simulink model "Robust_joint_Space"  (R2020b)
settings: Solver=VariableStepAuto  StartTime=0.0  StopTime=10  RelTol=1e-3
(part 5 of 7)

== matlab function Robust_joint_Space/robust inverse dynamic controller/v_hat_prod ==
  data: m input; theta input; Vhat output; thetad input
function Vhat = Find_V(m,theta,thetad)

m1 = m(1);
m2 = m(2);
m3 = m(3);
m4 = m(4);
m5 = m(5);
m6 = m(6);

t1=theta(1);
t2=theta(2);
t3=theta(3);
t4=theta(4);
t5=theta(5);
t6=theta(6);

td1=thetad(1);
td2=thetad(2);
td3=thetad(3);
td4=thetad(4);
td5=thetad(5);
td6=thetad(6);

L1=0.1025;
L2=0.408;
L3=0.376;
L4=0.1025; 
L5=0.1025;

Vhat = [td2*(td2*(0.1046752610416666598360663220646*cos(t1)*sin(t1) - 0.10662220333333332668301896006824*cos(t1)*cos(t2)^2*sin(t1) + 0.0058654583333333336347958919532175*cos(t1)*cos(t3)^2*sin(t1) - 0.0029327291666666668173979459766088*cos(t1)^2*cos(t3)*sin(t3) + 0.0029327291666666668173979459766088*cos(t3)*sin(t1)^2*sin(t3) + 19740.25*m2*cos(t1)*sin(t1) - 0.25*L2^2*m2*cos(t1)*sin(t1) - 70.25*L2*m2*cos(t1)^2*sin(t2) + 70.25*L2*m2*sin(t1)^2*sin(t2) + 0.25*L2^2*m2*cos(t1)*cos(t2)^2*sin(t1)) - 1.0*td5*(0.00036659114583333335217474324707609*sin(3.0*t2 - 1.0*t1 + t3 + t4) + 0.00073318229166666670434948649415219*sin(t2 - 2.0*t1 + 3.0*t3 + t4) + 0.00018329557291666667608737162353805*sin(3.0*t2 - 2.0*t1 + t3 + t4) + 0.00018329557291666667608737162353805*sin(2.0*t1 + 3.0*t2 + t3 + t4) + 0.00073318229166666670434948649415219*sin(t2 + t3 + t4) + 0.00036659114583333335217474324707609*sin(t1 - 1.0*t2 + t3 + t4) - 0.00057664973958333336527190549070099*sin(t2 - 2.0*t1 + t3 + t4) - 0.00057664973958333336527190549070099*sin(2.0*t1 + t2 + t3 + t4) + 0.00036659114583333335217474324707609*sin(t1 + 3.0*t2 + t3 + t4) - 0.00018329557291666667608737162353805*sin(2.0*t1 + t2 - 1.0*t3 - 1.0*t4) + 0.00036659114583333335217474324707609*sin(t3 - 1.0*t2 + t4) - 0.00036659114583333335217474324707609*sin(t1 + t2 - 1.0*t3 - 1.0*t4) + 0.00073318229166666670434948649415219*sin(2.0*t1 + t2 - 1.0*t3 + t4) + 0.00018329557291666667608737162353805*sin(2.0*t1 - 1.0*t2 + t3 + t4) - 0.0010997734375000000565242297412283*sin(3.0*t2 + t3 + t4) + 94.0*L3*m5*sin(t2 + t3 + t5) - 25.625*L3*m5*sin(t2 + t3 + t4 - 1.0*t5) - 102.0*L3*m5*sin(t2 - 1.0*t5) + 0.125*L3^2*m5*sin(t2 + t3 + t4) - 0.0625*L3^2*m5*sin(t2 + t3 + t4 - 2.0*t5) - 0.0625*L3^2*m5*sin(t2 + t3 + t4 + 2.0*t5) + 25.625*L3*m5*sin(t2 + t3 + t4 + t5) + 102.0*L3*m5*sin(t2 + t5) - 94.0*L3*m5*sin(t2 + t3 - 1.0*t5) - 0.25*L3*L4*m5*sin(t2 + t3 + t4 + t5) + 0.25*L3*L4*m5*sin(t2 + t3 + t4 - 1.0*t5)) - 1.0*td6*(0.00084023437500000005238864897449957*cos(t1)*cos(t5)*sin(t1) + 0.00042011718750000002619432448724979*cos(t1)^2*cos(t2)*cos(t3)*cos(t4)*sin(t5) - 0.00042011718750000002619432448724979*cos(t2)*cos(t3)*cos(t4)*sin(t1)^2*sin(t5) - 0.00042011718750000002619432448724979*cos(t1)^2*cos(t2)*sin(t3)*sin(t4)*sin(t5) - 0.00042011718750000002619432448724979*cos(t1)^2*cos(t3)*sin(t2)*sin(t4)*sin(t5) - 0.00042011718750000002619432448724979*cos(t1)^2*cos(t4)*sin(t2)*sin(t3)*sin(t5) + 0.00042011718750000002619432448724979*cos(t2)*sin(t1)^2*sin(t3)*sin(t4)*sin(t5) + 0.00042011718750000002619432448724979*cos(t3)*sin(t1)^2*sin(t2)*sin(t4)*sin(t5) + 0.00042011718750000002619432448724979*cos(t4)*sin(t1)^2*sin(t2)*sin(t3)*sin(t5)) + td4*(0.00073318229166666670434948649415219*sin(t1 - 2.0*t2) + 0.00073318229166666670434948649415219*sin(t1 + 2.0*t2) - 0.001153299479166666730543810981402*sin(2.0*t1) + 0.00036659114583333335217474324707609*sin(2.0*t1 - 2.0*t2) + 0.00036659114583333335217474324707609*sin(2.0*t1 + 2.0*t2) + 0.0014663645833333334086989729883044*sin(2.0*t1 - 2.0*t3)) + td3*(0.00073318229166666670434948649415219*sin(t1 - 2.0*t2) + 0.00073318229166666670434948649415219*sin(t1 + 2.0*t2) - 0.00024028885416666671912683250766918*sin(2.0*t1) + 0.00036659114583333335217474324707609*sin(2.0*t1 - 2.0*t2) + 0.00036659114583333335217474324707609*sin(2.0*t1 + 2.0*t2) + 0.0014663645833333334086989729883044*sin(2.0*t1 - 2.0*t3)) + td1*(153408.0*m4*sin(2.0*t2 + t3) - 0.053311101666666663341509480034119*sin(2.0*t2) + 153408.0*m5*sin(2.0*t2 + t3) + 153408.0*m6*sin(2.0*t2 + t3) + 38540.0*m5*sin(2.0*t2 + 2.0*t3 + t4) + 38540.0*m6*sin(2.0*t2 + 2.0*t3 + t4) + 83232.0*m3*sin(2.0*t2) + 83232.0*m4*sin(2.0*t2) + 83232.0*m5*sin(2.0*t2) + 83232.0*m6*sin(2.0*t2) + 41820.0*m5*sin(2.0*t2 + t3 + t4) + 41820.0*m6*sin(2.0*t2 + t3 + t4) + 70688.0*m4*sin(2.0*t2 + 2.0*t3) + 70688.0*m5*sin(2.0*t2 + 2.0*t3) + 70688.0*m6*sin(2.0*t2 + 2.0*t3) + 5253.125*m5*sin(2.0*t2 + 2.0*t3 + 2.0*t4) + 5253.125*m6*sin(2.0*t2 + 2.0*t3 + 2.0*t4) - 102.5*L4*m5*sin(2.0*t2 + 2.0*t3 + 2.0*t4) + 25.625*L3*m5*sin(2.0*t2 + 2.0*t3 + 2.0*t4 - 1.0*t5) - 102.0*L3*m5*sin(2.0*t2 + t3 + t4 + t5) - 0.0625*L3^2*m5*sin(2.0*t2 + 2.0*t3 + 2.0*t4) + 0.5*L4^2*m5*sin(2.0*t2 + 2.0*t3 + 2.0*t4) - 376.0*L4*m5*sin(2.0*t2 + 2.0*t3 + t4) + 0.03125*L3^2*m5*sin(2.0*t2 + 2.0*t3 + 2.0*t4 - 2.0*t5) + 0.03125*L3^2*m5*sin(2.0*t2 + 2.0*t3 + 2.0*t4 + 2.0*t5) + 94.0*L3*m5*sin(2.0*t2 + 2.0*t3 + t4 - 1.0*t5) - 25.625*L3*m5*sin(2.0*t2 + 2.0*t3 + 2.0*t4 + t5) - 408.0*L4*m5*sin(2.0*t2 + t3 + t4) + 102.0*L3*m5*sin(2.0*t2 + t3 + t4 - 1.0*t5) - 94.0*L3*m5*sin(2.0*t2 + 2.0*t3 + t4 + t5) + 0.125*L2^2*m2*sin(2.0*t2) - 0.25*L3*L4*m5*sin(2.0*t2 + 2.0*t3 + 2.0*t4 - 1.0*t5) + 0.25*L3*L4*m5*sin(2.0*t2 + 2.0*t3 + 2.0*t4 + t5))) - td6*(td6*(0.5*(0.00084023437500000005238864897449957*cos(t1)*cos(t5) - 0.00084023437500000005238864897449957*cos(t2)*cos(t3)*cos(t4)*sin(t1)*sin(t5) + 0.00084023437500000005238864897449957*cos(t2)*sin(t1)*sin(t3)*sin(t4)*sin(t5) + 0.00084023437500000005238864897449957*cos(t3)*sin(t1)*sin(t2)*sin(t4)*sin(t5) + 0.00084023437500000005238864897449957*cos(t4)*sin(t1)*sin(t2)*sin(t3)*sin(t5))*(cos(t1)*cos(t2)*sin(t3)*sin(t4)*sin(t5) - 1.0*cos(t1)*cos(t2)*cos(t3)*cos(t4)*sin(t5) - 1.0*cos(t5)*sin(t1) + cos(t1)*cos(t3)*sin(t2)*sin(t4)*sin(t5) + cos(t1)*cos(t4)*sin(t2)*sin(t3)*sin(t5)) - 0.5*(0.0016804687500000001047772979489991*cos(t1)*cos(t5) - 0.0016804687500000001047772979489991*cos(t2)*cos(t3)*cos(t4)*sin(t1)*sin(t5) + 0.0016804687500000001047772979489991*cos(t2)*sin(t1)*sin(t3)*sin(t4)*sin(t5) + 0.0016804687500000001047772979489991*cos(t3)*sin(t1)*sin(t2)*sin(t4)*sin(t5) + 0.0016804687500000001047772979489991*cos(t4)*sin(t1)*sin(t2)*sin(t3)*sin(t5))*(cos(t1)*cos(t2)*sin(t3)*sin(t4)*sin(t5) - 1.0*cos(t1)*cos(t2)*cos(t3)*cos(t4)*sin(t5) - 1.0*cos(t5)*sin(t1) + cos(t1)*cos(t3)*sin(t2)*sin(t4)*sin(t5) + cos(t1)*cos(t4)*sin(t2)*sin(t3)*sin(t5)) + 0.5*(0.00084023437500000005238864897449957*cos(t1)*cos(t2)*sin(t3)*sin(t4)*sin(t5) - 0.00084023437500000005238864897449957*cos(t1)*cos(t2)*cos(t3)*cos(t4)*sin(t5) - 0.00084023437500000005238864897449957*cos(t5)*sin(t1) + 0.00084023437500000005238864897449957*cos(t1)*cos(t3)*sin(t2)*sin(t4)*sin(t5) + 0.00084023437500000005238864897449957*cos(t1)*cos(t4)*sin(t2)*sin(t3)*sin(t5))*(cos(t1)*cos(t5) - 1.0*cos(t2)*cos(t3)*cos(t4)*sin(t1)*sin(t5) + cos(t2)*sin(t1)*sin(t3)*sin(t4)*sin(t5) + cos(t3)*sin(t1)*sin(t2)*sin(t4)*sin(t5) + cos(t4)*sin(t1)*sin(t2)*sin(t3)*sin(t5)) - 0.5*(0.0016804687500000001047772979489991*cos(t1)*cos(t2)*sin(t3)*sin(t4)*sin(t5) - 0.0016804687500000001047772979489991*cos(t1)*cos(t2)*cos(t3)*cos(t4)*sin(t5) - 0.0016804687500000001047772979489991*cos(t5)*sin(t1) + 0.0016804687500000001047772979489991*cos(t1)*cos(t3)*sin(t2)*sin(t4)*sin(t5) + 0.0016804687500000001047772979489991*cos(t1)*cos(t4)*sin(t2)*sin(t3)*sin(t5))*(cos(t1)*cos(t5) - 1.0*cos(t2)*cos(t3)*cos(t4)*sin(t1)*sin(t5) + cos(t2)*sin(t1)*sin(t3)*sin(t4)*sin(t5) + cos(t3)*sin(t1)*sin(t2)*sin(t4)*sin(t5) + cos(t4)*sin(t1)*sin(t2)*sin(t3)*sin(t5))) + 1.0*td2*(0.00084023437500000005238864897449957*cos(t1)*cos(t5)*sin(t1) + 0.00042011718750000002619432448724979*cos(t1)^2*cos(t2)*cos(t3)*cos(t4)*sin(t5) - 0.00042011718750000002619432448724979*cos(t2)*cos(t3)*cos(t4)*sin(t1)^2*sin(t5) - 0.00042011718750000002619432448724979*cos(t1)^2*cos(t2)*sin(t3)*sin(t4)*sin(t5) - 0.00042011718750000002619432448724979*cos(t1)^2*cos(t3)*sin(t2)*sin(t4)*sin(t5) - 0.00042011718750000002619432448724979*cos(t1)^2*cos(t4)*sin(t2)*sin(t3)*sin(t5) + 0.00042011718750000002619432448724979*cos(t2)*sin(t1)^2*sin(t3)*sin(t4)*sin(t5) + 0.00042011718750000002619432448724979*cos(t3)*sin(t1)^2*sin(t2)*sin(t4)*sin(t5) + 0.00042011718750000002619432448724979*cos(t4)*sin(t1)^2*sin(t2)*sin(t3)*sin(t5)) + 1.0*td3*(0.00084023437500000005238864897449957*cos(t1)*cos(t5)*sin(t1) + 0.00042011718750000002619432448724979*cos(t1)^2*cos(t2)*cos(t3)*cos(t4)*sin(t5) - 0.00042011718750000002619432448724979*cos(t2)*cos(t3)*cos(t4)*sin(t1)^2*sin(t5) - 0.00042011718750000002619432448724979*cos(t1)^2*cos(t2)*sin(t3)*sin(t4)*sin(t5) - 0.00042011718750000002619432448724979*cos(t1)^2*cos(t3)*sin(t2)*sin(t4)*sin(t5) - 0.00042011718750000002619432448724979*cos(t1)^2*cos(t4)*sin(t2)*sin(t3)*sin(t5) + 0.00042011718750000002619432448724979*cos(t2)*sin(t1)^2*sin(t3)*sin(t4)*sin(t5) + 0.00042011718750000002619432448724979*cos(t3)*sin(t1)^2*sin(t2)*sin(t4)*sin(t5) + 0.00042011718750000002619432448724979*cos(t4)*sin(t1)^2*sin(t2)*sin(t3)*sin(t5)) + 1.0*td4*(0.00084023437500000005238864897449957*cos(t1)*cos(t5)*sin(t1) + 0.00042011718750000002619432448724979*cos(t1)^2*cos(t2)*cos(t3)*cos(t4)*sin(t5) - 0.00042011718750000002619432448724979*cos(t2)*cos(t3)*cos(t4)*sin(t1)^2*sin(t5) - 0.00042011718750000002619432448724979*cos(t1)^2*cos(t2)*sin(t3)*sin(t4)*sin(t5) - 0.00042011718750000002619432448724979*cos(t1)^2*cos(t3)*sin(t2)*sin(t4)*sin(t5) - 0.00042011718750000002619432448724979*cos(t1)^2*cos(t4)*sin(t2)*sin(t3)*sin(t5) + 0.00042011718750000002619432448724979*cos(t2)*sin(t1)^2*sin(t3)*sin(t4)*sin(t5) + 0.00042011718750000002619432448724979*cos(t3)*sin(t1)^2*sin(t2)*sin(t4)*sin(t5) + 0.00042011718750000002619432448724979*cos(t4)*sin(t1)^2*sin(t2)*sin(t3)*sin(t5)) + td5*(0.00021005859375000001309716224362489*cos(2.0*t2)*cos(2.0*t3)*sin(2.0*t1)*sin(2.0*t4)*sin(t5) + 0.00021005859375000001309716224362489*cos(2.0*t2)*cos(2.0*t4)*sin(2.0*t1)*sin(2.0*t3)*sin(t5) + 0.00021005859375000001309716224362489*cos(2.0*t3)*cos(2.0*t4)*sin(2.0*t1)*sin(2.0*t2)*sin(t5) - 0.00042011718750000002619432448724979*cos(2.0*t1)*cos(t2)*cos(t3)*cos(t5)*sin(t4) - 0.00042011718750000002619432448724979*cos(2.0*t1)*cos(t2)*cos(t4)*cos(t5)*sin(t3) - 0.00042011718750000002619432448724979*cos(2.0*t1)*cos(t3)*cos(t4)*cos(t5)*sin(t2) - 0.00021005859375000001309716224362489*sin(2.0*t1)*sin(2.0*t2)*sin(2.0*t3)*sin(2.0*t4)*sin(t5) + 0.00042011718750000002619432448724979*cos(2.0*t1)*cos(t5)*sin(t2)*sin(t3)*sin(t4))) - td3*(1.0*td6*(0.00084023437500000005238864897449957*cos(t1)*cos(t5)*sin(t1) + 0.00042011718750000002619432448724979*cos(t1)^2*cos(t2)*cos(t3)*cos(t4)*sin(t5) - 0.00042011718750000002619432448724979*cos(t2)*cos(t3)*cos(t4)*sin(t1)^2*sin(t5) - 0.00042011718750000002619432448724979*cos(t1)^2*cos(t2)*sin(t3)*sin(t4)*sin(t5) - 0.00042011718750000002619432448724979*cos(t1)^2*cos(t3)*sin(t2)*sin(t4)*sin(t5) - 0.00042011718750000002619432448724979*cos(t1)^2*cos(t4)*sin(t2)*sin(t3)*sin(t5) + 0.00042011718750000002619432448724979*cos(t2)*sin(t1)^2*sin(t3)*sin(t4)*sin(t5) + 0.00042011718750000002619432448724979*cos(t3)*sin(t1)^2*sin(t2)*sin(t4)*sin(t5) + 0.00042011718750000002619432448724979*cos(t4)*sin(t1)^2*sin(t2)*sin(t3)*sin(t5)) - td3*(- 0.0029327291666666668173979459766088*sin(t3)*cos(t1)^2*cos(t3) + 0.0029327291666666668173979459766088*cos(t1)*cos(t2)^2*sin(t1) + 0.0058654583333333336347958919532175*cos(t1)*cos(t3)^2*sin(t1) - 0.0048796714583333336643505839802515*cos(t1)*sin(t1) + 0.0029327291666666668173979459766088*sin(t3)*cos(t3)*sin(t1)^2) - td4*(- 0.0029327291666666668173979459766088*sin(t3)*cos(t1)^2*cos(t3) + 0.0029327291666666668173979459766088*cos(t1)*cos(t2)^2*sin(t1) + 0.0058654583333333336347958919532175*cos(t1)*cos(t3)^2*sin(t1) - 0.0067056927083333336871845409277171*cos(t1)*sin(t1) + 0.0029327291666666668173979459766088*sin(t3)*cos(t3)*sin(t1)^2) - td1*(76704.0*m4*sin(2.0*t2 + t3) + 76704.0*m5*sin(2.0*t2 + t3) + 76704.0*m6*sin(2.0*t2 + t3) + 38540.0*m5*sin(2.0*t2 + 2.0*t3 + t4) + 38540.0*m6*sin(2.0*t2 + 2.0*t3 + t4) - 20910.0*m5*sin(t3 + t4) - 20910.0*m6*sin(t3 + t4) + 20910.0*m5*sin(2.0*t2 + t3 + t4) + 20910.0*m6*sin(2.0*t2 + t3 + t4) - 76704.0*m4*sin(t3) - 76704.0*m5*sin(t3) - 76704.0*m6*sin(t3) + 70688.0*m4*sin(2.0*t2 + 2.0*t3) + 70688.0*m5*sin(2.0*t2 + 2.0*t3) + 70688.0*m6*sin(2.0*t2 + 2.0*t3) + 5253.125*m5*sin(2.0*t2 + 2.0*t3 + 2.0*t4) + 5253.125*m6*sin(2.0*t2 + 2.0*t3 + 2.0*t4) - 102.5*L4*m5*sin(2.0*t2 + 2.0*t3 + 2.0*t4) + 25.625*L3*m5*sin(2.0*t2 + 2.0*t3 + 2.0*t4 - 1.0*t5) + 51.0*L3*m5*sin(t3 + t4 + t5) - 51.0*L3*m5*sin(2.0*t2 + t3 + t4 + t5) - 0.0625*L3^2*m5*sin(2.0*t2 + 2.0*t3 + 2.0*t4) + 0.5*L4^2*m5*sin(2.0*t2 + 2.0*t3 + 2.0*t4) - 376.0*L4*m5*sin(2.0*t2 + 2.0*t3 + t4) + 0.03125*L3^2*m5*sin(2.0*t2 + 2.0*t3 + 2.0*t4 - 2.0*t5) + 0.03125*L3^2*m5*sin(2.0*t2 + 2.0*t3 + 2.0*t4 + 2.0*t5) + 94.0*L3*m5*sin(2.0*t2 + 2.0*t3 + t4 - 1.0*t5) - 25.625*L3*m5*sin(2.0*t2 + 2.0*t3 + 2.0*t4 + t5) + 204.0*L4*m5*sin(t3 + t4) - 204.0*L4*m5*sin(2.0*t2 + t3 + t4) - 51.0*L3*m5*sin(t3 + t4 - 1.0*t5) + 51.0*L3*m5*sin(2.0*t2 + t3 + t4 - 1.0*t5) - 94.0*L3*m5*sin(2.0*t2 + 2.0*t3 + t4 + t5) - 0.25*L3*L4*m5*sin(2.0*t2 + 2.0*t3 + 2.0*t4 - 1.0*t5) + 0.25*L3*L4*m5*sin(2.0*t2 + 2.0*t3 + 2.0*t4 + t5)) + td5*(0.00073318229166666670434948649415219*sin(t2 - 2.0*t1 + 3.0*t3 + t4) + 0.00018329557291666667608737162353805*sin(3.0*t2 - 2.0*t1 + t3 + t4) + 0.00018329557291666667608737162353805*sin(2.0*t1 + 3.0*t2 + t3 + t4) + 0.00073318229166666670434948649415219*sin(t2 + t3 + t4) - 0.00057664973958333336527190549070099*sin(t2 - 2.0*t1 + t3 + t4) - 0.00057664973958333336527190549070099*sin(2.0*t1 + t2 + t3 + t4) - 0.00018329557291666667608737162353805*sin(2.0*t1 + t2 - 1.0*t3 - 1.0*t4) - 0.00036659114583333335217474324707609*sin(t3 - 1.0*t2 + t4) + 0.00073318229166666670434948649415219*sin(2.0*t1 + t2 - 1.0*t3 + t4) + 0.00018329557291666667608737162353805*sin(2.0*t1 - 1.0*t2 + t3 + t4) - 0.00036659114583333335217474324707609*sin(3.0*t2 + t3 + t4) + 94.0*L3*m5*sin(t2 + t3 + t5) - 25.625*L3*m5*sin(t2 + t3 + t4 - 1.0*t5) + 0.125*L3^2*m5*sin(t2 + t3 + t4) - 0.0625*L3^2*m5*sin(t2 + t3 + t4 - 2.0*t5) - 0.0625*L3^2*m5*sin(t2 + t3 + t4 + 2.0*t5) + 25.625*L3*m5*sin(t2 + t3 + t4 + t5) - 94.0*L3*m5*sin(t2 + t3 - 1.0*t5) - 0.25*L3*L4*m5*sin(t2 + t3 + t4 + t5) + 0.25*L3*L4*m5*sin(t2 + t3 + t4 - 1.0*t5)) + 1.0*td2*(0.00073318229166666670434948649415219*sin(t1 - 2.0*t2) + 0.00073318229166666670434948649415219*sin(t1 + 2.0*t2) + 0.00024028885416666671912683250766918*sin(2.0*t1) - 0.00036659114583333335217474324707609*sin(2.0*t1 - 2.0*t2) - 0.00036659114583333335217474324707609*sin(2.0*t1 + 2.0*t2) - 0.0014663645833333334086989729883044*sin(2.0*t1 - 2.0*t3))) - td5*(1.0*td5*(0.00018329557291666667608737162353805*sin(2.0*t3 - 1.0*t1 + 2.0*t4) - 0.00036659114583333335217474324707609*sin(2.0*t1 + 2.0*t2 + 2.0*t4) + 0.000091647786458333338043685811769024*sin(2.0*t3 - 2.0*t1 + 2.0*t4) - 0.000091647786458333338043685811769024*sin(2.0*t1 + 2.0*t3 + 2.0*t4) - 0.00018329557291666667608737162353805*sin(4.0*t2 - 1.0*t1 + 2.0*t3 + 2.0*t4) - 0.00028832486979166668263595274535049*sin(2.0*t2 - 2.0*t1 + 2.0*t3 + 2.0*t4) + 0.00028832486979166668263595274535049*sin(2.0*t1 + 2.0*t2 + 2.0*t3 + 2.0*t4) + 0.00036659114583333335217474324707609*sin(2.0*t2 - 2.0*t1 + 4.0*t3 + 2.0*t4) + 0.000091647786458333338043685811769024*sin(4.0*t2 - 2.0*t1 + 2.0*t3 + 2.0*t4) - 0.000091647786458333338043685811769024*sin(2.0*t1 + 4.0*t2 + 2.0*t3 + 2.0*t4) - 0.00018329557291666667608737162353805*sin(t1 + 2.0*t3 + 2.0*t4) + 0.00018329557291666667608737162353805*sin(t1 + 4.0*t2 + 2.0*t3 + 2.0*t4) - 0.00057664973958333336527190549070099*sin(2.0*t1) + 0.00018329557291666667608737162353805*sin(2.0*t1 - 2.0*t2) + 0.00018329557291666667608737162353805*sin(2.0*t1 + 2.0*t2) + 0.00073318229166666670434948649415219*sin(2.0*t1 - 2.0*t3)) + 1.0*td3*(0.00073318229166666670434948649415219*sin(t2 - 2.0*t1 + 3.0*t3 + t4) - 0.00036659114583333335217474324707609*sin(3.0*t2 - 1.0*t1 + t3 + t4) + 0.00018329557291666667608737162353805*sin(3.0*t2 - 2.0*t1 + t3 + t4) + 0.00018329557291666667608737162353805*sin(2.0*t1 + 3.0*t2 + t3 + t4) - 0.00073318229166666670434948649415219*sin(t2 + t3 + t4) + 0.00036659114583333335217474324707609*sin(t1 - 1.0*t2 + t3 + t4) - 0.00057664973958333336527190549070099*sin(t2 - 2.0*t1 + t3 + t4) - 0.00057664973958333336527190549070099*sin(2.0*t1 + t2 + t3 + t4) - 0.00036659114583333335217474324707609*sin(t1 + 3.0*t2 + t3 + t4) - 0.00018329557291666667608737162353805*sin(2.0*t1 + t2 - 1.0*t3 - 1.0*t4) + 0.00036659114583333335217474324707609*sin(t3 - 1.0*t2 + t4) - 0.00036659114583333335217474324707609*sin(t1 + t2 - 1.0*t3 - 1.0*t4) + 0.00073318229166666670434948649415219*sin(2.0*t1 + t2 - 1.0*t3 + t4) + 0.00018329557291666667608737162353805*sin(2.0*t1 - 1.0*t2 + t3 + t4) + 0.00036659114583333335217474324707609*sin(3.0*t2 + t3 + t4) - 94.0*L3*m5*sin(t2 + t3 + t5) + 25.625*L3*m5*sin(t2 + t3 + t4 - 1.0*t5) - 0.125*L3^2*m5*sin(t2 + t3 + t4) + 0.0625*L3^2*m5*sin(t2 + t3 + t4 - 2.0*t5) + 0.0625*L3^2*m5*sin(t2 + t3 + t4 + 2.0*t5) - 25.625*L3*m5*sin(t2 + t3 + t4 + t5) + 94.0*L3*m5*sin(t2 + t3 - 1.0*t5) + 0.25*L3*L4*m5*sin(t2 + t3 + t4 + t5) - 0.25*L3*L4*m5*sin(t2 + t3 + t4 - 1.0*t5)) + 1.0*td1*(12.8125*L3*m5*sin(2.0*t2 + 2.0*t3 + 2.0*t4 - 1.0*t5) - 51.0*L3*m5*sin(t3 + t4 + t5) + 51.0*L3*m5*sin(2.0*t2 + t3 + t4 + t5) - 47.0*L3*m5*sin(t4 - 1.0*t5) + 0.03125*L3^2*m5*sin(2.0*t2 + 2.0*t3 + 2.0*t4 - 2.0*t5) - 0.03125*L3^2*m5*sin(2.0*t2 + 2.0*t3 + 2.0*t4 + 2.0*t5) + 47.0*L3*m5*sin(2.0*t2 + 2.0*t3 + t4 - 1.0*t5) + 12.8125*L3*m5*sin(2.0*t2 + 2.0*t3 + 2.0*t4 + t5) - 47.0*L3*m5*sin(t4 + t5) - 51.0*L3*m5*sin(t3 + t4 - 1.0*t5) + 51.0*L3*m5*sin(2.0*t2 + t3 + t4 - 1.0*t5) + 47.0*L3*m5*sin(2.0*t2 + 2.0*t3 + t4 + t5) + 0.0625*L3^2*m5*sin(2.0*t5) + 70.25*L3*m5*sin(t5) - 0.125*L3*L4*m5*sin(2.0*t2 + 2.0*t3 + 2.0*t4 - 1.0*t5) - 0.125*L3*L4*m5*sin(2.0*t2 + 2.0*t3 + 2.0*t4 + t5)) + 1.0*td4*(0.00073318229166666670434948649415219*sin(t2 - 2.0*t1 + 3.0*t3 + t4) - 0.00036659114583333335217474324707609*sin(3.0*t2 - 1.0*t1 + t3 + t4) + 0.00018329557291666667608737162353805*sin(3.0*t2 - 2.0*t1 + t3 + t4) + 0.00018329557291666667608737162353805*sin(2.0*t1 + 3.0*t2 + t3 + t4) - 0.00073318229166666670434948649415219*sin(t2 + t3 + t4) + 0.00036659114583333335217474324707609*sin(t1 - 1.0*t2 + t3 + t4) - 0.00057664973958333336527190549070099*sin(t2 - 2.0*t1 + t3 + t4) - 0.00057664973958333336527190549070099*sin(2.0*t1 + t2 + t3 + t4) - 0.00036659114583333335217474324707609*sin(t1 + 3.0*t2 + t3 + t4) - 0.00018329557291666667608737162353805*sin(2.0*t1 + t2 - 1.0*t3 - 1.0*t4) + 0.00036659114583333335217474324707609*sin(t3 - 1.0*t2 + t4) - 0.00036659114583333335217474324707609*sin(t1 + t2 - 1.0*t3 - 1.0*t4) + 0.00073318229166666670434948649415219*sin(2.0*t1 + t2 - 1.0*t3 + t4) + 0.00018329557291666667608737162353805*sin(2.0*t1 - 1.0*t2 + t3 + t4) + 0.00036659114583333335217474324707609*sin(3.0*t2 + t3 + t4) + 25.625*L3*m5*sin(t2 + t3 + t4 - 1.0*t5) - 0.125*L3^2*m5*sin(t2 + t3 + t4) + 0.0625*L3^2*m5*sin(t2 + t3 + t4 - 2.0*t5) + 0.0625*L3^2*m5*sin(t2 + t3 + t4 + 2.0*t5) - 25.625*L3*m5*sin(t2 + t3 + t4 + t5) + 0.25*L3*L4*m5*sin(t2 + t3 + t4 + t5) - 0.25*L3*L4*m5*sin(t2 + t3 + t4 - 1.0*t5)) - td2*(0.00073318229166666670434948649415219*sin(3.0*t2 - 1.0*t1 + t3 + t4) - 0.00073318229166666670434948649415219*sin(t2 - 2.0*t1 + 3.0*t3 + t4) - 0.00018329557291666667608737162353805*sin(3.0*t2 - 2.0*t1 + t3 + t4) - 0.00018329557291666667608737162353805*sin(2.0*t1 + 3.0*t2 + t3 + t4) + 0.00073318229166666670434948649415219*sin(t2 + t3 + t4) + 0.00057664973958333336527190549070099*sin(t2 - 2.0*t1 + t3 + t4) + 0.00057664973958333336527190549070099*sin(2.0*t1 + t2 + t3 + t4) + 0.00073318229166666670434948649415219*sin(t1 + 3.0*t2 + t3 + t4) + 0.00018329557291666667608737162353805*sin(2.0*t1 + t2 - 1.0*t3 - 1.0*t4) + 0.00036659114583333335217474324707609*sin(t3 - 1.0*t2 + t4) - 0.00073318229166666670434948649415219*sin(2.0*t1 + t2 - 1.0*t3 + t4) - 0.00018329557291666667608737162353805*sin(2.0*t1 - 1.0*t2 + t3 + t4) - 0.0010997734375000000565242297412283*sin(3.0*t2 + t3 + t4) + 94.0*L3*m5*sin(t2 + t3 + t5) - 25.625*L3*m5*sin(t2 + t3 + t4 - 1.0*t5) - 102.0*L3*m5*sin(t2 - 1.0*t5) + 0.125*L3^2*m5*sin(t2 + t3 + t4) - 0.0625*L3^2*m5*sin(t2 + t3 + t4 - 2.0*t5) - 0.0625*L3^2*m5*sin(t2 + t3 + t4 + 2.0*t5) + 25.625*L3*m5*sin(t2 + t3 + t4 + t5) + 102.0*L3*m5*sin(t2 + t5) - 94.0*L3*m5*sin(t2 + t3 - 1.0*t5) - 0.25*L3*L4*m5*sin(t2 + t3 + t4 + t5) + 0.25*L3*L4*m5*sin(t2 + t3 + t4 - 1.0*t5)) + td6*(0.00021005859375000001309716224362489*cos(2.0*t2)*cos(2.0*t3)*sin(2.0*t1)*sin(2.0*t4)*sin(t5) + 0.00021005859375000001309716224362489*cos(2.0*t2)*cos(2.0*t4)*sin(2.0*t1)*sin(2.0*t3)*sin(t5) + 0.00021005859375000001309716224362489*cos(2.0*t3)*cos(2.0*t4)*sin(2.0*t1)*sin(2.0*t2)*sin(t5) - 0.00042011718750000002619432448724979*cos(2.0*t1)*cos(t2)*cos(t3)*cos(t5)*sin(t4) - 0.00042011718750000002619432448724979*cos(2.0*t1)*cos(t2)*cos(t4)*cos(t5)*sin(t3) - 0.00042011718750000002619432448724979*cos(2.0*t1)*cos(t3)*cos(t4)*cos(t5)*sin(t2) - 0.00021005859375000001309716224362489*sin(2.0*t1)*sin(2.0*t2)*sin(2.0*t3)*sin(2.0*t4)*sin(t5) + 0.00042011718750000002619432448724979*cos(2.0*t1)*cos(t5)*sin(t2)*sin(t3)*sin(t4))) - td4*(1.0*td6*(0.00084023437500000005238864897449957*cos(t1)*cos(t5)*sin(t1) + 0.00042011718750000002619432448724979*cos(t1)^2*cos(t2)*cos(t3)*cos(t4)*sin(t5) - 0.00042011718750000002619432448724979*cos(t2)*cos(t3)*cos(t4)*sin(t1)^2*sin(t5) - 0.00042011718750000002619432448724979*cos(t1)^2*cos(t2)*sin(t3)*sin(t4)*sin(t5) - 0.00042011718750000002619432448724979*cos(t1)^2*cos(t3)*sin(t2)*sin(t4)*sin(t5) - 0.00042011718750000002619432448724979*cos(t1)^2*cos(t4)*sin(t2)*sin(t3)*sin(t5) + 0.00042011718750000002619432448724979*cos(t2)*sin(t1)^2*sin(t3)*sin(t4)*sin(t5) + 0.00042011718750000002619432448724979*cos(t3)*sin(t1)^2*sin(t2)*sin(t4)*sin(t5) + 0.00042011718750000002619432448724979*cos(t4)*sin(t1)^2*sin(t2)*sin(t3)*sin(t5)) + 1.0*td4*(0.001153299479166666730543810981402*sin(2.0*t1) - 0.00073318229166666670434948649415219*cos(2.0*t2)*sin(2.0*t1) + 0.0014663645833333334086989729883044*cos(2.0*t1)*sin(2.0*t3) - 0.0014663645833333334086989729883044*cos(2.0*t3)*sin(2.0*t1)) - td1*(19270.0*m5*sin(2.0*t2 + 2.0*t3 + t4) + 19270.0*m6*sin(2.0*t2 + 2.0*t3 + t4) - 20910.0*m5*sin(t3 + t4) - 20910.0*m6*sin(t3 + t4) + 20910.0*m5*sin(2.0*t2 + t3 + t4) + 20910.0*m6*sin(2.0*t2 + t3 + t4) - 19270.0*m5*sin(t4) - 19270.0*m6*sin(t4) + 5253.125*m5*sin(2.0*t2 + 2.0*t3 + 2.0*t4) + 5253.125*m6*sin(2.0*t2 + 2.0*t3 + 2.0*t4) - 102.5*L4*m5*sin(2.0*t2 + 2.0*t3 + 2.0*t4) + 25.625*L3*m5*sin(2.0*t2 + 2.0*t3 + 2.0*t4 - 1.0*t5) + 51.0*L3*m5*sin(t3 + t4 + t5) - 51.0*L3*m5*sin(2.0*t2 + t3 + t4 + t5) - 47.0*L3*m5*sin(t4 - 1.0*t5) - 0.0625*L3^2*m5*sin(2.0*t2 + 2.0*t3 + 2.0*t4) + 0.5*L4^2*m5*sin(2.0*t2 + 2.0*t3 + 2.0*t4) - 188.0*L4*m5*sin(2.0*t2 + 2.0*t3 + t4) + 0.03125*L3^2*m5*sin(2.0*t2 + 2.0*t3 + 2.0*t4 - 2.0*t5) + 0.03125*L3^2*m5*sin(2.0*t2 + 2.0*t3 + 2.0*t4 + 2.0*t5) + 47.0*L3*m5*sin(2.0*t2 + 2.0*t3 + t4 - 1.0*t5) - 25.625*L3*m5*sin(2.0*t2 + 2.0*t3 + 2.0*t4 + t5) + 204.0*L4*m5*sin(t3 + t4) + 47.0*L3*m5*sin(t4 + t5) - 204.0*L4*m5*sin(2.0*t2 + t3 + t4) - 51.0*L3*m5*sin(t3 + t4 - 1.0*t5) + 51.0*L3*m5*sin(2.0*t2 + t3 + t4 - 1.0*t5) - 47.0*L3*m5*sin(2.0*t2 + 2.0*t3 + t4 + t5) + 188.0*L4*m5*sin(t4) - 0.25*L3*L4*m5*sin(2.0*t2 + 2.0*t3 + 2.0*t4 - 1.0*t5) + 0.25*L3*L4*m5*sin(2.0*t2 + 2.0*t3 + 2.0*t4 + t5)) - td3*(- 0.0029327291666666668173979459766088*sin(t3)*cos(t1)^2*cos(t3) + 0.0029327291666666668173979459766088*cos(t1)*cos(t2)^2*sin(t1) + 0.0058654583333333336347958919532175*cos(t1)*cos(t3)^2*sin(t1) - 0.0067056927083333336871845409277171*cos(t1)*sin(t1) + 0.0029327291666666668173979459766088*sin(t3)*cos(t3)*sin(t1)^2) + 1.0*td2*(0.00073318229166666670434948649415219*sin(t1 - 2.0*t2) + 0.00073318229166666670434948649415219*sin(t1 + 2.0*t2) + 0.001153299479166666730543810981402*sin(2.0*t1) - 0.00036659114583333335217474324707609*sin(2.0*t1 - 2.0*t2) - 0.00036659114583333335217474324707609*sin(2.0*t1 + 2.0*t2) - 0.0014663645833333334086989729883044*sin(2.0*t1 - 2.0*t3)) + td5*(0.00073318229166666670434948649415219*sin(t2 - 2.0*t1 + 3.0*t3 + t4) + 0.00018329557291666667608737162353805*sin(3.0*t2 - 2.0*t1 + t3 + t4) + 0.00018329557291666667608737162353805*sin(2.0*t1 + 3.0*t2 + t3 + t4) + 0.00073318229166666670434948649415219*sin(t2 + t3 + t4) - 0.00057664973958333336527190549070099*sin(t2 - 2.0*t1 + t3 + t4) - 0.00057664973958333336527190549070099*sin(2.0*t1 + t2 + t3 + t4) - 0.00018329557291666667608737162353805*sin(2.0*t1 + t2 - 1.0*t3 - 1.0*t4) - 0.00036659114583333335217474324707609*sin(t3 - 1.0*t2 + t4) + 0.00073318229166666670434948649415219*sin(2.0*t1 + t2 - 1.0*t3 + t4) + 0.00018329557291666667608737162353805*sin(2.0*t1 - 1.0*t2 + t3 + t4) - 0.00036659114583333335217474324707609*sin(3.0*t2 + t3 + t4) - 25.625*L3*m5*sin(t2 + t3 + t4 - 1.0*t5) + 0.125*L3^2*m5*sin(t2 + t3 + t4) - 0.0625*L3^2*m5*sin(t2 + t3 + t4 - 2.0*t5) - 0.0625*L3^2*m5*sin(t2 + t3 + t4 + 2.0*t5) + 25.625*L3*m5*sin(t2 + t3 + t4 + t5) - 0.25*L3*L4*m5*sin(t2 + t3 + t4 + t5) + 0.25*L3*L4*m5*sin(t2 + t3 + t4 - 1.0*t5))) - td1*(1.0*td2*(0.02665555083333333167075474001706*sin(t1 + 2.0*t2) - 0.02665555083333333167075474001706*sin(t1 - 2.0*t2) - 0.053311101666666663341509480034119*sin(2.0*t2) + 153408.0*m4*sin(2.0*t2 + t3) + 153408.0*m5*sin(2.0*t2 + t3) + 153408.0*m6*sin(2.0*t2 + t3) + 38540.0*m5*sin(2.0*t2 + 2.0*t3 + t4) + 38540.0*m6*sin(2.0*t2 + 2.0*t3 + t4) + 83232.0*m3*sin(2.0*t2) + 83232.0*m4*sin(2.0*t2) + 83232.0*m5*sin(2.0*t2) + 83232.0*m6*sin(2.0*t2) + 41820.0*m5*sin(2.0*t2 + t3 + t4) + 41820.0*m6*sin(2.0*t2 + t3 + t4) + 70688.0*m4*sin(2.0*t2 + 2.0*t3) + 70688.0*m5*sin(2.0*t2 + 2.0*t3) + 70688.0*m6*sin(2.0*t2 + 2.0*t3) + 5253.125*m5*sin(2.0*t2 + 2.0*t3 + 2.0*t4) + 5253.125*m6*sin(2.0*t2 + 2.0*t3 + 2.0*t4) - 102.5*L4*m5*sin(2.0*t2 + 2.0*t3 + 2.0*t4) + 25.625*L3*m5*sin(2.0*t2 + 2.0*t3 + 2.0*t4 - 1.0*t5) - 102.0*L3*m5*sin(2.0*t2 + t3 + t4 + t5) - 35.125*L2*m2*sin(t1 - 1.0*t2) - 0.0625*L3^2*m5*sin(2.0*t2 + 2.0*t3 + 2.0*t4) + 0.5*L4^2*m5*sin(2.0*t2 + 2.0*t3 + 2.0*t4) - 376.0*L4*m5*sin(2.0*t2 + 2.0*t3 + t4) + 0.03125*L3^2*m5*sin(2.0*t2 + 2.0*t3 + 2.0*t4 - 2.0*t5) + 0.03125*L3^2*m5*sin(2.0*t2 + 2.0*t3 + 2.0*t4 + 2.0*t5) + 94.0*L3*m5*sin(2.0*t2 + 2.0*t3 + t4 - 1.0*t5) - 25.625*L3*m5*sin(2.0*t2 + 2.0*t3 + 2.0*t4 + t5) - 0.0625*L2^2*m2*sin(t1 - 2.0*t2) + 0.0625*L2^2*m2*sin(t1 + 2.0*t2) - 35.125*L2*m2*sin(t1 + t2) - 408.0*L4*m5*sin(2.0*t2 + t3 + t4) + 102.0*L3*m5*sin(2.0*t2 + t3 + t4 - 1.0*t5) - 94.0*L3*m5*sin(2.0*t2 + 2.0*t3 + t4 + t5) + 0.125*L2^2*m2*sin(2.0*t2) - 0.25*L3*L4*m5*sin(2.0*t2 + 2.0*t3 + 2.0*t4 - 1.0*t5) + 0.25*L3*L4*m5*sin(2.0*t2 + 2.0*t3 + 2.0*t4 + t5)) + 1.0*td4*(0.00073318229166666670434948649415219*sin(t1 - 2.0*t2) - 0.00073318229166666670434948649415219*sin(t1 + 2.0*t2) + 19270.0*m5*sin(2.0*t2 + 2.0*t3 + t4) + 19270.0*m6*sin(2.0*t2 + 2.0*t3 + t4) - 20910.0*m5*sin(t3 + t4) - 20910.0*m6*sin(t3 + t4) + 20910.0*m5*sin(2.0*t2 + t3 + t4) + 20910.0*m6*sin(2.0*t2 + t3 + t4) - 19270.0*m5*sin(t4) - 19270.0*m6*sin(t4) + 5253.125*m5*sin(2.0*t2 + 2.0*t3 + 2.0*t4) + 5253.125*m6*sin(2.0*t2 + 2.0*t3 + 2.0*t4) - 102.5*L4*m5*sin(2.0*t2 + 2.0*t3 + 2.0*t4) + 25.625*L3*m5*sin(2.0*t2 + 2.0*t3 + 2.0*t4 - 1.0*t5) + 51.0*L3*m5*sin(t3 + t4 + t5) - 51.0*L3*m5*sin(2.0*t2 + t3 + t4 + t5) - 47.0*L3*m5*sin(t4 - 1.0*t5) - 0.0625*L3^2*m5*sin(2.0*t2 + 2.0*t3 + 2.0*t4) + 0.5*L4^2*m5*sin(2.0*t2 + 2.0*t3 + 2.0*t4) - 188.0*L4*m5*sin(2.0*t2 + 2.0*t3 + t4) + 0.03125*L3^2*m5*sin(2.0*t2 + 2.0*t3 + 2.0*t4 - 2.0*t5) + 0.03125*L3^2*m5*sin(2.0*t2 + 2.0*t3 + 2.0*t4 + 2.0*t5) + 47.0*L3*m5*sin(2.0*t2 + 2.0*t3 + t4 - 1.0*t5) - 25.625*L3*m5*sin(2.0*t2 + 2.0*t3 + 2.0*t4 + t5) + 204.0*L4*m5*sin(t3 + t4) + 47.0*L3*m5*sin(t4 + t5) - 204.0*L4*m5*sin(2.0*t2 + t3 + t4) - 51.0*L3*m5*sin(t3 + t4 - 1.0*t5) + 51.0*L3*m5*sin(2.0*t2 + t3 + t4 - 1.0*t5) - 47.0*L3*m5*sin(2.0*t2 + 2.0*t3 + t4 + t5) + 188.0*L4*m5*sin(t4) - 0.25*L3*L4*m5*sin(2.0*t2 + 2.0*t3 + 2.0*t4 - 1.0*t5) + 0.25*L3*L4*m5*sin(2.0*t2 + 2.0*t3 + 2.0*t4 + t5)) - td5*(0.00036659114583333335217474324707609*sin(3.0*t2 - 1.0*t1 + t3 + t4) + 0.00036659114583333335217474324707609*sin(t1 - 1.0*t2 + t3 + t4) - 0.00036659114583333335217474324707609*sin(t1 + 3.0*t2 + t3 + t4) + 0.00036659114583333335217474324707609*sin(t1 + t2 - 1.0*t3 - 1.0*t4) + 12.8125*L3*m5*sin(2.0*t2 + 2.0*t3 + 2.0*t4 - 1.0*t5) - 51.0*L3*m5*sin(t3 + t4 + t5) + 51.0*L3*m5*sin(2.0*t2 + t3 + t4 + t5) - 47.0*L3*m5*sin(t4 - 1.0*t5) + 0.03125*L3^2*m5*sin(2.0*t2 + 2.0*t3 + 2.0*t4 - 2.0*t5) - 0.03125*L3^2*m5*sin(2.0*t2 + 2.0*t3 + 2.0*t4 + 2.0*t5) + 47.0*L3*m5*sin(2.0*t2 + 2.0*t3 + t4 - 1.0*t5) + 12.8125*L3*m5*sin(2.0*t2 + 2.0*t3 + 2.0*t4 + t5) - 47.0*L3*m5*sin(t4 + t5) - 51.0*L3*m5*sin(t3 + t4 - 1.0*t5) + 51.0*L3*m5*sin(2.0*t2 + t3 + t4 - 1.0*t5) + 47.0*L3*m5*sin(2.0*t2 + 2.0*t3 + t4 + t5) + 0.0625*L3^2*m5*sin(2.0*t5) + 70.25*L3*m5*sin(t5) - 0.125*L3*L4*m5*sin(2.0*t2 + 2.0*t3 + 2.0*t4 - 1.0*t5) - 0.125*L3*L4*m5*sin(2.0*t2 + 2.0*t3 + 2.0*t4 + t5)) + 1.0*td3*(0.00073318229166666670434948649415219*sin(t1 - 2.0*t2) - 0.00073318229166666670434948649415219*sin(t1 + 2.0*t2) + 76704.0*m4*sin(2.0*t2 + t3) + 76704.0*m5*sin(2.0*t2 + t3) + 76704.0*m6*sin(2.0*t2 + t3) + 38540.0*m5*sin(2.0*t2 + 2.0*t3 + t4) + 38540.0*m6*sin(2.0*t2 + 2.0*t3 + t4) - 20910.0*m5*sin(t3 + t4) - 20910.0*m6*sin(t3 + t4) + 20910.0*m5*sin(2.0*t2 + t3 + t4) + 20910.0*m6*sin(2.0*t2 + t3 + t4) - 76704.0*m4*sin(t3) - 76704.0*m5*sin(t3) - 76704.0*m6*sin(t3) + 70688.0*m4*sin(2.0*t2 + 2.0*t3) + 70688.0*m5*sin(2.0*t2 + 2.0*t3) + 70688.0*m6*sin(2.0*t2 + 2.0*t3) + 5253.125*m5*sin(2.0*t2 + 2.0*t3 + 2.0*t4) + 5253.125*m6*sin(2.0*t2 + 2.0*t3 + 2.0*t4) - 102.5*L4*m5*sin(2.0*t2 + 2.0*t3 + 2.0*t4) + 25.625*L3*m5*sin(2.0*t2 + 2.0*t3 + 2.0*t4 - 1.0*t5) + 51.0*L3*m5*sin(t3 + t4 + t5) - 51.0*L3*m5*sin(2.0*t2 + t3 + t4 + t5) - 0.0625*L3^2*m5*sin(2.0*t2 + 2.0*t3 + 2.0*t4) + 0.5*L4^2*m5*sin(2.0*t2 + 2.0*t3 + 2.0*t4) - 376.0*L4*m5*sin(2.0*t2 + 2.0*t3 + t4) + 0.03125*L3^2*m5*sin(2.0*t2 + 2.0*t3 + 2.0*t4 - 2.0*t5) + 0.03125*L3^2*m5*sin(2.0*t2 + 2.0*t3 + 2.0*t4 + 2.0*t5) + 94.0*L3*m5*sin(2.0*t2 + 2.0*t3 + t4 - 1.0*t5) - 25.625*L3*m5*sin(2.0*t2 + 2.0*t3 + 2.0*t4 + t5) + 204.0*L4*m5*sin(t3 + t4) - 204.0*L4*m5*sin(2.0*t2 + t3 + t4) - 51.0*L3*m5*sin(t3 + t4 - 1.0*t5) + 51.0*L3*m5*sin(2.0*t2 + t3 + t4 - 1.0*t5) - 94.0*L3*m5*sin(2.0*t2 + 2.0*t3 + t4 + t5) - 0.25*L3*L4*m5*sin(2.0*t2 + 2.0*t3 + 2.0*t4 - 1.0*t5) + 0.25*L3*L4*m5*sin(2.0*t2 + 2.0*t3 + 2.0*t4 + t5)))
     td6*(td1*(0.00084023437500000005238864897449957*cos(t1)*cos(t5)*sin(t1) + 0.00042011718750000002619432448724979*cos(t1)^2*cos(t2)*cos(t3)*cos(t4)*sin(t5) - 0.00042011718750000002619432448724979*cos(t2)*cos(t3)*cos(t4)*sin(t1)^2*sin(t5) - 0.00042011718750000002619432448724979*cos(t1)^2*cos(t2)*sin(t3)*sin(t4)*sin(t5) - 0.00042011718750000002619432448724979*cos(t1)^2*cos(t3)*sin(t2)*sin(t4)*sin(t5) - 0.00042011718750000002619432448724979*cos(t1)^2*cos(t4)*sin(t2)*sin(t3)*sin(t5) + 0.00042011718750000002619432448724979*cos(t2)*sin(t1)^2*sin(t3)*sin(t4)*sin(t5) + 0.00042011718750000002619432448724979*cos(t3)*sin(t1)^2*sin(t2)*sin(t4)*sin(t5) + 0.00042011718750000002619432448724979*cos(t4)*sin(t1)^2*sin(t2)*sin(t3)*sin(t5)) + td6*(0.5*(0.00084023437500000005238864897449957*cos(t1)*cos(t2)*cos(t3)*sin(t4)*sin(t5) + 0.00084023437500000005238864897449957*cos(t1)*cos(t2)*cos(t4)*sin(t3)*sin(t5) + 0.00084023437500000005238864897449957*cos(t1)*cos(t3)*cos(t4)*sin(t2)*sin(t5) - 0.00084023437500000005238864897449957*cos(t1)*sin(t2)*sin(t3)*sin(t4)*sin(t5))*(cos(t1)*cos(t2)*sin(t3)*sin(t4)*sin(t5) - 1.0*cos(t1)*cos(t2)*cos(t3)*cos(t4)*sin(t5) - 1.0*cos(t5)*sin(t1) + cos(t1)*cos(t3)*sin(t2)*sin(t4)*sin(t5) + cos(t1)*cos(t4)*sin(t2)*sin(t3)*sin(t5)) + 0.5*(cos(t1)*cos(t2)*cos(t3)*sin(t4)*sin(t5) + cos(t1)*cos(t2)*cos(t4)*sin(t3)*sin(t5) + cos(t1)*cos(t3)*cos(t4)*sin(t2)*sin(t5) - 1.0*cos(t1)*sin(t2)*sin(t3)*sin(t4)*sin(t5))*(0.00084023437500000005238864897449957*cos(t1)*cos(t2)*sin(t3)*sin(t4)*sin(t5) - 0.00084023437500000005238864897449957*cos(t1)*cos(t2)*cos(t3)*cos(t4)*sin(t5) - 0.00084023437500000005238864897449957*cos(t5)*sin(t1) + 0.00084023437500000005238864897449957*cos(t1)*cos(t3)*sin(t2)*sin(t4)*sin(t5) + 0.00084023437500000005238864897449957*cos(t1)*cos(t4)*sin(t2)*sin(t3)*sin(t5)) + 0.5*(0.0016804687500000001047772979489991*cos(t2)*cos(t3)*sin(t1)*sin(t4)*sin(t5) + 0.0016804687500000001047772979489991*cos(t2)*cos(t4)*sin(t1)*sin(t3)*sin(t5) + 0.0016804687500000001047772979489991*cos(t3)*cos(t4)*sin(t1)*sin(t2)*sin(t5) - 0.0016804687500000001047772979489991*sin(t1)*sin(t2)*sin(t3)*sin(t4)*sin(t5))*(cos(t1)*cos(t5) - 1.0*cos(t2)*cos(t3)*cos(t4)*sin(t1)*sin(t5) + cos(t2)*sin(t1)*sin(t3)*sin(t4)*sin(t5) + cos(t3)*sin(t1)*sin(t2)*sin(t4)*sin(t5) + cos(t4)*sin(t1)*sin(t2)*sin(t3)*sin(t5)) + 0.5*(cos(t2)*cos(t3)*sin(t1)*sin(t4)*sin(t5) + cos(t2)*cos(t4)*sin(t1)*sin(t3)*sin(t5) + cos(t3)*cos(t4)*sin(t1)*sin(t2)*sin(t5) - 1.0*sin(t1)*sin(t2)*sin(t3)*sin(t4)*sin(t5))*(0.0016804687500000001047772979489991*cos(t1)*cos(t5) - 0.0016804687500000001047772979489991*cos(t2)*cos(t3)*cos(t4)*sin(t1)*sin(t5) + 0.0016804687500000001047772979489991*cos(t2)*sin(t1)*sin(t3)*sin(t4)*sin(t5) + 0.0016804687500000001047772979489991*cos(t3)*sin(t1)*sin(t2)*sin(t4)*sin(t5) + 0.0016804687500000001047772979489991*cos(t4)*sin(t1)*sin(t2)*sin(t3)*sin(t5))) - 1.0*td5*(0.00063017578125000003929148673087468*cos(2.0*t2)*cos(2.0*t3)*cos(2.0*t4)*sin(t5) - 0.00042011718750000002619432448724979*cos(t1)^2*sin(t5) - 0.00042011718750000002619432448724979*sin(t5) - 0.00063017578125000003929148673087468*cos(2.0*t2)*sin(2.0*t3)*sin(2.0*t4)*sin(t5) - 0.00063017578125000003929148673087468*cos(2.0*t3)*sin(2.0*t2)*sin(2.0*t4)*sin(t5) - 0.00063017578125000003929148673087468*cos(2.0*t4)*sin(2.0*t2)*sin(2.0*t3)*sin(t5) - 0.00021005859375000001309716224362489*cos(2.0*t1)*cos(2.0*t2)*cos(2.0*t3)*cos(2.0*t4)*sin(t5) + 0.00021005859375000001309716224362489*cos(2.0*t1)*cos(2.0*t2)*sin(2.0*t3)*sin(2.0*t4)*sin(t5) + 0.00021005859375000001309716224362489*cos(2.0*t1)*cos(2.0*t3)*sin(2.0*t2)*sin(2.0*t4)*sin(t5) + 0.00021005859375000001309716224362489*cos(2.0*t1)*cos(2.0*t4)*sin(2.0*t2)*sin(2.0*t3)*sin(t5) - 0.00021005859375000001309716224362489*sin(2.0*t1)*cos(t2)*cos(t3)*cos(t4)*cos(t5) + 0.00021005859375000001309716224362489*sin(2.0*t1)*cos(t2)*cos(t5)*sin(t3)*sin(t4) + 0.00021005859375000001309716224362489*sin(2.0*t1)*cos(t3)*cos(t5)*sin(t2)*sin(t4) + 0.00021005859375000001309716224362489*sin(2.0*t1)*cos(t4)*cos(t5)*sin(t2)*sin(t3) - 0.00042011718750000002619432448724979*cos(t1)*cos(t2)*cos(t3)*cos(t4)*cos(t5)*sin(t1) + 0.00042011718750000002619432448724979*cos(t1)*cos(t2)*cos(t5)*sin(t1)*sin(t3)*sin(t4) + 0.00042011718750000002619432448724979*cos(t1)*cos(t3)*cos(t5)*sin(t1)*sin(t2)*sin(t4) + 0.00042011718750000002619432448724979*cos(t1)*cos(t4)*cos(t5)*sin(t1)*sin(t2)*sin(t3))) - td3*(1.0*td2*(0.0029327291666666668173979459766088*cos(t3)*sin(t3) + 153408.0*m4*sin(t3) + 153408.0*m5*sin(t3) + 153408.0*m6*sin(t3) + 0.0029327291666666668173979459766088*cos(t1)*cos(t3)^2*sin(t1) - 0.0058654583333333336347958919532175*cos(t1)^2*cos(t3)*sin(t3) - 0.0029327291666666668173979459766088*cos(t1)*sin(t1)*sin(t3)^2 + 41820.0*m5*cos(t3)*sin(t4) + 41820.0*m5*cos(t4)*sin(t3) + 41820.0*m6*cos(t3)*sin(t4) + 41820.0*m6*cos(t4)*sin(t3) - 408.0*L4*m5*cos(t3)*sin(t4) - 408.0*L4*m5*cos(t4)*sin(t3) - 204.0*L3*m5*cos(t3)*cos(t4)*sin(t5) + 204.0*L3*m5*sin(t3)*sin(t4)*sin(t5)) - td1*(0.00073318229166666670434948649415219*sin(t1 - 2.0*t2) + 0.00073318229166666670434948649415219*sin(t1 + 2.0*t2) + 0.00024028885416666671912683250766918*sin(2.0*t1) - 0.00036659114583333335217474324707609*sin(2.0*t1 - 2.0*t2) - 0.00036659114583333335217474324707609*sin(2.0*t1 + 2.0*t2) - 0.0014663645833333334086989729883044*sin(2.0*t1 - 2.0*t3) + 52828.0*m4*sin(t2 + t3) + 52828.0*m5*sin(t2 + t3) + 52828.0*m6*sin(t2 + t3) + 14401.25*m5*sin(t2 + t3 + t4) + 14401.25*m6*sin(t2 + t3 + t4) + 94.0*L3*m5*sin(t2 + t3 + t5) - 140.5*L4*m5*sin(t2 + t3 + t4) + 60.75*L3*m5*sin(t2 + t3 + t4 - 1.0*t5) + 0.0625*L3^2*m5*sin(t2 + t3 + t4 - 2.0*t5) - 0.0625*L3^2*m5*sin(t2 + t3 + t4 + 2.0*t5) - 9.5*L3*m5*sin(t2 + t3 + t4 + t5) - 376.0*L1*m4*sin(t2 + t3) + 94.0*L3*m5*sin(t2 + t3 - 1.0*t5) - 0.25*L3*L4*m5*sin(t2 + t3 + t4 + t5) - 0.25*L3*L4*m5*sin(t2 + t3 + t4 - 1.0*t5)) + 1.0*td3*(0.0029327291666666668173979459766088*cos(t2)*sin(t2) - 0.0029327291666666668173979459766088*cos(t1)^2*cos(t2)*sin(t2)) + 1.0*td5*(0.00073318229166666670434948649415219*sin(3.0*t2 - 1.0*t1 + t3 + t4) - 0.0014663645833333334086989729883044*sin(t2 - 2.0*t1 + 3.0*t3 + t4) - 0.00036659114583333335217474324707609*sin(3.0*t2 - 2.0*t1 + t3 + t4) + 0.00036659114583333335217474324707609*sin(2.0*t1 + 3.0*t2 + t3 + t4) + 0.00057664973958333336527190549070099*sin(t2 - 2.0*t1 + t3 + t4) - 0.00057664973958333336527190549070099*sin(2.0*t1 + t2 + t3 + t4) - 0.00073318229166666670434948649415219*sin(t1 + 3.0*t2 + t3 + t4) + 94.0*L3*m5*sin(t4 - 1.0*t5) + 94.0*L3*m5*sin(t4 + t5) + 0.125*L3^2*m5*sin(2.0*t5)) - td6*(0.00084023437500000005238864897449957*cos(t1)*cos(t2)*cos(t3)*sin(t1)*sin(t4)*sin(t5) + 0.00084023437500000005238864897449957*cos(t1)*cos(t2)*cos(t4)*sin(t1)*sin(t3)*sin(t5) + 0.00084023437500000005238864897449957*cos(t1)*cos(t3)*cos(t4)*sin(t1)*sin(t2)*sin(t5) - 0.00084023437500000005238864897449957*cos(t1)*sin(t1)*sin(t2)*sin(t3)*sin(t4)*sin(t5)) + 1.0*td4*(- 0.0029327291666666668173979459766088*cos(t2)*sin(t2)*cos(t1)^2 + 0.0014663645833333334086989729883044*sin(2.0*t1 - 2.0*t3) + 0.0029327291666666668173979459766088*cos(t2)*sin(t2) - 38540.0*m5*sin(t4) - 38540.0*m6*sin(t4) - 94.0*L3*m5*sin(t4 - 1.0*t5) + 94.0*L3*m5*sin(t4 + t5) + 376.0*L4*m5*sin(t4))) + td2*(td6*(0.00084023437500000005238864897449957*cos(t1)*cos(t2)*cos(t3)*sin(t1)*sin(t4)*sin(t5) + 0.00084023437500000005238864897449957*cos(t1)*cos(t2)*cos(t4)*sin(t1)*sin(t3)*sin(t5) + 0.00084023437500000005238864897449957*cos(t1)*cos(t3)*cos(t4)*sin(t1)*sin(t2)*sin(t5) - 0.00084023437500000005238864897449957*cos(t1)*sin(t1)*sin(t2)*sin(t3)*sin(t4)*sin(t5)) - 1.0*td2*(- 0.25*m2*cos(t2)*sin(t2)*L2^2*cos(t1)^2 + 0.25*m2*cos(t2)*sin(t2)*L2^2 + 70.25*m2*cos(t2)*sin(t1)*L2*cos(t1) + 0.10662220333333332668301896006824*cos(t2)*sin(t2)*cos(t1)^2 - 0.10662220333333332668301896006824*cos(t2)*sin(t2)) + td1*(52828.0*m4*sin(t2 + t3) - 0.053311101666666663341509480034119*sin(t1 + 2.0*t2) - 0.1046752610416666598360663220646*cos(t1)*sin(t1) - 0.053311101666666663341509480034119*sin(t1 - 2.0*t2) + 52828.0*m5*sin(t2 + t3) + 52828.0*m6*sin(t2 + t3) + 57324.0*m3*sin(t2) + 57324.0*m4*sin(t2) + 57324.0*m5*sin(t2) + 57324.0*m6*sin(t2) + 14401.25*m5*sin(t2 + t3 + t4) + 14401.25*m6*sin(t2 + t3 + t4) + 94.0*L3*m5*sin(t2 + t3 + t5) - 140.5*L4*m5*sin(t2 + t3 + t4) + 0.10662220333333332668301896006824*cos(t1)*cos(t2)^2*sin(t1) - 0.0058654583333333336347958919532175*cos(t1)*cos(t3)^2*sin(t1) + 0.0029327291666666668173979459766088*cos(t1)^2*cos(t3)*sin(t3) + 60.75*L3*m5*sin(t2 + t3 + t4 - 1.0*t5) - 0.0029327291666666668173979459766088*cos(t3)*sin(t1)^2*sin(t3) - 35.125*L2*m2*sin(t1 - 1.0*t2) + 102.0*L3*m5*sin(t2 - 1.0*t5) - 19740.25*m2*cos(t1)*sin(t1) + 0.0625*L3^2*m5*sin(t2 + t3 + t4 - 2.0*t5) - 0.0625*L3^2*m5*sin(t2 + t3 + t4 + 2.0*t5) - 9.5*L3*m5*sin(t2 + t3 + t4 + t5) - 0.125*L2^2*m2*sin(t1 - 2.0*t2) - 0.125*L2^2*m2*sin(t1 + 2.0*t2) + 35.125*L2*m2*sin(t1 + t2) - 376.0*L1*m4*sin(t2 + t3) + 102.0*L3*m5*sin(t2 + t5) + 94.0*L3*m5*sin(t2 + t3 - 1.0*t5) - 408.0*L1*m3*sin(t2) - 408.0*L1*m4*sin(t2) - 0.25*L3*L4*m5*sin(t2 + t3 + t4 + t5) + 0.25*L2^2*m2*cos(t1)*sin(t1) + 70.25*L2*m2*cos(t1)^2*sin(t2) - 70.25*L2*m2*sin(t1)^2*sin(t2) - 0.25*L3*L4*m5*sin(t2 + t3 + t4 - 1.0*t5) - 0.25*L2^2*m2*cos(t1)*cos(t2)^2*sin(t1)) + td4*(0.00073318229166666670434948649415219*sin(2.0*t1 + 2.0*t2) - 0.00073318229166666670434948649415219*sin(2.0*t1 - 2.0*t2) - 0.0014663645833333334086989729883044*sin(2.0*t2) + 38540.0*m5*sin(t4) + 38540.0*m6*sin(t4) + 41820.0*m5*cos(t3)*sin(t4) + 41820.0*m5*cos(t4)*sin(t3) + 41820.0*m6*cos(t3)*sin(t4) + 41820.0*m6*cos(t4)*sin(t3) - 376.0*L4*m5*sin(t4) - 408.0*L4*m5*cos(t3)*sin(t4) - 408.0*L4*m5*cos(t4)*sin(t3) - 188.0*L3*m5*cos(t4)*sin(t5) - 204.0*L3*m5*cos(t3)*cos(t4)*sin(t5) + 204.0*L3*m5*sin(t3)*sin(t4)*sin(t5)) + td3*(0.00073318229166666670434948649415219*sin(2.0*t1 + 2.0*t2) - 0.00073318229166666670434948649415219*sin(2.0*t1 - 2.0*t2) - 0.0014663645833333334086989729883044*sin(2.0*t2) + 0.0029327291666666668173979459766088*cos(t3)*sin(t3) + 153408.0*m4*sin(t3) + 153408.0*m5*sin(t3) + 153408.0*m6*sin(t3) + 0.0029327291666666668173979459766088*cos(t1)*cos(t3)^2*sin(t1) - 0.0058654583333333336347958919532175*cos(t1)^2*cos(t3)*sin(t3) - 0.0029327291666666668173979459766088*cos(t1)*sin(t1)*sin(t3)^2 + 41820.0*m5*cos(t3)*sin(t4) + 41820.0*m5*cos(t4)*sin(t3) + 41820.0*m6*cos(t3)*sin(t4) + 41820.0*m6*cos(t4)*sin(t3) - 408.0*L4*m5*cos(t3)*sin(t4) - 408.0*L4*m5*cos(t4)*sin(t3) - 204.0*L3*m5*cos(t3)*cos(t4)*sin(t5) + 204.0*L3*m5*sin(t3)*sin(t4)*sin(t5)) - td5*(0.0010997734375000000565242297412283*sin(3.0*t2 - 1.0*t1 + t3 + t4) - 0.00073318229166666670434948649415219*sin(t2 - 2.0*t1 + 3.0*t3 + t4) - 0.00054988671875000002826211487061414*sin(3.0*t2 - 2.0*t1 + t3 + t4) + 0.00054988671875000002826211487061414*sin(2.0*t1 + 3.0*t2 + t3 + t4) - 0.00036659114583333335217474324707609*sin(t1 - 1.0*t2 + t3 + t4) + 0.00057664973958333336527190549070099*sin(t2 - 2.0*t1 + t3 + t4) - 0.00057664973958333336527190549070099*sin(2.0*t1 + t2 + t3 + t4) - 0.0010997734375000000565242297412283*sin(t1 + 3.0*t2 + t3 + t4) - 0.00018329557291666667608737162353805*sin(2.0*t1 + t2 - 1.0*t3 - 1.0*t4) - 0.00036659114583333335217474324707609*sin(t1 + t2 - 1.0*t3 - 1.0*t4) + 0.00073318229166666670434948649415219*sin(2.0*t1 + t2 - 1.0*t3 + t4) - 0.00018329557291666667608737162353805*sin(2.0*t1 - 1.0*t2 + t3 + t4) + 0.25*L3^2*m5*cos(t5)*sin(t5) + 188.0*L3*m5*cos(t5)*sin(t4) + 204.0*L3*m5*cos(t3)*cos(t5)*sin(t4) + 204.0*L3*m5*cos(t4)*cos(t5)*sin(t3))) + td1*(td2*(0.1046752610416666598360663220646*cos(t1)*sin(t1) - 0.10662220333333332668301896006824*cos(t1)*cos(t2)^2*sin(t1) + 0.0058654583333333336347958919532175*cos(t1)*cos(t3)^2*sin(t1) - 0.0029327291666666668173979459766088*cos(t1)^2*cos(t3)*sin(t3) + 0.0029327291666666668173979459766088*cos(t3)*sin(t1)^2*sin(t3) + 19740.25*m2*cos(t1)*sin(t1) - 0.25*L2^2*m2*cos(t1)*sin(t1) - 70.25*L2*m2*cos(t1)^2*sin(t2) + 70.25*L2*m2*sin(t1)^2*sin(t2) + 0.25*L2^2*m2*cos(t1)*cos(t2)^2*sin(t1)) - 1.0*td5*(0.00036659114583333335217474324707609*sin(3.0*t2 - 1.0*t1 + t3 + t4) + 0.00073318229166666670434948649415219*sin(t2 - 2.0*t1 + 3.0*t3 + t4) + 0.00018329557291666667608737162353805*sin(3.0*t2 - 2.0*t1 + t3 + t4) + 0.00018329557291666667608737162353805*sin(2.0*t1 + 3.0*t2 + t3 + t4) + 0.00073318229166666670434948649415219*sin(t2 + t3 + t4) + 0.00036659114583333335217474324707609*sin(t1 - 1.0*t2 + t3 + t4) - 0.00057664973958333336527190549070099*sin(t2 - 2.0*t1 + t3 + t4) - 0.00057664973958333336527190549070099*sin(2.0*t1 + t2 + t3 + t4) + 0.00036659114583333335217474324707609*sin(t1 + 3.0*t2 + t3 + t4) - 0.00018329557291666667608737162353805*sin(2.0*t1 + t2 - 1.0*t3 - 1.0*t4) + 0.00036659114583333335217474324707609*sin(t3 - 1.0*t2 + t4) - 0.00036659114583333335217474324707609*sin(t1 + t2 - 1.0*t3 - 1.0*t4) + 0.00073318229166666670434948649415219*sin(2.0*t1 + t2 - 1.0*t3 + t4) + 0.00018329557291666667608737162353805*sin(2.0*t1 - 1.0*t2 + t3 + t4) - 0.0010997734375000000565242297412283*sin(3.0*t2 + t3 + t4) + 94.0*L3*m5*sin(t2 + t3 + t5) - 25.625*L3*m5*sin(t2 + t3 + t4 - 1.0*t5) - 102.0*L3*m5*sin(t2 - 1.0*t5) + 0.125*L3^2*m5*sin(t2 + t3 + t4) - 0.0625*L3^2*m5*sin(t2 + t3 + t4 - 2.0*t5) - 0.0625*L3^2*m5*sin(t2 + t3 + t4 + 2.0*t5) + 25.625*L3*m5*sin(t2 + t3 + t4 + t5) + 102.0*L3*m5*sin(t2 + t5) - 94.0*L3*m5*sin(t2 + t3 - 1.0*t5) - 0.25*L3*L4*m5*sin(t2 + t3 + t4 + t5) + 0.25*L3*L4*m5*sin(t2 + t3 + t4 - 1.0*t5)) - 1.0*td6*(0.00084023437500000005238864897449957*cos(t1)*cos(t5)*sin(t1) + 0.00042011718750000002619432448724979*cos(t1)^2*cos(t2)*cos(t3)*cos(t4)*sin(t5) - 0.00042011718750000002619432448724979*cos(t2)*cos(t3)*cos(t4)*sin(t1)^2*sin(t5) - 0.00042011718750000002619432448724979*cos(t1)^2*cos(t2)*sin(t3)*sin(t4)*sin(t5) - 0.00042011718750000002619432448724979*cos(t1)^2*cos(t3)*sin(t2)*sin(t4)*sin(t5) - 0.00042011718750000002619432448724979*cos(t1)^2*cos(t4)*sin(t2)*sin(t3)*sin(t5) + 0.00042011718750000002619432448724979*cos(t2)*sin(t1)^2*sin(t3)*sin(t4)*sin(t5) + 0.00042011718750000002619432448724979*cos(t3)*sin(t1)^2*sin(t2)*sin(t4)*sin(t5) + 0.00042011718750000002619432448724979*cos(t4)*sin(t1)^2*sin(t2)*sin(t3)*sin(t5)) + td4*(0.00073318229166666670434948649415219*sin(t1 - 2.0*t2) + 0.00073318229166666670434948649415219*sin(t1 + 2.0*t2) - 0.001153299479166666730543810981402*sin(2.0*t1) + 0.00036659114583333335217474324707609*sin(2.0*t1 - 2.0*t2) + 0.00036659114583333335217474324707609*sin(2.0*t1 + 2.0*t2) + 0.0014663645833333334086989729883044*sin(2.0*t1 - 2.0*t3)) + td3*(0.00073318229166666670434948649415219*sin(t1 - 2.0*t2) + 0.00073318229166666670434948649415219*sin(t1 + 2.0*t2) - 0.00024028885416666671912683250766918*sin(2.0*t1) + 0.00036659114583333335217474324707609*sin(2.0*t1 - 2.0*t2) + 0.00036659114583333335217474324707609*sin(2.0*t1 + 2.0*t2) + 0.0014663645833333334086989729883044*sin(2.0*t1 - 2.0*t3)) + td1*(153408.0*m4*sin(2.0*t2 + t3) - 0.053311101666666663341509480034119*sin(2.0*t2) + 153408.0*m5*sin(2.0*t2 + t3) + 153408.0*m6*sin(2.0*t2 + t3) + 38540.0*m5*sin(2.0*t2 + 2.0*t3 + t4) + 38540.0*m6*sin(2.0*t2 + 2.0*t3 + t4) + 83232.0*m3*sin(2.0*t2) + 83232.0*m4*sin(2.0*t2) + 83232.0*m5*sin(2.0*t2) + 83232.0*m6*sin(2.0*t2) + 41820.0*m5*sin(2.0*t2 + t3 + t4) + 41820.0*m6*sin(2.0*t2 + t3 + t4) + 70688.0*m4*sin(2.0*t2 + 2.0*t3) + 70688.0*m5*sin(2.0*t2 + 2.0*t3) + 70688.0*m6*sin(2.0*t2 + 2.0*t3) + 5253.125*m5*sin(2.0*t2 + 2.0*t3 + 2.0*t4) + 5253.125*m6*sin(2.0*t2 + 2.0*t3 + 2.0*t4) - 102.5*L4*m5*sin(2.0*t2 + 2.0*t3 + 2.0*t4) + 25.625*L3*m5*sin(2.0*t2 + 2.0*t3 + 2.0*t4 - 1.0*t5) - 102.0*L3*m5*sin(2.0*t2 + t3 + t4 + t5) - 0.0625*L3^2*m5*sin(2.0*t2 + 2.0*t3 + 2.0*t4) + 0.5*L4^2*m5*sin(2.0*t2 + 2.0*t3 + 2.0*t4) - 376.0*L4*m5*sin(2.0*t2 + 2.0*t3 + t4) + 0.03125*L3^2*m5*sin(2.0*t2 + 2.0*t3 + 2.0*t4 - 2.0*t5) + 0.03125*L3^2*m5*sin(2.0*t2 + 2.0*t3 + 2.0*t4 + 2.0*t5) + 94.0*L3*m5*sin(2.0*t2 + 2.0*t3 + t4 - 1.0*t5) - 25.625*L3*m5*sin(2.0*t2 + 2.0*t3 + 2.0*t4 + t5) - 408.0*L4*m5*sin(2.0*t2 + t3 + t4) + 102.0*L3*m5*sin(2.0*t2 + t3 + t4 - 1.0*t5) - 94.0*L3*m5*sin(2.0*t2 + 2.0*t3 + t4 + t5) + 0.125*L2^2*m2*sin(2.0*t2) - 0.25*L3*L4*m5*sin(2.0*t2 + 2.0*t3 + 2.0*t4 - 1.0*t5) + 0.25*L3*L4*m5*sin(2.0*t2 + 2.0*t3 + 2.0*t4 + t5))) - td4*(1.0*td5*(0.125*m5*sin(2.0*t5)*L3^2 + 0.00073318229166666670434948649415219*sin(3.0*t2 - 1.0*t1 + t3 + t4) - 0.00073318229166666670434948649415219*sin(t2 - 2.0*t1 + 3.0*t3 + t4) - 0.00036659114583333335217474324707609*sin(3.0*t2 - 2.0*t1 + t3 + t4) + 0.00036659114583333335217474324707609*sin(2.0*t1 + 3.0*t2 + t3 + t4) + 0.00057664973958333336527190549070099*sin(t2 - 2.0*t1 + t3 + t4) - 0.00057664973958333336527190549070099*sin(2.0*t1 + t2 + t3 + t4) - 0.00073318229166666670434948649415219*sin(t1 + 3.0*t2 + t3 + t4) + 0.00073318229166666670434948649415219*sin(2.0*t1 + t2 - 1.0*t3 + t4)) + 1.0*td1*(0.00036659114583333335217474324707609*sin(2.0*t1 - 2.0*t2) - 0.00073318229166666670434948649415219*sin(t1 + 2.0*t2) - 0.001153299479166666730543810981402*sin(2.0*t1) - 0.00073318229166666670434948649415219*sin(t1 - 2.0*t2) + 0.00036659114583333335217474324707609*sin(2.0*t1 + 2.0*t2) + 0.0014663645833333334086989729883044*sin(2.0*t1 - 2.0*t3) - 14401.25*m5*sin(t2 + t3 + t4) - 14401.25*m6*sin(t2 + t3 + t4) + 140.5*L4*m5*sin(t2 + t3 + t4) - 60.75*L3*m5*sin(t2 + t3 + t4 - 1.0*t5) - 0.0625*L3^2*m5*sin(t2 + t3 + t4 - 2.0*t5) + 0.0625*L3^2*m5*sin(t2 + t3 + t4 + 2.0*t5) + 9.5*L3*m5*sin(t2 + t3 + t4 + t5) + 0.25*L3*L4*m5*sin(t2 + t3 + t4 + t5) + 0.25*L3*L4*m5*sin(t2 + t3 + t4 - 1.0*t5)) + 1.0*td4*(0.00073318229166666670434948649415219*sin(2.0*t2) - 0.00073318229166666670434948649415219*cos(2.0*t1)*sin(2.0*t2)) - td6*(0.00084023437500000005238864897449957*cos(t1)*cos(t2)*cos(t3)*sin(t1)*sin(t4)*sin(t5) + 0.00084023437500000005238864897449957*cos(t1)*cos(t2)*cos(t4)*sin(t1)*sin(t3)*sin(t5) + 0.00084023437500000005238864897449957*cos(t1)*cos(t3)*cos(t4)*sin(t1)*sin(t2)*sin(t5) - 0.00084023437500000005238864897449957*cos(t1)*sin(t1)*sin(t2)*sin(t3)*sin(t4)*sin(t5)) - td3*(0.0029327291666666668173979459766088*cos(t2)*sin(t2)*cos(t1)^2 + 0.0014663645833333334086989729883044*sin(2.0*t1 - 2.0*t3) - 0.0029327291666666668173979459766088*cos(t2)*sin(t2) - 38540.0*m5*sin(t4) - 38540.0*m6*sin(t4) - 94.0*L3*m5*sin(t4 - 1.0*t5) + 94.0*L3*m5*sin(t4 + t5) + 376.0*L4*m5*sin(t4)) + 1.0*td2*(38540.0*m5*sin(t4) + 38540.0*m6*sin(t4) + 41820.0*m5*cos(t3)*sin(t4) + 41820.0*m5*cos(t4)*sin(t3) + 41820.0*m6*cos(t3)*sin(t4) + 41820.0*m6*cos(t4)*sin(t3) - 376.0*L4*m5*sin(t4) - 408.0*L4*m5*cos(t3)*sin(t4) - 408.0*L4*m5*cos(t4)*sin(t3) - 188.0*L3*m5*cos(t4)*sin(t5) - 204.0*L3*m5*cos(t3)*cos(t4)*sin(t5) + 204.0*L3*m5*sin(t3)*sin(t4)*sin(t5))) + td5*(td2*(0.25*L3^2*m5*cos(t5)*sin(t5) + 188.0*L3*m5*cos(t5)*sin(t4) + 204.0*L3*m5*cos(t3)*cos(t5)*sin(t4) + 204.0*L3*m5*cos(t4)*cos(t5)*sin(t3)) - 1.0*td1*(0.00073318229166666670434948649415219*sin(3.0*t2 - 1.0*t1 + t3 + t4) - 0.00073318229166666670434948649415219*sin(t2 - 2.0*t1 + 3.0*t3 + t4) - 0.00018329557291666667608737162353805*sin(3.0*t2 - 2.0*t1 + t3 + t4) - 0.00018329557291666667608737162353805*sin(2.0*t1 + 3.0*t2 + t3 + t4) + 0.00073318229166666670434948649415219*sin(t2 + t3 + t4) + 0.00057664973958333336527190549070099*sin(t2 - 2.0*t1 + t3 + t4) + 0.00057664973958333336527190549070099*sin(2.0*t1 + t2 + t3 + t4) + 0.00073318229166666670434948649415219*sin(t1 + 3.0*t2 + t3 + t4) + 0.00018329557291666667608737162353805*sin(2.0*t1 + t2 - 1.0*t3 - 1.0*t4) + 0.00036659114583333335217474324707609*sin(t3 - 1.0*t2 + t4) - 0.00073318229166666670434948649415219*sin(2.0*t1 + t2 - 1.0*t3 + t4) - 0.00018329557291666667608737162353805*sin(2.0*t1 - 1.0*t2 + t3 + t4) - 0.0010997734375000000565242297412283*sin(3.0*t2 + t3 + t4) + 35.125*L3*m5*sin(t2 + t3 + t4 - 1.0*t5) + 0.125*L3^2*m5*sin(t2 + t3 + t4) + 0.0625*L3^2*m5*sin(t2 + t3 + t4 - 2.0*t5) + 0.0625*L3^2*m5*sin(t2 + t3 + t4 + 2.0*t5) + 35.125*L3*m5*sin(t2 + t3 + t4 + t5)) + td4*(0.125*m5*sin(2.0*t5)*L3^2 - 0.00036659114583333335217474324707609*sin(3.0*t2 - 1.0*t1 + t3 + t4) + 0.00018329557291666667608737162353805*sin(3.0*t2 - 2.0*t1 + t3 + t4) - 0.00018329557291666667608737162353805*sin(2.0*t1 + 3.0*t2 + t3 + t4) + 0.00036659114583333335217474324707609*sin(t1 - 1.0*t2 + t3 + t4) + 0.00036659114583333335217474324707609*sin(t1 + 3.0*t2 + t3 + t4) + 0.00018329557291666667608737162353805*sin(2.0*t1 + t2 - 1.0*t3 - 1.0*t4) + 0.00036659114583333335217474324707609*sin(t1 + t2 - 1.0*t3 - 1.0*t4) + 0.00018329557291666667608737162353805*sin(2.0*t1 - 1.0*t2 + t3 + t4)) + td5*(0.00036659114583333335217474324707609*sin(2.0*t1 + 2.0*t2 + 2.0*t4) + 0.001729949218750000095815716472103*sin(2.0*t2 + 2.0*t3 + 2.0*t4) + 0.0010997734375000000565242297412283*sin(4.0*t2 + 2.0*t3 + 2.0*t4) - 0.00073318229166666670434948649415219*sin(4.0*t2 - 1.0*t1 + 2.0*t3 + 2.0*t4) - 0.00028832486979166668263595274535049*sin(2.0*t2 - 2.0*t1 + 2.0*t3 + 2.0*t4) - 0.00028832486979166668263595274535049*sin(2.0*t1 + 2.0*t2 + 2.0*t3 + 2.0*t4) + 0.00036659114583333335217474324707609*sin(2.0*t2 - 2.0*t1 + 4.0*t3 + 2.0*t4) + 0.00018329557291666667608737162353805*sin(4.0*t2 - 2.0*t1 + 2.0*t3 + 2.0*t4) + 0.00018329557291666667608737162353805*sin(2.0*t1 + 4.0*t2 + 2.0*t3 + 2.0*t4) - 0.00073318229166666670434948649415219*sin(t1 + 4.0*t2 + 2.0*t3 + 2.0*t4) + 0.00036659114583333335217474324707609*sin(2.0*t2) + 0.00018329557291666667608737162353805*sin(2.0*t1 - 2.0*t2) - 0.00018329557291666667608737162353805*sin(2.0*t1 + 2.0*t2)) + td3*(0.00018329557291666667608737162353805*sin(3.0*t2 - 2.0*t1 + t3 + t4) - 0.00073318229166666670434948649415219*sin(t2 - 2.0*t1 + 3.0*t3 + t4) - 0.00036659114583333335217474324707609*sin(3.0*t2 - 1.0*t1 + t3 + t4) - 0.00018329557291666667608737162353805*sin(2.0*t1 + 3.0*t2 + t3 + t4) + 0.00036659114583333335217474324707609*sin(t1 - 1.0*t2 + t3 + t4) + 0.00036659114583333335217474324707609*sin(t1 + 3.0*t2 + t3 + t4) + 0.00018329557291666667608737162353805*sin(2.0*t1 + t2 - 1.0*t3 - 1.0*t4) + 0.00036659114583333335217474324707609*sin(t1 + t2 - 1.0*t3 - 1.0*t4) - 0.00073318229166666670434948649415219*sin(2.0*t1 + t2 - 1.0*t3 + t4) + 0.00018329557291666667608737162353805*sin(2.0*t1 - 1.0*t2 + t3 + t4) + 94.0*L3*m5*sin(t4 - 1.0*t5) + 94.0*L3*m5*sin(t4 + t5) + 0.125*L3^2*m5*sin(2.0*t5)) - 1.0*td6*(0.00042011718750000002619432448724979*sin(t5) + 0.00042011718750000002619432448724979*cos(t1)^2*sin(t5) + 0.00063017578125000003929148673087468*cos(2.0*t2)*cos(2.0*t3)*cos(2.0*t4)*sin(t5) - 0.00063017578125000003929148673087468*cos(2.0*t2)*sin(2.0*t3)*sin(2.0*t4)*sin(t5) - 0.00063017578125000003929148673087468*cos(2.0*t3)*sin(2.0*t2)*sin(2.0*t4)*sin(t5) - 0.00063017578125000003929148673087468*cos(2.0*t4)*sin(2.0*t2)*sin(2.0*t3)*sin(t5) - 0.00021005859375000001309716224362489*cos(2.0*t1)*cos(2.0*t2)*cos(2.0*t3)*cos(2.0*t4)*sin(t5) + 0.00021005859375000001309716224362489*cos(2.0*t1)*cos(2.0*t2)*sin(2.0*t3)*sin(2.0*t4)*sin(t5) + 0.00021005859375000001309716224362489*cos(2.0*t1)*cos(2.0*t3)*sin(2.0*t2)*sin(2.0*t4)*sin(t5) + 0.00021005859375000001309716224362489*cos(2.0*t1)*cos(2.0*t4)*sin(2.0*t2)*sin(2.0*t3)*sin(t5) - 0.00021005859375000001309716224362489*sin(2.0*t1)*cos(t2)*cos(t3)*cos(t4)*cos(t5) + 0.00021005859375000001309716224362489*sin(2.0*t1)*cos(t2)*cos(t5)*sin(t3)*sin(t4) + 0.00021005859375000001309716224362489*sin(2.0*t1)*cos(t3)*cos(t5)*sin(t2)*sin(t4) + 0.00021005859375000001309716224362489*sin(2.0*t1)*cos(t4)*cos(t5)*sin(t2)*sin(t3) + 0.00042011718750000002619432448724979*cos(t1)*cos(t2)*cos(t3)*cos(t4)*cos(t5)*sin(t1) - 0.00042011718750000002619432448724979*cos(t1)*cos(t2)*cos(t5)*sin(t1)*sin(t3)*sin(t4) - 0.00042011718750000002619432448724979*cos(t1)*cos(t3)*cos(t5)*sin(t1)*sin(t2)*sin(t4) - 0.00042011718750000002619432448724979*cos(t1)*cos(t4)*cos(t5)*sin(t1)*sin(t2)*sin(t3)))
     td6*(td1*(0.00084023437500000005238864897449957*cos(t1)*cos(t5)*sin(t1) + 0.00042011718750000002619432448724979*cos(t1)^2*cos(t2)*cos(t3)*cos(t4)*sin(t5) - 0.00042011718750000002619432448724979*cos(t2)*cos(t3)*cos(t4)*sin(t1)^2*sin(t5) - 0.00042011718750000002619432448724979*cos(t1)^2*cos(t2)*sin(t3)*sin(t4)*sin(t5) - 0.00042011718750000002619432448724979*cos(t1)^2*cos(t3)*sin(t2)*sin(t4)*sin(t5) - 0.00042011718750000002619432448724979*cos(t1)^2*cos(t4)*sin(t2)*sin(t3)*sin(t5) + 0.00042011718750000002619432448724979*cos(t2)*sin(t1)^2*sin(t3)*sin(t4)*sin(t5) + 0.00042011718750000002619432448724979*cos(t3)*sin(t1)^2*sin(t2)*sin(t4)*sin(t5) + 0.00042011718750000002619432448724979*cos(t4)*sin(t1)^2*sin(t2)*sin(t3)*sin(t5)) + td6*(0.5*(0.00084023437500000005238864897449957*cos(t1)*cos(t2)*cos(t3)*sin(t4)*sin(t5) + 0.00084023437500000005238864897449957*cos(t1)*cos(t2)*cos(t4)*sin(t3)*sin(t5) + 0.00084023437500000005238864897449957*cos(t1)*cos(t3)*cos(t4)*sin(t2)*sin(t5) - 0.00084023437500000005238864897449957*cos(t1)*sin(t2)*sin(t3)*sin(t4)*sin(t5))*(cos(t1)*cos(t2)*sin(t3)*sin(t4)*sin(t5) - 1.0*cos(t1)*cos(t2)*cos(t3)*cos(t4)*sin(t5) - 1.0*cos(t5)*sin(t1) + cos(t1)*cos(t3)*sin(t2)*sin(t4)*sin(t5) + cos(t1)*cos(t4)*sin(t2)*sin(t3)*sin(t5)) + 0.5*(cos(t1)*cos(t2)*cos(t3)*sin(t4)*sin(t5) + cos(t1)*cos(t2)*cos(t4)*sin(t3)*sin(t5) + cos(t1)*cos(t3)*cos(t4)*sin(t2)*sin(t5) - 1.0*cos(t1)*sin(t2)*sin(t3)*sin(t4)*sin(t5))*(0.00084023437500000005238864897449957*cos(t1)*cos(t2)*sin(t3)*sin(t4)*sin(t5) - 0.00084023437500000005238864897449957*cos(t1)*cos(t2)*cos(t3)*cos(t4)*sin(t5) - 0.00084023437500000005238864897449957*cos(t5)*sin(t1) + 0.00084023437500000005238864897449957*cos(t1)*cos(t3)*sin(t2)*sin(t4)*sin(t5) + 0.00084023437500000005238864897449957*cos(t1)*cos(t4)*sin(t2)*sin(t3)*sin(t5)) + 0.5*(0.0016804687500000001047772979489991*cos(t2)*cos(t3)*sin(t1)*sin(t4)*sin(t5) + 0.0016804687500000001047772979489991*cos(t2)*cos(t4)*sin(t1)*sin(t3)*sin(t5) + 0.0016804687500000001047772979489991*cos(t3)*cos(t4)*sin(t1)*sin(t2)*sin(t5) - 0.0016804687500000001047772979489991*sin(t1)*sin(t2)*sin(t3)*sin(t4)*sin(t5))*(cos(t1)*cos(t5) - 1.0*cos(t2)*cos(t3)*cos(t4)*sin(t1)*sin(t5) + cos(t2)*sin(t1)*sin(t3)*sin(t4)*sin(t5) + cos(t3)*sin(t1)*sin(t2)*sin(t4)*sin(t5) + cos(t4)*sin(t1)*sin(t2)*sin(t3)*sin(t5)) + 0.5*(cos(t2)*cos(t3)*sin(t1)*sin(t4)*sin(t5) + cos(t2)*cos(t4)*sin(t1)*sin(t3)*sin(t5) + cos(t3)*cos(t4)*sin(t1)*sin(t2)*sin(t5) - 1.0*sin(t1)*sin(t2)*sin(t3)*sin(t4)*sin(t5))*(0.0016804687500000001047772979489991*cos(t1)*cos(t5) - 0.0016804687500000001047772979489991*cos(t2)*cos(t3)*cos(t4)*sin(t1)*sin(t5) + 0.0016804687500000001047772979489991*cos(t2)*sin(t1)*sin(t3)*sin(t4)*sin(t5) + 0.0016804687500000001047772979489991*cos(t3)*sin(t1)*sin(t2)*sin(t4)*sin(t5) + 0.0016804687500000001047772979489991*cos(t4)*sin(t1)*sin(t2)*sin(t3)*sin(t5))) - 1.0*td5*(0.00063017578125000003929148673087468*cos(2.0*t2)*cos(2.0*t3)*cos(2.0*t4)*sin(t5) - 0.00042011718750000002619432448724979*cos(t1)^2*sin(t5) - 0.00042011718750000002619432448724979*sin(t5) - 0.00063017578125000003929148673087468*cos(2.0*t2)*sin(2.0*t3)*sin(2.0*t4)*sin(t5) - 0.00063017578125000003929148673087468*cos(2.0*t3)*sin(2.0*t2)*sin(2.0*t4)*sin(t5) - 0.00063017578125000003929148673087468*cos(2.0*t4)*sin(2.0*t2)*sin(2.0*t3)*sin(t5) - 0.00021005859375000001309716224362489*cos(2.0*t1)*cos(2.0*t2)*cos(2.0*t3)*cos(2.0*t4)*sin(t5) + 0.00021005859375000001309716224362489*cos(2.0*t1)*cos(2.0*t2)*sin(2.0*t3)*sin(2.0*t4)*sin(t5) + 0.00021005859375000001309716224362489*cos(2.0*t1)*cos(2.0*t3)*sin(2.0*t2)*sin(2.0*t4)*sin(t5) + 0.00021005859375000001309716224362489*cos(2.0*t1)*cos(2.0*t4)*sin(2.0*t2)*sin(2.0*t3)*sin(t5) - 0.00021005859375000001309716224362489*sin(2.0*t1)*cos(t2)*cos(t3)*cos(t4)*cos(t5) + 0.00021005859375000001309716224362489*sin(2.0*t1)*cos(t2)*cos(t5)*sin(t3)*sin(t4) + 0.00021005859375000001309716224362489*sin(2.0*t1)*cos(t3)*cos(t5)*sin(t2)*sin(t4) + 0.00021005859375000001309716224362489*sin(2.0*t1)*cos(t4)*cos(t5)*sin(t2)*sin(t3) - 0.00042011718750000002619432448724979*cos(t1)*cos(t2)*cos(t3)*cos(t4)*cos(t5)*sin(t1) + 0.00042011718750000002619432448724979*cos(t1)*cos(t2)*cos(t5)*sin(t1)*sin(t3)*sin(t4) + 0.00042011718750000002619432448724979*cos(t1)*cos(t3)*cos(t5)*sin(t1)*sin(t2)*sin(t4) + 0.00042011718750000002619432448724979*cos(t1)*cos(t4)*cos(t5)*sin(t1)*sin(t2)*sin(t3))) - td2*(1.0*td2*(0.0029327291666666668173979459766088*cos(t3)*sin(t3) + 153408.0*m4*sin(t3) + 153408.0*m5*sin(t3) + 153408.0*m6*sin(t3) + 0.0029327291666666668173979459766088*cos(t1)*cos(t3)^2*sin(t1) - 0.0058654583333333336347958919532175*cos(t1)^2*cos(t3)*sin(t3) - 0.0029327291666666668173979459766088*cos(t1)*sin(t1)*sin(t3)^2 + 41820.0*m5*cos(t3)*sin(t4) + 41820.0*m5*cos(t4)*sin(t3) + 41820.0*m6*cos(t3)*sin(t4) + 41820.0*m6*cos(t4)*sin(t3) - 408.0*L4*m5*cos(t3)*sin(t4) - 408.0*L4*m5*cos(t4)*sin(t3) - 204.0*L3*m5*cos(t3)*cos(t4)*sin(t5) + 204.0*L3*m5*sin(t3)*sin(t4)*sin(t5)) - td1*(0.00073318229166666670434948649415219*sin(t1 - 2.0*t2) + 0.00073318229166666670434948649415219*sin(t1 + 2.0*t2) + 0.00024028885416666671912683250766918*sin(2.0*t1) - 0.00036659114583333335217474324707609*sin(2.0*t1 - 2.0*t2) - 0.00036659114583333335217474324707609*sin(2.0*t1 + 2.0*t2) - 0.0014663645833333334086989729883044*sin(2.0*t1 - 2.0*t3) + 52828.0*m4*sin(t2 + t3) + 52828.0*m5*sin(t2 + t3) + 52828.0*m6*sin(t2 + t3) + 14401.25*m5*sin(t2 + t3 + t4) + 14401.25*m6*sin(t2 + t3 + t4) + 94.0*L3*m5*sin(t2 + t3 + t5) - 140.5*L4*m5*sin(t2 + t3 + t4) + 60.75*L3*m5*sin(t2 + t3 + t4 - 1.0*t5) + 0.0625*L3^2*m5*sin(t2 + t3 + t4 - 2.0*t5) - 0.0625*L3^2*m5*sin(t2 + t3 + t4 + 2.0*t5) - 9.5*L3*m5*sin(t2 + t3 + t4 + t5) - 376.0*L1*m4*sin(t2 + t3) + 94.0*L3*m5*sin(t2 + t3 - 1.0*t5) - 0.25*L3*L4*m5*sin(t2 + t3 + t4 + t5) - 0.25*L3*L4*m5*sin(t2 + t3 + t4 - 1.0*t5)) + 1.0*td3*(0.0029327291666666668173979459766088*cos(t2)*sin(t2) - 0.0029327291666666668173979459766088*cos(t1)^2*cos(t2)*sin(t2)) + 1.0*td5*(0.00073318229166666670434948649415219*sin(3.0*t2 - 1.0*t1 + t3 + t4) - 0.0014663645833333334086989729883044*sin(t2 - 2.0*t1 + 3.0*t3 + t4) - 0.00036659114583333335217474324707609*sin(3.0*t2 - 2.0*t1 + t3 + t4) + 0.00036659114583333335217474324707609*sin(2.0*t1 + 3.0*t2 + t3 + t4) + 0.00057664973958333336527190549070099*sin(t2 - 2.0*t1 + t3 + t4) - 0.00057664973958333336527190549070099*sin(2.0*t1 + t2 + t3 + t4) - 0.00073318229166666670434948649415219*sin(t1 + 3.0*t2 + t3 + t4) + 94.0*L3*m5*sin(t4 - 1.0*t5) + 94.0*L3*m5*sin(t4 + t5) + 0.125*L3^2*m5*sin(2.0*t5)) - td6*(0.00084023437500000005238864897449957*cos(t1)*cos(t2)*cos(t3)*sin(t1)*sin(t4)*sin(t5) + 0.00084023437500000005238864897449957*cos(t1)*cos(t2)*cos(t4)*sin(t1)*sin(t3)*sin(t5) + 0.00084023437500000005238864897449957*cos(t1)*cos(t3)*cos(t4)*sin(t1)*sin(t2)*sin(t5) - 0.00084023437500000005238864897449957*cos(t1)*sin(t1)*sin(t2)*sin(t3)*sin(t4)*sin(t5)) + 1.0*td4*(- 0.0029327291666666668173979459766088*cos(t2)*sin(t2)*cos(t1)^2 + 0.0014663645833333334086989729883044*sin(2.0*t1 - 2.0*t3) + 0.0029327291666666668173979459766088*cos(t2)*sin(t2) - 38540.0*m5*sin(t4) - 38540.0*m6*sin(t4) - 94.0*L3*m5*sin(t4 - 1.0*t5) + 94.0*L3*m5*sin(t4 + t5) + 376.0*L4*m5*sin(t4))) - td1*(1.0*td6*(0.00084023437500000005238864897449957*cos(t1)*cos(t5)*sin(t1) + 0.00042011718750000002619432448724979*cos(t1)^2*cos(t2)*cos(t3)*cos(t4)*sin(t5) - 0.00042011718750000002619432448724979*cos(t2)*cos(t3)*cos(t4)*sin(t1)^2*sin(t5) - 0.00042011718750000002619432448724979*cos(t1)^2*cos(t2)*sin(t3)*sin(t4)*sin(t5) - 0.00042011718750000002619432448724979*cos(t1)^2*cos(t3)*sin(t2)*sin(t4)*sin(t5) - 0.00042011718750000002619432448724979*cos(t1)^2*cos(t4)*sin(t2)*sin(t3)*sin(t5) + 0.00042011718750000002619432448724979*cos(t2)*sin(t1)^2*sin(t3)*sin(t4)*sin(t5) + 0.00042011718750000002619432448724979*cos(t3)*sin(t1)^2*sin(t2)*sin(t4)*sin(t5) + 0.00042011718750000002619432448724979*cos(t4)*sin(t1)^2*sin(t2)*sin(t3)*sin(t5)) - td3*(- 0.0029327291666666668173979459766088*sin(t3)*cos(t1)^2*cos(t3) + 0.0029327291666666668173979459766088*cos(t1)*cos(t2)^2*sin(t1) + 0.0058654583333333336347958919532175*cos(t1)*cos(t3)^2*sin(t1) - 0.0048796714583333336643505839802515*cos(t1)*sin(t1) + 0.0029327291666666668173979459766088*sin(t3)*cos(t3)*sin(t1)^2) - td4*(- 0.0029327291666666668173979459766088*sin(t3)*cos(t1)^2*cos(t3) + 0.0029327291666666668173979459766088*cos(t1)*cos(t2)^2*sin(t1) + 0.0058654583333333336347958919532175*cos(t1)*cos(t3)^2*sin(t1) - 0.0067056927083333336871845409277171*cos(t1)*sin(t1) + 0.0029327291666666668173979459766088*sin(t3)*cos(t3)*sin(t1)^2) - td1*(76704.0*m4*sin(2.0*t2 + t3) + 76704.0*m5*sin(2.0*t2 + t3) + 76704.0*m6*sin(2.0*t2 + t3) + 38540.0*m5*sin(2.0*t2 + 2.0*t3 + t4) + 38540.0*m6*sin(2.0*t2 + 2.0*t3 + t4) - 20910.0*m5*sin(t3 + t4) - 20910.0*m6*sin(t3 + t4) + 20910.0*m5*sin(2.0*t2 + t3 + t4) + 20910.0*m6*sin(2.0*t2 + t3 + t4) - 76704.0*m4*sin(t3) - 76704.0*m5*sin(t3) - 76704.0*m6*sin(t3) + 70688.0*m4*sin(2.0*t2 + 2.0*t3) + 70688.0*m5*sin(2.0*t2 + 2.0*t3) + 70688.0*m6*sin(2.0*t2 + 2.0*t3) + 5253.125*m5*sin(2.0*t2 + 2.0*t3 + 2.0*t4) + 5253.125*m6*sin(2.0*t2 + 2.0*t3 + 2.0*t4) - 102.5*L4*m5*sin(2.0*t2 + 2.0*t3 + 2.0*t4) + 25.625*L3*m5*sin(2.0*t2 + 2.0*t3 + 2.0*t4 - 1.0*t5) + 51.0*L3*m5*sin(t3 + t4 + t5) - 51.0*L3*m5*sin(2.0*t2 + t3 + t4 + t5) - 0.0625*L3^2*m5*sin(2.0*t2 + 2.0*t3 + 2.0*t4) + 0.5*L4^2*m5*sin(2.0*t2 + 2.0*t3 + 2.0*t4) - 376.0*L4*m5*sin(2.0*t2 + 2.0*t3 + t4) + 0.03125*L3^2*m5*sin(2.0*t2 + 2.0*t3 + 2.0*t4 - 2.0*t5) + 0.03125*L3^2*m5*sin(2.0*t2 + 2.0*t3 + 2.0*t4 + 2.0*t5) + 94.0*L3*m5*sin(2.0*t2 + 2.0*t3 + t4 - 1.0*t5) - 25.625*L3*m5*sin(2.0*t2 + 2.0*t3 + 2.0*t4 + t5) + 204.0*L4*m5*sin(t3 + t4) - 204.0*L4*m5*sin(2.0*t2 + t3 + t4) - 51.0*L3*m5*sin(t3 + t4 - 1.0*t5) + 51.0*L3*m5*sin(2.0*t2 + t3 + t4 - 1.0*t5) - 94.0*L3*m5*sin(2.0*t2 + 2.0*t3 + t4 + t5) - 0.25*L3*L4*m5*sin(2.0*t2 + 2.0*t3 + 2.0*t4 - 1.0*t5) + 0.25*L3*L4*m5*sin(2.0*t2 + 2.0*t3 + 2.0*t4 + t5)) + td5*(0.00073318229166666670434948649415219*sin(t2 - 2.0*t1 + 3.0*t3 + t4) + 0.00018329557291666667608737162353805*sin(3.0*t2 - 2.0*t1 + t3 + t4) + 0.00018329557291666667608737162353805*sin(2.0*t1 + 3.0*t2 + t3 + t4) + 0.00073318229166666670434948649415219*sin(t2 + t3 + t4) - 0.00057664973958333336527190549070099*sin(t2 - 2.0*t1 + t3 + t4) - 0.00057664973958333336527190549070099*sin(2.0*t1 + t2 + t3 + t4) - 0.00018329557291666667608737162353805*sin(2.0*t1 + t2 - 1.0*t3 - 1.0*t4) - 0.00036659114583333335217474324707609*sin(t3 - 1.0*t2 + t4) + 0.00073318229166666670434948649415219*sin(2.0*t1 + t2 - 1.0*t3 + t4) + 0.00018329557291666667608737162353805*sin(2.0*t1 - 1.0*t2 + t3 + t4) - 0.00036659114583333335217474324707609*sin(3.0*t2 + t3 + t4) + 94.0*L3*m5*sin(t2 + t3 + t5) - 25.625*L3*m5*sin(t2 + t3 + t4 - 1.0*t5) + 0.125*L3^2*m5*sin(t2 + t3 + t4) - 0.0625*L3^2*m5*sin(t2 + t3 + t4 - 2.0*t5) - 0.0625*L3^2*m5*sin(t2 + t3 + t4 + 2.0*t5) + 25.625*L3*m5*sin(t2 + t3 + t4 + t5) - 94.0*L3*m5*sin(t2 + t3 - 1.0*t5) - 0.25*L3*L4*m5*sin(t2 + t3 + t4 + t5) + 0.25*L3*L4*m5*sin(t2 + t3 + t4 - 1.0*t5)) + 1.0*td2*(0.00073318229166666670434948649415219*sin(t1 - 2.0*t2) + 0.00073318229166666670434948649415219*sin(t1 + 2.0*t2) + 0.00024028885416666671912683250766918*sin(2.0*t1) - 0.00036659114583333335217474324707609*sin(2.0*t1 - 2.0*t2) - 0.00036659114583333335217474324707609*sin(2.0*t1 + 2.0*t2) - 0.0014663645833333334086989729883044*sin(2.0*t1 - 2.0*t3))) + td5*(td5*(0.00036659114583333335217474324707609*sin(2.0*t3 - 1.0*t1 + 2.0*t4) + 0.000091647786458333338043685811769024*sin(2.0*t3 - 2.0*t1 + 2.0*t4) + 0.000091647786458333338043685811769024*sin(2.0*t1 + 2.0*t3 + 2.0*t4) + 0.001729949218750000095815716472103*sin(2.0*t2 + 2.0*t3 + 2.0*t4) + 0.00054988671875000002826211487061414*sin(4.0*t2 + 2.0*t3 + 2.0*t4) - 0.00036659114583333335217474324707609*sin(4.0*t2 - 1.0*t1 + 2.0*t3 + 2.0*t4) - 0.00028832486979166668263595274535049*sin(2.0*t2 - 2.0*t1 + 2.0*t3 + 2.0*t4) - 0.00028832486979166668263595274535049*sin(2.0*t1 + 2.0*t2 + 2.0*t3 + 2.0*t4) + 0.00073318229166666670434948649415219*sin(2.0*t2 - 2.0*t1 + 4.0*t3 + 2.0*t4) + 0.000091647786458333338043685811769024*sin(4.0*t2 - 2.0*t1 + 2.0*t3 + 2.0*t4) + 0.000091647786458333338043685811769024*sin(2.0*t1 + 4.0*t2 + 2.0*t3 + 2.0*t4) + 0.00036659114583333335217474324707609*sin(t1 + 2.0*t3 + 2.0*t4) - 0.00036659114583333335217474324707609*sin(t1 + 4.0*t2 + 2.0*t3 + 2.0*t4) + 0.00073318229166666670434948649415219*sin(2.0*t1 - 2.0*t3) + 0.00054988671875000002826211487061414*sin(2.0*t3 + 2.0*t4)) - 1.0*td1*(0.00036659114583333335217474324707609*sin(3.0*t2 - 1.0*t1 + t3 + t4) - 0.00073318229166666670434948649415219*sin(t2 - 2.0*t1 + 3.0*t3 + t4) - 0.00018329557291666667608737162353805*sin(3.0*t2 - 2.0*t1 + t3 + t4) - 0.00018329557291666667608737162353805*sin(2.0*t1 + 3.0*t2 + t3 + t4) + 0.00073318229166666670434948649415219*sin(t2 + t3 + t4) - 0.00036659114583333335217474324707609*sin(t1 - 1.0*t2 + t3 + t4) + 0.00057664973958333336527190549070099*sin(t2 - 2.0*t1 + t3 + t4) + 0.00057664973958333336527190549070099*sin(2.0*t1 + t2 + t3 + t4) + 0.00036659114583333335217474324707609*sin(t1 + 3.0*t2 + t3 + t4) + 0.00018329557291666667608737162353805*sin(2.0*t1 + t2 - 1.0*t3 - 1.0*t4) - 0.00036659114583333335217474324707609*sin(t3 - 1.0*t2 + t4) + 0.00036659114583333335217474324707609*sin(t1 + t2 - 1.0*t3 - 1.0*t4) - 0.00073318229166666670434948649415219*sin(2.0*t1 + t2 - 1.0*t3 + t4) - 0.00018329557291666667608737162353805*sin(2.0*t1 - 1.0*t2 + t3 + t4) - 0.00036659114583333335217474324707609*sin(3.0*t2 + t3 + t4) + 35.125*L3*m5*sin(t2 + t3 + t4 - 1.0*t5) + 0.125*L3^2*m5*sin(t2 + t3 + t4) + 0.0625*L3^2*m5*sin(t2 + t3 + t4 - 2.0*t5) + 0.0625*L3^2*m5*sin(t2 + t3 + t4 + 2.0*t5) + 35.125*L3*m5*sin(t2 + t3 + t4 + t5)) + td4*(0.00073318229166666670434948649415219*sin(t2 - 2.0*t1 + 3.0*t3 + t4) + 0.00073318229166666670434948649415219*sin(2.0*t1 + t2 - 1.0*t3 + t4) - 47.0*L3*m5*sin(t4 - 1.0*t5) - 47.0*L3*m5*sin(t4 + t5) + 0.25*L3^2*m5*cos(t5)*sin(t5) + 94.0*L3*m5*cos(t5)*sin(t4)) + td2*(0.00036659114583333335217474324707609*sin(3.0*t2 - 1.0*t1 + t3 + t4) + 0.00073318229166666670434948649415219*sin(t2 - 2.0*t1 + 3.0*t3 + t4) - 0.00018329557291666667608737162353805*sin(3.0*t2 - 2.0*t1 + t3 + t4) + 0.00018329557291666667608737162353805*sin(2.0*t1 + 3.0*t2 + t3 + t4) - 0.00036659114583333335217474324707609*sin(t1 - 1.0*t2 + t3 + t4) - 0.00036659114583333335217474324707609*sin(t1 + 3.0*t2 + t3 + t4) - 0.00018329557291666667608737162353805*sin(2.0*t1 + t2 - 1.0*t3 - 1.0*t4) - 0.00036659114583333335217474324707609*sin(t1 + t2 - 1.0*t3 - 1.0*t4) + 0.00073318229166666670434948649415219*sin(2.0*t1 + t2 - 1.0*t3 + t4) - 0.00018329557291666667608737162353805*sin(2.0*t1 - 1.0*t2 + t3 + t4) + 102.0*L3*m5*sin(t3 + t4 + t5) + 94.0*L3*m5*sin(t4 - 1.0*t5) + 94.0*L3*m5*sin(t4 + t5) + 102.0*L3*m5*sin(t3 + t4 - 1.0*t5) + 0.125*L3^2*m5*sin(2.0*t5)) + td3*(0.25*m5*cos(t5)*sin(t5)*L3^2 + 188.0*m5*cos(t5)*sin(t4)*L3) - 1.0*td6*(0.00042011718750000002619432448724979*sin(t5) + 0.00042011718750000002619432448724979*cos(t1)^2*sin(t5) + 0.00063017578125000003929148673087468*cos(2.0*t2)*cos(2.0*t3)*cos(2.0*t4)*sin(t5) - 0.00063017578125000003929148673087468*cos(2.0*t2)*sin(2.0*t3)*sin(2.0*t4)*sin(t5) - 0.00063017578125000003929148673087468*cos(2.0*t3)*sin(2.0*t2)*sin(2.0*t4)*sin(t5) - 0.00063017578125000003929148673087468*cos(2.0*t4)*sin(2.0*t2)*sin(2.0*t3)*sin(t5) - 0.00021005859375000001309716224362489*cos(2.0*t1)*cos(2.0*t2)*cos(2.0*t3)*cos(2.0*t4)*sin(t5) + 0.00021005859375000001309716224362489*cos(2.0*t1)*cos(2.0*t2)*sin(2.0*t3)*sin(2.0*t4)*sin(t5) + 0.00021005859375000001309716224362489*cos(2.0*t1)*cos(2.0*t3)*sin(2.0*t2)*sin(2.0*t4)*sin(t5) + 0.00021005859375000001309716224362489*cos(2.0*t1)*cos(2.0*t4)*sin(2.0*t2)*sin(2.0*t3)*sin(t5) - 0.00021005859375000001309716224362489*sin(2.0*t1)*cos(t2)*cos(t3)*cos(t4)*cos(t5) + 0.00021005859375000001309716224362489*sin(2.0*t1)*cos(t2)*cos(t5)*sin(t3)*sin(t4) + 0.00021005859375000001309716224362489*sin(2.0*t1)*cos(t3)*cos(t5)*sin(t2)*sin(t4) + 0.00021005859375000001309716224362489*sin(2.0*t1)*cos(t4)*cos(t5)*sin(t2)*sin(t3) + 0.00042011718750000002619432448724979*cos(t1)*cos(t2)*cos(t3)*cos(t4)*cos(t5)*sin(t1) - 0.00042011718750000002619432448724979*cos(t1)*cos(t2)*cos(t5)*sin(t1)*sin(t3)*sin(t4) - 0.00042011718750000002619432448724979*cos(t1)*cos(t3)*cos(t5)*sin(t1)*sin(t2)*sin(t4) - 0.00042011718750000002619432448724979*cos(t1)*cos(t4)*cos(t5)*sin(t1)*sin(t2)*sin(t3))) - td3*(1.0*td2*(0.0029327291666666668173979459766088*cos(t2)*sin(t2)*cos(t1)^2 + 0.0029327291666666668173979459766088*sin(2.0*t1 - 2.0*t3) - 0.0029327291666666668173979459766088*cos(t2)*sin(t2) + 41820.0*m5*sin(t3 + t4) + 41820.0*m6*sin(t3 + t4) + 153408.0*m4*sin(t3) + 153408.0*m5*sin(t3) + 153408.0*m6*sin(t3) - 102.0*L3*m5*sin(t3 + t4 + t5) - 408.0*L4*m5*sin(t3 + t4) + 102.0*L3*m5*sin(t3 + t4 - 1.0*t5)) + 1.0*td4*(- 0.011730916666666667269591783906435*cos(t1)^2*cos(t3)*sin(t3) + 0.0058654583333333336347958919532175*sin(t1)*cos(t1)*cos(t3)^2 - 0.0058654583333333336347958919532175*sin(t1)*cos(t1)*sin(t3)^2 + 0.0058654583333333336347958919532175*cos(t3)*sin(t3) - 38540.0*m5*sin(t4) - 38540.0*m6*sin(t4) + 376.0*L4*m5*sin(t4) + 188.0*L3*m5*cos(t4)*sin(t5)) - td6*(0.00084023437500000005238864897449957*cos(t1)*cos(t2)*cos(t3)*sin(t1)*sin(t4)*sin(t5) + 0.00084023437500000005238864897449957*cos(t1)*cos(t2)*cos(t4)*sin(t1)*sin(t3)*sin(t5) + 0.00084023437500000005238864897449957*cos(t1)*cos(t3)*cos(t4)*sin(t1)*sin(t2)*sin(t5) - 0.00084023437500000005238864897449957*cos(t1)*sin(t1)*sin(t2)*sin(t3)*sin(t4)*sin(t5)) - td1*(0.0048796714583333336643505839802515*cos(t1)*sin(t1) + 52828.0*m4*sin(t2 + t3) + 52828.0*m5*sin(t2 + t3) + 52828.0*m6*sin(t2 + t3) + 14401.25*m5*sin(t2 + t3 + t4) + 14401.25*m6*sin(t2 + t3 + t4) + 94.0*L3*m5*sin(t2 + t3 + t5) - 140.5*L4*m5*sin(t2 + t3 + t4) - 0.0029327291666666668173979459766088*cos(t1)*cos(t2)^2*sin(t1) - 0.0058654583333333336347958919532175*cos(t1)*cos(t3)^2*sin(t1) + 0.0029327291666666668173979459766088*cos(t1)^2*cos(t3)*sin(t3) + 60.75*L3*m5*sin(t2 + t3 + t4 - 1.0*t5) - 0.0029327291666666668173979459766088*cos(t3)*sin(t1)^2*sin(t3) + 0.0625*L3^2*m5*sin(t2 + t3 + t4 - 2.0*t5) - 0.0625*L3^2*m5*sin(t2 + t3 + t4 + 2.0*t5) - 9.5*L3*m5*sin(t2 + t3 + t4 + t5) - 376.0*L1*m4*sin(t2 + t3) + 94.0*L3*m5*sin(t2 + t3 - 1.0*t5) - 0.25*L3*L4*m5*sin(t2 + t3 + t4 + t5) - 0.25*L3*L4*m5*sin(t2 + t3 + t4 - 1.0*t5)) + 1.0*td3*(- 0.0058654583333333336347958919532175*cos(t1)^2*cos(t3)*sin(t3) + 0.0029327291666666668173979459766088*sin(t1)*cos(t1)*cos(t3)^2 - 0.0029327291666666668173979459766088*sin(t1)*cos(t1)*sin(t3)^2 + 0.0029327291666666668173979459766088*cos(t3)*sin(t3)) + 1.0*td5*(0.25*m5*cos(t5)*sin(t5)*L3^2 + 188.0*m5*cos(t5)*sin(t4)*L3 + 0.00036659114583333335217474324707609*sin(3.0*t2 - 1.0*t1 + t3 + t4) - 0.0021995468750000001130484594824566*sin(t2 - 2.0*t1 + 3.0*t3 + t4) - 0.00018329557291666667608737162353805*sin(3.0*t2 - 2.0*t1 + t3 + t4) + 0.00018329557291666667608737162353805*sin(2.0*t1 + 3.0*t2 + t3 + t4) + 0.00036659114583333335217474324707609*sin(t1 - 1.0*t2 + t3 + t4) + 0.00057664973958333336527190549070099*sin(t2 - 2.0*t1 + t3 + t4) - 0.00057664973958333336527190549070099*sin(2.0*t1 + t2 + t3 + t4) - 0.00036659114583333335217474324707609*sin(t1 + 3.0*t2 + t3 + t4) + 0.00018329557291666667608737162353805*sin(2.0*t1 + t2 - 1.0*t3 - 1.0*t4) + 0.00036659114583333335217474324707609*sin(t1 + t2 - 1.0*t3 - 1.0*t4) - 0.00073318229166666670434948649415219*sin(2.0*t1 + t2 - 1.0*t3 + t4) + 0.00018329557291666667608737162353805*sin(2.0*t1 - 1.0*t2 + t3 + t4))) - td4*(1.0*td1*(140.5*L4*m5*sin(t2 + t3 + t4) - 14401.25*m5*sin(t2 + t3 + t4) - 14401.25*m6*sin(t2 + t3 + t4) - 0.0067056927083333336871845409277171*cos(t1)*sin(t1) + 0.0029327291666666668173979459766088*cos(t1)*cos(t2)^2*sin(t1) + 0.0058654583333333336347958919532175*cos(t1)*cos(t3)^2*sin(t1) - 0.0029327291666666668173979459766088*cos(t1)^2*cos(t3)*sin(t3) - 60.75*L3*m5*sin(t2 + t3 + t4 - 1.0*t5) + 0.0029327291666666668173979459766088*cos(t3)*sin(t1)^2*sin(t3) - 0.0625*L3^2*m5*sin(t2 + t3 + t4 - 2.0*t5) + 0.0625*L3^2*m5*sin(t2 + t3 + t4 + 2.0*t5) + 9.5*L3*m5*sin(t2 + t3 + t4 + t5) + 0.25*L3*L4*m5*sin(t2 + t3 + t4 + t5) + 0.25*L3*L4*m5*sin(t2 + t3 + t4 - 1.0*t5)) + 1.0*td2*(0.0029327291666666668173979459766088*cos(t2)*sin(t2)*cos(t1)^2 + 0.0014663645833333334086989729883044*sin(2.0*t1 - 2.0*t3) - 0.0029327291666666668173979459766088*cos(t2)*sin(t2) + 41820.0*m5*sin(t3 + t4) + 41820.0*m6*sin(t3 + t4) + 38540.0*m5*sin(t4) + 38540.0*m6*sin(t4) - 102.0*L3*m5*sin(t3 + t4 + t5) + 94.0*L3*m5*sin(t4 - 1.0*t5) - 408.0*L4*m5*sin(t3 + t4) - 94.0*L3*m5*sin(t4 + t5) + 102.0*L3*m5*sin(t3 + t4 - 1.0*t5) - 376.0*L4*m5*sin(t4)) + 1.0*td5*(0.00036659114583333335217474324707609*sin(3.0*t2 - 1.0*t1 + t3 + t4) - 0.0014663645833333334086989729883044*sin(t2 - 2.0*t1 + 3.0*t3 + t4) - 0.00018329557291666667608737162353805*sin(3.0*t2 - 2.0*t1 + t3 + t4) + 0.00018329557291666667608737162353805*sin(2.0*t1 + 3.0*t2 + t3 + t4) + 0.00036659114583333335217474324707609*sin(t1 - 1.0*t2 + t3 + t4) + 0.00057664973958333336527190549070099*sin(t2 - 2.0*t1 + t3 + t4) - 0.00057664973958333336527190549070099*sin(2.0*t1 + t2 + t3 + t4) - 0.00036659114583333335217474324707609*sin(t1 + 3.0*t2 + t3 + t4) + 0.00018329557291666667608737162353805*sin(2.0*t1 + t2 - 1.0*t3 - 1.0*t4) + 0.00036659114583333335217474324707609*sin(t1 + t2 - 1.0*t3 - 1.0*t4) + 0.00018329557291666667608737162353805*sin(2.0*t1 - 1.0*t2 + t3 + t4) - 47.0*L3*m5*sin(t4 - 1.0*t5) - 47.0*L3*m5*sin(t4 + t5) + 0.25*L3^2*m5*cos(t5)*sin(t5) + 94.0*L3*m5*cos(t5)*sin(t4)) - td6*(0.00084023437500000005238864897449957*cos(t1)*cos(t2)*cos(t3)*sin(t1)*sin(t4)*sin(t5) + 0.00084023437500000005238864897449957*cos(t1)*cos(t2)*cos(t4)*sin(t1)*sin(t3)*sin(t5) + 0.00084023437500000005238864897449957*cos(t1)*cos(t3)*cos(t4)*sin(t1)*sin(t2)*sin(t5) - 0.00084023437500000005238864897449957*cos(t1)*sin(t1)*sin(t2)*sin(t3)*sin(t4)*sin(t5)) - td4*(0.0014663645833333334086989729883044*cos(2.0*t1)*sin(2.0*t3) - 0.0014663645833333334086989729883044*cos(2.0*t3)*sin(2.0*t1)) + 1.0*td3*(38540.0*m5*sin(t4) + 38540.0*m6*sin(t4) - 376.0*L4*m5*sin(t4) - 188.0*L3*m5*cos(t4)*sin(t5)))
     td5*(td5*(0.00036659114583333335217474324707609*sin(2.0*t3 - 1.0*t1 + 2.0*t4) + 0.00036659114583333335217474324707609*sin(2.0*t1 + 2.0*t2 + 2.0*t4) + 0.000091647786458333338043685811769024*sin(2.0*t3 - 2.0*t1 + 2.0*t4) + 0.000091647786458333338043685811769024*sin(2.0*t1 + 2.0*t3 + 2.0*t4) + 0.001729949218750000095815716472103*sin(2.0*t2 + 2.0*t3 + 2.0*t4) + 0.00054988671875000002826211487061414*sin(4.0*t2 + 2.0*t3 + 2.0*t4) - 0.00036659114583333335217474324707609*sin(4.0*t2 - 1.0*t1 + 2.0*t3 + 2.0*t4) - 0.00028832486979166668263595274535049*sin(2.0*t2 - 2.0*t1 + 2.0*t3 + 2.0*t4) - 0.00028832486979166668263595274535049*sin(2.0*t1 + 2.0*t2 + 2.0*t3 + 2.0*t4) + 0.00036659114583333335217474324707609*sin(2.0*t2 - 2.0*t1 + 4.0*t3 + 2.0*t4) + 0.000091647786458333338043685811769024*sin(4.0*t2 - 2.0*t1 + 2.0*t3 + 2.0*t4) + 0.000091647786458333338043685811769024*sin(2.0*t1 + 4.0*t2 + 2.0*t3 + 2.0*t4) + 0.00036659114583333335217474324707609*sin(t1 + 2.0*t3 + 2.0*t4) - 0.00036659114583333335217474324707609*sin(t1 + 4.0*t2 + 2.0*t3 + 2.0*t4) + 0.00054988671875000002826211487061414*sin(2.0*t3 + 2.0*t4)) - 1.0*td1*(0.00036659114583333335217474324707609*sin(3.0*t2 - 1.0*t1 + t3 + t4) - 0.00073318229166666670434948649415219*sin(t2 - 2.0*t1 + 3.0*t3 + t4) - 0.00018329557291666667608737162353805*sin(3.0*t2 - 2.0*t1 + t3 + t4) - 0.00018329557291666667608737162353805*sin(2.0*t1 + 3.0*t2 + t3 + t4) + 0.00073318229166666670434948649415219*sin(t2 + t3 + t4) - 0.00036659114583333335217474324707609*sin(t1 - 1.0*t2 + t3 + t4) + 0.00057664973958333336527190549070099*sin(t2 - 2.0*t1 + t3 + t4) + 0.00057664973958333336527190549070099*sin(2.0*t1 + t2 + t3 + t4) + 0.00036659114583333335217474324707609*sin(t1 + 3.0*t2 + t3 + t4) + 0.00018329557291666667608737162353805*sin(2.0*t1 + t2 - 1.0*t3 - 1.0*t4) - 0.00036659114583333335217474324707609*sin(t3 - 1.0*t2 + t4) + 0.00036659114583333335217474324707609*sin(t1 + t2 - 1.0*t3 - 1.0*t4) - 0.00073318229166666670434948649415219*sin(2.0*t1 + t2 - 1.0*t3 + t4) - 0.00018329557291666667608737162353805*sin(2.0*t1 - 1.0*t2 + t3 + t4) - 0.00036659114583333335217474324707609*sin(3.0*t2 + t3 + t4) + 35.125*L3*m5*sin(t2 + t3 + t4 - 1.0*t5) + 0.125*L3^2*m5*sin(t2 + t3 + t4) + 0.0625*L3^2*m5*sin(t2 + t3 + t4 - 2.0*t5) + 0.0625*L3^2*m5*sin(t2 + t3 + t4 + 2.0*t5) + 35.125*L3*m5*sin(t2 + t3 + t4 + t5)) + td3*(47.0*L3*m5*sin(t4 - 1.0*t5) - 0.00073318229166666670434948649415219*sin(2.0*t1 + t2 - 1.0*t3 + t4) - 0.00073318229166666670434948649415219*sin(t2 - 2.0*t1 + 3.0*t3 + t4) + 47.0*L3*m5*sin(t4 + t5) + 0.25*L3^2*m5*cos(t5)*sin(t5) + 94.0*L3*m5*cos(t5)*sin(t4)) + td2*(0.00036659114583333335217474324707609*sin(3.0*t2 - 1.0*t1 + t3 + t4) - 0.00018329557291666667608737162353805*sin(3.0*t2 - 2.0*t1 + t3 + t4) + 0.00018329557291666667608737162353805*sin(2.0*t1 + 3.0*t2 + t3 + t4) - 0.00036659114583333335217474324707609*sin(t1 - 1.0*t2 + t3 + t4) - 0.00036659114583333335217474324707609*sin(t1 + 3.0*t2 + t3 + t4) - 0.00018329557291666667608737162353805*sin(2.0*t1 + t2 - 1.0*t3 - 1.0*t4) - 0.00036659114583333335217474324707609*sin(t1 + t2 - 1.0*t3 - 1.0*t4) - 0.00018329557291666667608737162353805*sin(2.0*t1 - 1.0*t2 + t3 + t4) + 102.0*L3*m5*sin(t3 + t4 + t5) + 94.0*L3*m5*sin(t4 - 1.0*t5) + 94.0*L3*m5*sin(t4 + t5) + 102.0*L3*m5*sin(t3 + t4 - 1.0*t5) + 0.125*L3^2*m5*sin(2.0*t5)) - 1.0*td6*(0.00042011718750000002619432448724979*sin(t5) + 0.00042011718750000002619432448724979*cos(t1)^2*sin(t5) + 0.00063017578125000003929148673087468*cos(2.0*t2)*cos(2.0*t3)*cos(2.0*t4)*sin(t5) - 0.00063017578125000003929148673087468*cos(2.0*t2)*sin(2.0*t3)*sin(2.0*t4)*sin(t5) - 0.00063017578125000003929148673087468*cos(2.0*t3)*sin(2.0*t2)*sin(2.0*t4)*sin(t5) - 0.00063017578125000003929148673087468*cos(2.0*t4)*sin(2.0*t2)*sin(2.0*t3)*sin(t5) - 0.00021005859375000001309716224362489*cos(2.0*t1)*cos(2.0*t2)*cos(2.0*t3)*cos(2.0*t4)*sin(t5) + 0.00021005859375000001309716224362489*cos(2.0*t1)*cos(2.0*t2)*sin(2.0*t3)*sin(2.0*t4)*sin(t5) + 0.00021005859375000001309716224362489*cos(2.0*t1)*cos(2.0*t3)*sin(2.0*t2)*sin(2.0*t4)*sin(t5) + 0.00021005859375000001309716224362489*cos(2.0*t1)*cos(2.0*t4)*sin(2.0*t2)*sin(2.0*t3)*sin(t5) - 0.00021005859375000001309716224362489*sin(2.0*t1)*cos(t2)*cos(t3)*cos(t4)*cos(t5) + 0.00021005859375000001309716224362489*sin(2.0*t1)*cos(t2)*cos(t5)*sin(t3)*sin(t4) + 0.00021005859375000001309716224362489*sin(2.0*t1)*cos(t3)*cos(t5)*sin(t2)*sin(t4) + 0.00021005859375000001309716224362489*sin(2.0*t1)*cos(t4)*cos(t5)*sin(t2)*sin(t3) + 0.00042011718750000002619432448724979*cos(t1)*cos(t2)*cos(t3)*cos(t4)*cos(t5)*sin(t1) - 0.00042011718750000002619432448724979*cos(t1)*cos(t2)*cos(t5)*sin(t1)*sin(t3)*sin(t4) - 0.00042011718750000002619432448724979*cos(t1)*cos(t3)*cos(t5)*sin(t1)*sin(t2)*sin(t4) - 0.00042011718750000002619432448724979*cos(t1)*cos(t4)*cos(t5)*sin(t1)*sin(t2)*sin(t3)) + 0.125*L3^2*m5*td4*sin(2.0*t5)) - td4*(1.0*td3*(0.0014663645833333334086989729883044*cos(2.0*t1)*sin(2.0*t3) - 0.0014663645833333334086989729883044*cos(2.0*t3)*sin(2.0*t1) + 38540.0*m5*sin(t4) + 38540.0*m6*sin(t4) - 376.0*L4*m5*sin(t4) - 188.0*L3*m5*cos(t4)*sin(t5)) + 1.0*td2*(0.00073318229166666670434948649415219*cos(2.0*t1)*sin(2.0*t2) - 0.00073318229166666670434948649415219*sin(2.0*t2) + 41820.0*m5*sin(t3 + t4) + 41820.0*m6*sin(t3 + t4) + 38540.0*m5*sin(t4) + 38540.0*m6*sin(t4) - 102.0*L3*m5*sin(t3 + t4 + t5) + 94.0*L3*m5*sin(t4 - 1.0*t5) - 408.0*L4*m5*sin(t3 + t4) - 94.0*L3*m5*sin(t4 + t5) + 102.0*L3*m5*sin(t3 + t4 - 1.0*t5) - 376.0*L4*m5*sin(t4)) - td6*(0.00084023437500000005238864897449957*cos(t1)*cos(t2)*cos(t3)*sin(t1)*sin(t4)*sin(t5) + 0.00084023437500000005238864897449957*cos(t1)*cos(t2)*cos(t4)*sin(t1)*sin(t3)*sin(t5) + 0.00084023437500000005238864897449957*cos(t1)*cos(t3)*cos(t4)*sin(t1)*sin(t2)*sin(t5) - 0.00084023437500000005238864897449957*cos(t1)*sin(t1)*sin(t2)*sin(t3)*sin(t4)*sin(t5)) + 1.0*td5*(0.125*m5*sin(2.0*t5)*L3^2 + 0.00036659114583333335217474324707609*sin(3.0*t2 - 1.0*t1 + t3 + t4) - 0.00073318229166666670434948649415219*sin(t2 - 2.0*t1 + 3.0*t3 + t4) - 0.00018329557291666667608737162353805*sin(3.0*t2 - 2.0*t1 + t3 + t4) + 0.00018329557291666667608737162353805*sin(2.0*t1 + 3.0*t2 + t3 + t4) + 0.00036659114583333335217474324707609*sin(t1 - 1.0*t2 + t3 + t4) + 0.00057664973958333336527190549070099*sin(t2 - 2.0*t1 + t3 + t4) - 0.00057664973958333336527190549070099*sin(2.0*t1 + t2 + t3 + t4) - 0.00036659114583333335217474324707609*sin(t1 + 3.0*t2 + t3 + t4) + 0.00018329557291666667608737162353805*sin(2.0*t1 + t2 - 1.0*t3 - 1.0*t4) + 0.00036659114583333335217474324707609*sin(t1 + t2 - 1.0*t3 - 1.0*t4) + 0.00073318229166666670434948649415219*sin(2.0*t1 + t2 - 1.0*t3 + t4) + 0.00018329557291666667608737162353805*sin(2.0*t1 - 1.0*t2 + t3 + t4)) + 1.0*td1*(0.00073318229166666670434948649415219*cos(2.0*t2)*sin(2.0*t1) - 0.001153299479166666730543810981402*sin(2.0*t1) - 0.0014663645833333334086989729883044*cos(2.0*t1)*sin(2.0*t3) + 0.0014663645833333334086989729883044*cos(2.0*t3)*sin(2.0*t1) - 14401.25*m5*sin(t2 + t3 + t4) - 14401.25*m6*sin(t2 + t3 + t4) + 140.5*L4*m5*sin(t2 + t3 + t4) - 60.75*L3*m5*sin(t2 + t3 + t4 - 1.0*t5) - 0.0625*L3^2*m5*sin(t2 + t3 + t4 - 2.0*t5) + 0.0625*L3^2*m5*sin(t2 + t3 + t4 + 2.0*t5) + 9.5*L3*m5*sin(t2 + t3 + t4 + t5) + 0.25*L3*L4*m5*sin(t2 + t3 + t4 + t5) + 0.25*L3*L4*m5*sin(t2 + t3 + t4 - 1.0*t5))) + td6*(td1*(0.00084023437500000005238864897449957*cos(t1)*cos(t5)*sin(t1) + 0.00042011718750000002619432448724979*cos(t1)^2*cos(t2)*cos(t3)*cos(t4)*sin(t5) - 0.00042011718750000002619432448724979*cos(t2)*cos(t3)*cos(t4)*sin(t1)^2*sin(t5) - 0.00042011718750000002619432448724979*cos(t1)^2*cos(t2)*sin(t3)*sin(t4)*sin(t5) - 0.00042011718750000002619432448724979*cos(t1)^2*cos(t3)*sin(t2)*sin(t4)*sin(t5) - 0.00042011718750000002619432448724979*cos(t1)^2*cos(t4)*sin(t2)*sin(t3)*sin(t5) + 0.00042011718750000002619432448724979*cos(t2)*sin(t1)^2*sin(t3)*sin(t4)*sin(t5) + 0.00042011718750000002619432448724979*cos(t3)*sin(t1)^2*sin(t2)*sin(t4)*sin(t5) + 0.00042011718750000002619432448724979*cos(t4)*sin(t1)^2*sin(t2)*sin(t3)*sin(t5)) + td6*(0.5*(0.00084023437500000005238864897449957*cos(t1)*cos(t2)*cos(t3)*sin(t4)*sin(t5) + 0.00084023437500000005238864897449957*cos(t1)*cos(t2)*cos(t4)*sin(t3)*sin(t5) + 0.00084023437500000005238864897449957*cos(t1)*cos(t3)*cos(t4)*sin(t2)*sin(t5) - 0.00084023437500000005238864897449957*cos(t1)*sin(t2)*sin(t3)*sin(t4)*sin(t5))*(cos(t1)*cos(t2)*sin(t3)*sin(t4)*sin(t5) - 1.0*cos(t1)*cos(t2)*cos(t3)*cos(t4)*sin(t5) - 1.0*cos(t5)*sin(t1) + cos(t1)*cos(t3)*sin(t2)*sin(t4)*sin(t5) + cos(t1)*cos(t4)*sin(t2)*sin(t3)*sin(t5)) + 0.5*(cos(t1)*cos(t2)*cos(t3)*sin(t4)*sin(t5) + cos(t1)*cos(t2)*cos(t4)*sin(t3)*sin(t5) + cos(t1)*cos(t3)*cos(t4)*sin(t2)*sin(t5) - 1.0*cos(t1)*sin(t2)*sin(t3)*sin(t4)*sin(t5))*(0.00084023437500000005238864897449957*cos(t1)*cos(t2)*sin(t3)*sin(t4)*sin(t5) - 0.00084023437500000005238864897449957*cos(t1)*cos(t2)*cos(t3)*cos(t4)*sin(t5) - 0.00084023437500000005238864897449957*cos(t5)*sin(t1) + 0.00084023437500000005238864897449957*cos(t1)*cos(t3)*sin(t2)*sin(t4)*sin(t5) + 0.00084023437500000005238864897449957*cos(t1)*cos(t4)*sin(t2)*sin(t3)*sin(t5)) + 0.5*(0.0016804687500000001047772979489991*cos(t2)*cos(t3)*sin(t1)*sin(t4)*sin(t5) + 0.0016804687500000001047772979489991*cos(t2)*cos(t4)*sin(t1)*sin(t3)*sin(t5) + 0.0016804687500000001047772979489991*cos(t3)*cos(t4)*sin(t1)*sin(t2)*sin(t5) - 0.0016804687500000001047772979489991*sin(t1)*sin(t2)*sin(t3)*sin(t4)*sin(t5))*(cos(t1)*cos(t5) - 1.0*cos(t2)*cos(t3)*cos(t4)*sin(t1)*sin(t5) + cos(t2)*sin(t1)*sin(t3)*sin(t4)*sin(t5) + cos(t3)*sin(t1)*sin(t2)*sin(t4)*sin(t5) + cos(t4)*sin(t1)*sin(t2)*sin(t3)*sin(t5)) + 0.5*(cos(t2)*cos(t3)*sin(t1)*sin(t4)*sin(t5) + cos(t2)*cos(t4)*sin(t1)*sin(t3)*sin(t5) + cos(t3)*cos(t4)*sin(t1)*sin(t2)*sin(t5) - 1.0*sin(t1)*sin(t2)*sin(t3)*sin(t4)*sin(t5))*(0.0016804687500000001047772979489991*cos(t1)*cos(t5) - 0.0016804687500000001047772979489991*cos(t2)*cos(t3)*cos(t4)*sin(t1)*sin(t5) + 0.0016804687500000001047772979489991*cos(t2)*sin(t1)*sin(t3)*sin(t4)*sin(t5) + 0.0016804687500000001047772979489991*cos(t3)*sin(t1)*sin(t2)*sin(t4)*sin(t5) + 0.0016804687500000001047772979489991*cos(t4)*sin(t1)*sin(t2)*sin(t3)*sin(t5))) - 1.0*td5*(0.00063017578125000003929148673087468*cos(2.0*t2)*cos(2.0*t3)*cos(2.0*t4)*sin(t5) - 0.00042011718750000002619432448724979*cos(t1)^2*sin(t5) - 0.00042011718750000002619432448724979*sin(t5) - 0.00063017578125000003929148673087468*cos(2.0*t2)*sin(2.0*t3)*sin(2.0*t4)*sin(t5) - 0.00063017578125000003929148673087468*cos(2.0*t3)*sin(2.0*t2)*sin(2.0*t4)*sin(t5) - 0.00063017578125000003929148673087468*cos(2.0*t4)*sin(2.0*t2)*sin(2.0*t3)*sin(t5) - 0.00021005859375000001309716224362489*cos(2.0*t1)*cos(2.0*t2)*cos(2.0*t3)*cos(2.0*t4)*sin(t5) + 0.00021005859375000001309716224362489*cos(2.0*t1)*cos(2.0*t2)*sin(2.0*t3)*sin(2.0*t4)*sin(t5) + 0.00021005859375000001309716224362489*cos(2.0*t1)*cos(2.0*t3)*sin(2.0*t2)*sin(2.0*t4)*sin(t5) + 0.00021005859375000001309716224362489*cos(2.0*t1)*cos(2.0*t4)*sin(2.0*t2)*sin(2.0*t3)*sin(t5) - 0.00021005859375000001309716224362489*sin(2.0*t1)*cos(t2)*cos(t3)*cos(t4)*cos(t5) + 0.00021005859375000001309716224362489*sin(2.0*t1)*cos(t2)*cos(t5)*sin(t3)*sin(t4) + 0.00021005859375000001309716224362489*sin(2.0*t1)*cos(t3)*cos(t5)*sin(t2)*sin(t4) + 0.00021005859375000001309716224362489*sin(2.0*t1)*cos(t4)*cos(t5)*sin(t2)*sin(t3) - 0.00042011718750000002619432448724979*cos(t1)*cos(t2)*cos(t3)*cos(t4)*cos(t5)*sin(t1) + 0.00042011718750000002619432448724979*cos(t1)*cos(t2)*cos(t5)*sin(t1)*sin(t3)*sin(t4) + 0.00042011718750000002619432448724979*cos(t1)*cos(t3)*cos(t5)*sin(t1)*sin(t2)*sin(t4) + 0.00042011718750000002619432448724979*cos(t1)*cos(t4)*cos(t5)*sin(t1)*sin(t2)*sin(t3))) - td2*(1.0*td5*(0.125*m5*sin(2.0*t5)*L3^2 + 0.00073318229166666670434948649415219*sin(3.0*t2 - 1.0*t1 + t3 + t4) - 0.00073318229166666670434948649415219*sin(t2 - 2.0*t1 + 3.0*t3 + t4) - 0.00036659114583333335217474324707609*sin(3.0*t2 - 2.0*t1 + t3 + t4) + 0.00036659114583333335217474324707609*sin(2.0*t1 + 3.0*t2 + t3 + t4) + 0.00057664973958333336527190549070099*sin(t2 - 2.0*t1 + t3 + t4) - 0.00057664973958333336527190549070099*sin(2.0*t1 + t2 + t3 + t4) - 0.00073318229166666670434948649415219*sin(t1 + 3.0*t2 + t3 + t4) + 0.00073318229166666670434948649415219*sin(2.0*t1 + t2 - 1.0*t3 + t4)) + 1.0*td1*(0.00036659114583333335217474324707609*sin(2.0*t1 - 2.0*t2) - 0.00073318229166666670434948649415219*sin(t1 + 2.0*t2) - 0.001153299479166666730543810981402*sin(2.0*t1) - 0.00073318229166666670434948649415219*sin(t1 - 2.0*t2) + 0.00036659114583333335217474324707609*sin(2.0*t1 + 2.0*t2) + 0.0014663645833333334086989729883044*sin(2.0*t1 - 2.0*t3) - 14401.25*m5*sin(t2 + t3 + t4) - 14401.25*m6*sin(t2 + t3 + t4) + 140.5*L4*m5*sin(t2 + t3 + t4) - 60.75*L3*m5*sin(t2 + t3 + t4 - 1.0*t5) - 0.0625*L3^2*m5*sin(t2 + t3 + t4 - 2.0*t5) + 0.0625*L3^2*m5*sin(t2 + t3 + t4 + 2.0*t5) + 9.5*L3*m5*sin(t2 + t3 + t4 + t5) + 0.25*L3*L4*m5*sin(t2 + t3 + t4 + t5) + 0.25*L3*L4*m5*sin(t2 + t3 + t4 - 1.0*t5)) + 1.0*td4*(0.00073318229166666670434948649415219*sin(2.0*t2) - 0.00073318229166666670434948649415219*cos(2.0*t1)*sin(2.0*t2)) - td6*(0.00084023437500000005238864897449957*cos(t1)*cos(t2)*cos(t3)*sin(t1)*sin(t4)*sin(t5) + 0.00084023437500000005238864897449957*cos(t1)*cos(t2)*cos(t4)*sin(t1)*sin(t3)*sin(t5) + 0.00084023437500000005238864897449957*cos(t1)*cos(t3)*cos(t4)*sin(t1)*sin(t2)*sin(t5) - 0.00084023437500000005238864897449957*cos(t1)*sin(t1)*sin(t2)*sin(t3)*sin(t4)*sin(t5)) - td3*(0.0029327291666666668173979459766088*cos(t2)*sin(t2)*cos(t1)^2 + 0.0014663645833333334086989729883044*sin(2.0*t1 - 2.0*t3) - 0.0029327291666666668173979459766088*cos(t2)*sin(t2) - 38540.0*m5*sin(t4) - 38540.0*m6*sin(t4) - 94.0*L3*m5*sin(t4 - 1.0*t5) + 94.0*L3*m5*sin(t4 + t5) + 376.0*L4*m5*sin(t4)) + 1.0*td2*(38540.0*m5*sin(t4) + 38540.0*m6*sin(t4) + 41820.0*m5*cos(t3)*sin(t4) + 41820.0*m5*cos(t4)*sin(t3) + 41820.0*m6*cos(t3)*sin(t4) + 41820.0*m6*cos(t4)*sin(t3) - 376.0*L4*m5*sin(t4) - 408.0*L4*m5*cos(t3)*sin(t4) - 408.0*L4*m5*cos(t4)*sin(t3) - 188.0*L3*m5*cos(t4)*sin(t5) - 204.0*L3*m5*cos(t3)*cos(t4)*sin(t5) + 204.0*L3*m5*sin(t3)*sin(t4)*sin(t5))) - td1*(1.0*td6*(0.00084023437500000005238864897449957*cos(t1)*cos(t5)*sin(t1) + 0.00042011718750000002619432448724979*cos(t1)^2*cos(t2)*cos(t3)*cos(t4)*sin(t5) - 0.00042011718750000002619432448724979*cos(t2)*cos(t3)*cos(t4)*sin(t1)^2*sin(t5) - 0.00042011718750000002619432448724979*cos(t1)^2*cos(t2)*sin(t3)*sin(t4)*sin(t5) - 0.00042011718750000002619432448724979*cos(t1)^2*cos(t3)*sin(t2)*sin(t4)*sin(t5) - 0.00042011718750000002619432448724979*cos(t1)^2*cos(t4)*sin(t2)*sin(t3)*sin(t5) + 0.00042011718750000002619432448724979*cos(t2)*sin(t1)^2*sin(t3)*sin(t4)*sin(t5) + 0.00042011718750000002619432448724979*cos(t3)*sin(t1)^2*sin(t2)*sin(t4)*sin(t5) + 0.00042011718750000002619432448724979*cos(t4)*sin(t1)^2*sin(t2)*sin(t3)*sin(t5)) + 1.0*td4*(0.001153299479166666730543810981402*sin(2.0*t1) - 0.00073318229166666670434948649415219*cos(2.0*t2)*sin(2.0*t1) + 0.0014663645833333334086989729883044*cos(2.0*t1)*sin(2.0*t3) - 0.0014663645833333334086989729883044*cos(2.0*t3)*sin(2.0*t1)) - td1*(19270.0*m5*sin(2.0*t2 + 2.0*t3 + t4) + 19270.0*m6*sin(2.0*t2 + 2.0*t3 + t4) - 20910.0*m5*sin(t3 + t4) - 20910.0*m6*sin(t3 + t4) + 20910.0*m5*sin(2.0*t2 + t3 + t4) + 20910.0*m6*sin(2.0*t2 + t3 + t4) - 19270.0*m5*sin(t4) - 19270.0*m6*sin(t4) + 5253.125*m5*sin(2.0*t2 + 2.0*t3 + 2.0*t4) + 5253.125*m6*sin(2.0*t2 + 2.0*t3 + 2.0*t4) - 102.5*L4*m5*sin(2.0*t2 + 2.0*t3 + 2.0*t4) + 25.625*L3*m5*sin(2.0*t2 + 2.0*t3 + 2.0*t4 - 1.0*t5) + 51.0*L3*m5*sin(t3 + t4 + t5) - 51.0*L3*m5*sin(2.0*t2 + t3 + t4 + t5) - 47.0*L3*m5*sin(t4 - 1.0*t5) - 0.0625*L3^2*m5*sin(2.0*t2 + 2.0*t3 + 2.0*t4) + 0.5*L4^2*m5*sin(2.0*t2 + 2.0*t3 + 2.0*t4) - 188.0*L4*m5*sin(2.0*t2 + 2.0*t3 + t4) + 0.03125*L3^2*m5*sin(2.0*t2 + 2.0*t3 + 2.0*t4 - 2.0*t5) + 0.03125*L3^2*m5*sin(2.0*t2 + 2.0*t3 + 2.0*t4 + 2.0*t5) + 47.0*L3*m5*sin(2.0*t2 + 2.0*t3 + t4 - 1.0*t5) - 25.625*L3*m5*sin(2.0*t2 + 2.0*t3 + 2.0*t4 + t5) + 204.0*L4*m5*sin(t3 + t4) + 47.0*L3*m5*sin(t4 + t5) - 204.0*L4*m5*sin(2.0*t2 + t3 + t4) - 51.0*L3*m5*sin(t3 + t4 - 1.0*t5) + 51.0*L3*m5*sin(2.0*t2 + t3 + t4 - 1.0*t5) - 47.0*L3*m5*sin(2.0*t2 + 2.0*t3 + t4 + t5) + 188.0*L4*m5*sin(t4) - 0.25*L3*L4*m5*sin(2.0*t2 + 2.0*t3 + 2.0*t4 - 1.0*t5) + 0.25*L3*L4*m5*sin(2.0*t2 + 2.0*t3 + 2.0*t4 + t5)) - td3*(- 0.0029327291666666668173979459766088*sin(t3)*cos(t1)^2*cos(t3) + 0.0029327291666666668173979459766088*cos(t1)*cos(t2)^2*sin(t1) + 0.0058654583333333336347958919532175*cos(t1)*cos(t3)^2*sin(t1) - 0.0067056927083333336871845409277171*cos(t1)*sin(t1) + 0.0029327291666666668173979459766088*sin(t3)*cos(t3)*sin(t1)^2) + 1.0*td2*(0.00073318229166666670434948649415219*sin(t1 - 2.0*t2) + 0.00073318229166666670434948649415219*sin(t1 + 2.0*t2) + 0.001153299479166666730543810981402*sin(2.0*t1) - 0.00036659114583333335217474324707609*sin(2.0*t1 - 2.0*t2) - 0.00036659114583333335217474324707609*sin(2.0*t1 + 2.0*t2) - 0.0014663645833333334086989729883044*sin(2.0*t1 - 2.0*t3)) + td5*(0.00073318229166666670434948649415219*sin(t2 - 2.0*t1 + 3.0*t3 + t4) + 0.00018329557291666667608737162353805*sin(3.0*t2 - 2.0*t1 + t3 + t4) + 0.00018329557291666667608737162353805*sin(2.0*t1 + 3.0*t2 + t3 + t4) + 0.00073318229166666670434948649415219*sin(t2 + t3 + t4) - 0.00057664973958333336527190549070099*sin(t2 - 2.0*t1 + t3 + t4) - 0.00057664973958333336527190549070099*sin(2.0*t1 + t2 + t3 + t4) - 0.00018329557291666667608737162353805*sin(2.0*t1 + t2 - 1.0*t3 - 1.0*t4) - 0.00036659114583333335217474324707609*sin(t3 - 1.0*t2 + t4) + 0.00073318229166666670434948649415219*sin(2.0*t1 + t2 - 1.0*t3 + t4) + 0.00018329557291666667608737162353805*sin(2.0*t1 - 1.0*t2 + t3 + t4) - 0.00036659114583333335217474324707609*sin(3.0*t2 + t3 + t4) - 25.625*L3*m5*sin(t2 + t3 + t4 - 1.0*t5) + 0.125*L3^2*m5*sin(t2 + t3 + t4) - 0.0625*L3^2*m5*sin(t2 + t3 + t4 - 2.0*t5) - 0.0625*L3^2*m5*sin(t2 + t3 + t4 + 2.0*t5) + 25.625*L3*m5*sin(t2 + t3 + t4 + t5) - 0.25*L3*L4*m5*sin(t2 + t3 + t4 + t5) + 0.25*L3*L4*m5*sin(t2 + t3 + t4 - 1.0*t5))) - td3*(1.0*td1*(140.5*L4*m5*sin(t2 + t3 + t4) - 14401.25*m5*sin(t2 + t3 + t4) - 14401.25*m6*sin(t2 + t3 + t4) - 0.0067056927083333336871845409277171*cos(t1)*sin(t1) + 0.0029327291666666668173979459766088*cos(t1)*cos(t2)^2*sin(t1) + 0.0058654583333333336347958919532175*cos(t1)*cos(t3)^2*sin(t1) - 0.0029327291666666668173979459766088*cos(t1)^2*cos(t3)*sin(t3) - 60.75*L3*m5*sin(t2 + t3 + t4 - 1.0*t5) + 0.0029327291666666668173979459766088*cos(t3)*sin(t1)^2*sin(t3) - 0.0625*L3^2*m5*sin(t2 + t3 + t4 - 2.0*t5) + 0.0625*L3^2*m5*sin(t2 + t3 + t4 + 2.0*t5) + 9.5*L3*m5*sin(t2 + t3 + t4 + t5) + 0.25*L3*L4*m5*sin(t2 + t3 + t4 + t5) + 0.25*L3*L4*m5*sin(t2 + t3 + t4 - 1.0*t5)) + 1.0*td2*(0.0029327291666666668173979459766088*cos(t2)*sin(t2)*cos(t1)^2 + 0.0014663645833333334086989729883044*sin(2.0*t1 - 2.0*t3) - 0.0029327291666666668173979459766088*cos(t2)*sin(t2) + 41820.0*m5*sin(t3 + t4) + 41820.0*m6*sin(t3 + t4) + 38540.0*m5*sin(t4) + 38540.0*m6*sin(t4) - 102.0*L3*m5*sin(t3 + t4 + t5) + 94.0*L3*m5*sin(t4 - 1.0*t5) - 408.0*L4*m5*sin(t3 + t4) - 94.0*L3*m5*sin(t4 + t5) + 102.0*L3*m5*sin(t3 + t4 - 1.0*t5) - 376.0*L4*m5*sin(t4)) + 1.0*td5*(0.00036659114583333335217474324707609*sin(3.0*t2 - 1.0*t1 + t3 + t4) - 0.0014663645833333334086989729883044*sin(t2 - 2.0*t1 + 3.0*t3 + t4) - 0.00018329557291666667608737162353805*sin(3.0*t2 - 2.0*t1 + t3 + t4) + 0.00018329557291666667608737162353805*sin(2.0*t1 + 3.0*t2 + t3 + t4) + 0.00036659114583333335217474324707609*sin(t1 - 1.0*t2 + t3 + t4) + 0.00057664973958333336527190549070099*sin(t2 - 2.0*t1 + t3 + t4) - 0.00057664973958333336527190549070099*sin(2.0*t1 + t2 + t3 + t4) - 0.00036659114583333335217474324707609*sin(t1 + 3.0*t2 + t3 + t4) + 0.00018329557291666667608737162353805*sin(2.0*t1 + t2 - 1.0*t3 - 1.0*t4) + 0.00036659114583333335217474324707609*sin(t1 + t2 - 1.0*t3 - 1.0*t4) + 0.00018329557291666667608737162353805*sin(2.0*t1 - 1.0*t2 + t3 + t4) - 47.0*L3*m5*sin(t4 - 1.0*t5) - 47.0*L3*m5*sin(t4 + t5) + 0.25*L3^2*m5*cos(t5)*sin(t5) + 94.0*L3*m5*cos(t5)*sin(t4)) - td6*(0.00084023437500000005238864897449957*cos(t1)*cos(t2)*cos(t3)*sin(t1)*sin(t4)*sin(t5) + 0.00084023437500000005238864897449957*cos(t1)*cos(t2)*cos(t4)*sin(t1)*sin(t3)*sin(t5) + 0.00084023437500000005238864897449957*cos(t1)*cos(t3)*cos(t4)*sin(t1)*sin(t2)*sin(t5) - 0.00084023437500000005238864897449957*cos(t1)*sin(t1)*sin(t2)*sin(t3)*sin(t4)*sin(t5)) - td4*(0.0014663645833333334086989729883044*cos(2.0*t1)*sin(2.0*t3) - 0.0014663645833333334086989729883044*cos(2.0*t3)*sin(2.0*t1)) + 1.0*td3*(38540.0*m5*sin(t4) + 38540.0*m6*sin(t4) - 376.0*L4*m5*sin(t4) - 188.0*L3*m5*cos(t4)*sin(t5)))
     td4*(td5*(0.00036659114583333335217474324707609*sin(2.0*t3 - 1.0*t1 + 2.0*t4) + 0.00036659114583333335217474324707609*sin(2.0*t1 + 2.0*t2 + 2.0*t4) + 0.000091647786458333338043685811769024*sin(2.0*t3 - 2.0*t1 + 2.0*t4) + 0.000091647786458333338043685811769024*sin(2.0*t1 + 2.0*t3 + 2.0*t4) + 0.001729949218750000095815716472103*sin(2.0*t2 + 2.0*t3 + 2.0*t4) + 0.00054988671875000002826211487061414*sin(4.0*t2 + 2.0*t3 + 2.0*t4) - 0.00036659114583333335217474324707609*sin(4.0*t2 - 1.0*t1 + 2.0*t3 + 2.0*t4) - 0.00028832486979166668263595274535049*sin(2.0*t2 - 2.0*t1 + 2.0*t3 + 2.0*t4) - 0.00028832486979166668263595274535049*sin(2.0*t1 + 2.0*t2 + 2.0*t3 + 2.0*t4) + 0.00036659114583333335217474324707609*sin(2.0*t2 - 2.0*t1 + 4.0*t3 + 2.0*t4) + 0.000091647786458333338043685811769024*sin(4.0*t2 - 2.0*t1 + 2.0*t3 + 2.0*t4) + 0.000091647786458333338043685811769024*sin(2.0*t1 + 4.0*t2 + 2.0*t3 + 2.0*t4) + 0.00036659114583333335217474324707609*sin(t1 + 2.0*t3 + 2.0*t4) - 0.00036659114583333335217474324707609*sin(t1 + 4.0*t2 + 2.0*t3 + 2.0*t4) + 0.00054988671875000002826211487061414*sin(2.0*t3 + 2.0*t4)) - 1.0*td1*(0.00036659114583333335217474324707609*sin(3.0*t2 - 1.0*t1 + t3 + t4) - 0.00073318229166666670434948649415219*sin(t2 - 2.0*t1 + 3.0*t3 + t4) - 0.00018329557291666667608737162353805*sin(3.0*t2 - 2.0*t1 + t3 + t4) - 0.00018329557291666667608737162353805*sin(2.0*t1 + 3.0*t2 + t3 + t4) + 0.00073318229166666670434948649415219*sin(t2 + t3 + t4) - 0.00036659114583333335217474324707609*sin(t1 - 1.0*t2 + t3 + t4) + 0.00057664973958333336527190549070099*sin(t2 - 2.0*t1 + t3 + t4) + 0.00057664973958333336527190549070099*sin(2.0*t1 + t2 + t3 + t4) + 0.00036659114583333335217474324707609*sin(t1 + 3.0*t2 + t3 + t4) + 0.00018329557291666667608737162353805*sin(2.0*t1 + t2 - 1.0*t3 - 1.0*t4) - 0.00036659114583333335217474324707609*sin(t3 - 1.0*t2 + t4) + 0.00036659114583333335217474324707609*sin(t1 + t2 - 1.0*t3 - 1.0*t4) - 0.00073318229166666670434948649415219*sin(2.0*t1 + t2 - 1.0*t3 + t4) - 0.00018329557291666667608737162353805*sin(2.0*t1 - 1.0*t2 + t3 + t4) - 0.00036659114583333335217474324707609*sin(3.0*t2 + t3 + t4) + 35.125*L3*m5*sin(t2 + t3 + t4 - 1.0*t5) + 0.125*L3^2*m5*sin(t2 + t3 + t4) + 0.0625*L3^2*m5*sin(t2 + t3 + t4 - 2.0*t5) + 0.0625*L3^2*m5*sin(t2 + t3 + t4 + 2.0*t5) + 35.125*L3*m5*sin(t2 + t3 + t4 + t5)) + td3*(47.0*L3*m5*sin(t4 - 1.0*t5) - 0.00073318229166666670434948649415219*sin(2.0*t1 + t2 - 1.0*t3 + t4) - 0.00073318229166666670434948649415219*sin(t2 - 2.0*t1 + 3.0*t3 + t4) + 47.0*L3*m5*sin(t4 + t5) + 0.25*L3^2*m5*cos(t5)*sin(t5) + 94.0*L3*m5*cos(t5)*sin(t4)) + td2*(0.00036659114583333335217474324707609*sin(3.0*t2 - 1.0*t1 + t3 + t4) - 0.00018329557291666667608737162353805*sin(3.0*t2 - 2.0*t1 + t3 + t4) + 0.00018329557291666667608737162353805*sin(2.0*t1 + 3.0*t2 + t3 + t4) - 0.00036659114583333335217474324707609*sin(t1 - 1.0*t2 + t3 + t4) - 0.00036659114583333335217474324707609*sin(t1 + 3.0*t2 + t3 + t4) - 0.00018329557291666667608737162353805*sin(2.0*t1 + t2 - 1.0*t3 - 1.0*t4) - 0.00036659114583333335217474324707609*sin(t1 + t2 - 1.0*t3 - 1.0*t4) - 0.00018329557291666667608737162353805*sin(2.0*t1 - 1.0*t2 + t3 + t4) + 102.0*L3*m5*sin(t3 + t4 + t5) + 94.0*L3*m5*sin(t4 - 1.0*t5) + 94.0*L3*m5*sin(t4 + t5) + 102.0*L3*m5*sin(t3 + t4 - 1.0*t5) + 0.125*L3^2*m5*sin(2.0*t5)) - 1.0*td6*(0.00042011718750000002619432448724979*sin(t5) + 0.00042011718750000002619432448724979*cos(t1)^2*sin(t5) + 0.00063017578125000003929148673087468*cos(2.0*t2)*cos(2.0*t3)*cos(2.0*t4)*sin(t5) - 0.00063017578125000003929148673087468*cos(2.0*t2)*sin(2.0*t3)*sin(2.0*t4)*sin(t5) - 0.00063017578125000003929148673087468*cos(2.0*t3)*sin(2.0*t2)*sin(2.0*t4)*sin(t5) - 0.00063017578125000003929148673087468*cos(2.0*t4)*sin(2.0*t2)*sin(2.0*t3)*sin(t5) - 0.00021005859375000001309716224362489*cos(2.0*t1)*cos(2.0*t2)*cos(2.0*t3)*cos(2.0*t4)*sin(t5) + 0.00021005859375000001309716224362489*cos(2.0*t1)*cos(2.0*t2)*sin(2.0*t3)*sin(2.0*t4)*sin(t5) + 0.00021005859375000001309716224362489*cos(2.0*t1)*cos(2.0*t3)*sin(2.0*t2)*sin(2.0*t4)*sin(t5) + 0.00021005859375000001309716224362489*cos(2.0*t1)*cos(2.0*t4)*sin(2.0*t2)*sin(2.0*t3)*sin(t5) - 0.00021005859375000001309716224362489*sin(2.0*t1)*cos(t2)*cos(t3)*cos(t4)*cos(t5) + 0.00021005859375000001309716224362489*sin(2.0*t1)*cos(t2)*cos(t5)*sin(t3)*sin(t4) + 0.00021005859375000001309716224362489*sin(2.0*t1)*cos(t3)*cos(t5)*sin(t2)*sin(t4) + 0.00021005859375000001309716224362489*sin(2.0*t1)*cos(t4)*cos(t5)*sin(t2)*sin(t3) + 0.00042011718750000002619432448724979*cos(t1)*cos(t2)*cos(t3)*cos(t4)*cos(t5)*sin(t1) - 0.00042011718750000002619432448724979*cos(t1)*cos(t2)*cos(t5)*sin(t1)*sin(t3)*sin(t4) - 0.00042011718750000002619432448724979*cos(t1)*cos(t3)*cos(t5)*sin(t1)*sin(t2)*sin(t4) - 0.00042011718750000002619432448724979*cos(t1)*cos(t4)*cos(t5)*sin(t1)*sin(t2)*sin(t3)) + 0.125*L3^2*m5*td4*sin(2.0*t5)) - td1*(1.0*td5*(0.00018329557291666667608737162353805*sin(2.0*t3 - 1.0*t1 + 2.0*t4) - 0.00036659114583333335217474324707609*sin(2.0*t1 + 2.0*t2 + 2.0*t4) + 0.000091647786458333338043685811769024*sin(2.0*t3 - 2.0*t1 + 2.0*t4) - 0.000091647786458333338043685811769024*sin(2.0*t1 + 2.0*t3 + 2.0*t4) - 0.00018329557291666667608737162353805*sin(4.0*t2 - 1.0*t1 + 2.0*t3 + 2.0*t4) - 0.00028832486979166668263595274535049*sin(2.0*t2 - 2.0*t1 + 2.0*t3 + 2.0*t4) + 0.00028832486979166668263595274535049*sin(2.0*t1 + 2.0*t2 + 2.0*t3 + 2.0*t4) + 0.00036659114583333335217474324707609*sin(2.0*t2 - 2.0*t1 + 4.0*t3 + 2.0*t4) + 0.000091647786458333338043685811769024*sin(4.0*t2 - 2.0*t1 + 2.0*t3 + 2.0*t4) - 0.000091647786458333338043685811769024*sin(2.0*t1 + 4.0*t2 + 2.0*t3 + 2.0*t4) - 0.00018329557291666667608737162353805*sin(t1 + 2.0*t3 + 2.0*t4) + 0.00018329557291666667608737162353805*sin(t1 + 4.0*t2 + 2.0*t3 + 2.0*t4) - 0.00057664973958333336527190549070099*sin(2.0*t1) + 0.00018329557291666667608737162353805*sin(2.0*t1 - 2.0*t2) + 0.00018329557291666667608737162353805*sin(2.0*t1 + 2.0*t2) + 0.00073318229166666670434948649415219*sin(2.0*t1 - 2.0*t3)) + 1.0*td3*(0.00073318229166666670434948649415219*sin(t2 - 2.0*t1 + 3.0*t3 + t4) - 0.00036659114583333335217474324707609*sin(3.0*t2 - 1.0*t1 + t3 + t4) + 0.00018329557291666667608737162353805*sin(3.0*t2 - 2.0*t1 + t3 + t4) + 0.00018329557291666667608737162353805*sin(2.0*t1 + 3.0*t2 + t3 + t4) - 0.00073318229166666670434948649415219*sin(t2 + t3 + t4) + 0.00036659114583333335217474324707609*sin(t1 - 1.0*t2 + t3 + t4) - 0.00057664973958333336527190549070099*sin(t2 - 2.0*t1 + t3 + t4) - 0.00057664973958333336527190549070099*sin(2.0*t1 + t2 + t3 + t4) - 0.00036659114583333335217474324707609*sin(t1 + 3.0*t2 + t3 + t4) - 0.00018329557291666667608737162353805*sin(2.0*t1 + t2 - 1.0*t3 - 1.0*t4) + 0.00036659114583333335217474324707609*sin(t3 - 1.0*t2 + t4) - 0.00036659114583333335217474324707609*sin(t1 + t2 - 1.0*t3 - 1.0*t4) + 0.00073318229166666670434948649415219*sin(2.0*t1 + t2 - 1.0*t3 + t4) + 0.00018329557291666667608737162353805*sin(2.0*t1 - 1.0*t2 + t3 + t4) + 0.00036659114583333335217474324707609*sin(3.0*t2 + t3 + t4) - 94.0*L3*m5*sin(t2 + t3 + t5) + 25.625*L3*m5*sin(t2 + t3 + t4 - 1.0*t5) - 0.125*L3^2*m5*sin(t2 + t3 + t4) + 0.0625*L3^2*m5*sin(t2 + t3 + t4 - 2.0*t5) + 0.0625*L3^2*m5*sin(t2 + t3 + t4 + 2.0*t5) - 25.625*L3*m5*sin(t2 + t3 + t4 + t5) + 94.0*L3*m5*sin(t2 + t3 - 1.0*t5) + 0.25*L3*L4*m5*sin(t2 + t3 + t4 + t5) - 0.25*L3*L4*m5*sin(t2 + t3 + t4 - 1.0*t5)) + 1.0*td1*(12.8125*L3*m5*sin(2.0*t2 + 2.0*t3 + 2.0*t4 - 1.0*t5) - 51.0*L3*m5*sin(t3 + t4 + t5) + 51.0*L3*m5*sin(2.0*t2 + t3 + t4 + t5) - 47.0*L3*m5*sin(t4 - 1.0*t5) + 0.03125*L3^2*m5*sin(2.0*t2 + 2.0*t3 + 2.0*t4 - 2.0*t5) - 0.03125*L3^2*m5*sin(2.0*t2 + 2.0*t3 + 2.0*t4 + 2.0*t5) + 47.0*L3*m5*sin(2.0*t2 + 2.0*t3 + t4 - 1.0*t5) + 12.8125*L3*m5*sin(2.0*t2 + 2.0*t3 + 2.0*t4 + t5) - 47.0*L3*m5*sin(t4 + t5) - 51.0*L3*m5*sin(t3 + t4 - 1.0*t5) + 51.0*L3*m5*sin(2.0*t2 + t3 + t4 - 1.0*t5) + 47.0*L3*m5*sin(2.0*t2 + 2.0*t3 + t4 + t5) + 0.0625*L3^2*m5*sin(2.0*t5) + 70.25*L3*m5*sin(t5) - 0.125*L3*L4*m5*sin(2.0*t2 + 2.0*t3 + 2.0*t4 - 1.0*t5) - 0.125*L3*L4*m5*sin(2.0*t2 + 2.0*t3 + 2.0*t4 + t5)) + 1.0*td4*(0.00073318229166666670434948649415219*sin(t2 - 2.0*t1 + 3.0*t3 + t4) - 0.00036659114583333335217474324707609*sin(3.0*t2 - 1.0*t1 + t3 + t4) + 0.00018329557291666667608737162353805*sin(3.0*t2 - 2.0*t1 + t3 + t4) + 0.00018329557291666667608737162353805*sin(2.0*t1 + 3.0*t2 + t3 + t4) - 0.00073318229166666670434948649415219*sin(t2 + t3 + t4) + 0.00036659114583333335217474324707609*sin(t1 - 1.0*t2 + t3 + t4) - 0.00057664973958333336527190549070099*sin(t2 - 2.0*t1 + t3 + t4) - 0.00057664973958333336527190549070099*sin(2.0*t1 + t2 + t3 + t4) - 0.00036659114583333335217474324707609*sin(t1 + 3.0*t2 + t3 + t4) - 0.00018329557291666667608737162353805*sin(2.0*t1 + t2 - 1.0*t3 - 1.0*t4) + 0.00036659114583333335217474324707609*sin(t3 - 1.0*t2 + t4) - 0.00036659114583333335217474324707609*sin(t1 + t2 - 1.0*t3 - 1.0*t4) + 0.00073318229166666670434948649415219*sin(2.0*t1 + t2 - 1.0*t3 + t4) + 0.00018329557291666667608737162353805*sin(2.0*t1 - 1.0*t2 + t3 + t4) + 0.00036659114583333335217474324707609*sin(3.0*t2 + t3 + t4) + 25.625*L3*m5*sin(t2 + t3 + t4 - 1.0*t5) - 0.125*L3^2*m5*sin(t2 + t3 + t4) + 0.0625*L3^2*m5*sin(t2 + t3 + t4 - 2.0*t5) + 0.0625*L3^2*m5*sin(t2 + t3 + t4 + 2.0*t5) - 25.625*L3*m5*sin(t2 + t3 + t4 + t5) + 0.25*L3*L4*m5*sin(t2 + t3 + t4 + t5) - 0.25*L3*L4*m5*sin(t2 + t3 + t4 - 1.0*t5)) - td2*(0.00073318229166666670434948649415219*sin(3.0*t2 - 1.0*t1 + t3 + t4) - 0.00073318229166666670434948649415219*sin(t2 - 2.0*t1 + 3.0*t3 + t4) - 0.00018329557291666667608737162353805*sin(3.0*t2 - 2.0*t1 + t3 + t4) - 0.00018329557291666667608737162353805*sin(2.0*t1 + 3.0*t2 + t3 + t4) + 0.00073318229166666670434948649415219*sin(t2 + t3 + t4) + 0.00057664973958333336527190549070099*sin(t2 - 2.0*t1 + t3 + t4) + 0.00057664973958333336527190549070099*sin(2.0*t1 + t2 + t3 + t4) + 0.00073318229166666670434948649415219*sin(t1 + 3.0*t2 + t3 + t4) + 0.00018329557291666667608737162353805*sin(2.0*t1 + t2 - 1.0*t3 - 1.0*t4) + 0.00036659114583333335217474324707609*sin(t3 - 1.0*t2 + t4) - 0.00073318229166666670434948649415219*sin(2.0*t1 + t2 - 1.0*t3 + t4) - 0.00018329557291666667608737162353805*sin(2.0*t1 - 1.0*t2 + t3 + t4) - 0.0010997734375000000565242297412283*sin(3.0*t2 + t3 + t4) + 94.0*L3*m5*sin(t2 + t3 + t5) - 25.625*L3*m5*sin(t2 + t3 + t4 - 1.0*t5) - 102.0*L3*m5*sin(t2 - 1.0*t5) + 0.125*L3^2*m5*sin(t2 + t3 + t4) - 0.0625*L3^2*m5*sin(t2 + t3 + t4 - 2.0*t5) - 0.0625*L3^2*m5*sin(t2 + t3 + t4 + 2.0*t5) + 25.625*L3*m5*sin(t2 + t3 + t4 + t5) + 102.0*L3*m5*sin(t2 + t5) - 94.0*L3*m5*sin(t2 + t3 - 1.0*t5) - 0.25*L3*L4*m5*sin(t2 + t3 + t4 + t5) + 0.25*L3*L4*m5*sin(t2 + t3 + t4 - 1.0*t5)) + td6*(0.00021005859375000001309716224362489*cos(2.0*t2)*cos(2.0*t3)*sin(2.0*t1)*sin(2.0*t4)*sin(t5) + 0.00021005859375000001309716224362489*cos(2.0*t2)*cos(2.0*t4)*sin(2.0*t1)*sin(2.0*t3)*sin(t5) + 0.00021005859375000001309716224362489*cos(2.0*t3)*cos(2.0*t4)*sin(2.0*t1)*sin(2.0*t2)*sin(t5) - 0.00042011718750000002619432448724979*cos(2.0*t1)*cos(t2)*cos(t3)*cos(t5)*sin(t4) - 0.00042011718750000002619432448724979*cos(2.0*t1)*cos(t2)*cos(t4)*cos(t5)*sin(t3) - 0.00042011718750000002619432448724979*cos(2.0*t1)*cos(t3)*cos(t4)*cos(t5)*sin(t2) - 0.00021005859375000001309716224362489*sin(2.0*t1)*sin(2.0*t2)*sin(2.0*t3)*sin(2.0*t4)*sin(t5) + 0.00042011718750000002619432448724979*cos(2.0*t1)*cos(t5)*sin(t2)*sin(t3)*sin(t4))) - td5*(1.0*td4*(0.00036659114583333335217474324707609*sin(2.0*t3 - 1.0*t1 + 2.0*t4) + 0.00036659114583333335217474324707609*sin(2.0*t1 + 2.0*t2 + 2.0*t4) + 0.000091647786458333338043685811769024*sin(2.0*t3 - 2.0*t1 + 2.0*t4) + 0.000091647786458333338043685811769024*sin(2.0*t1 + 2.0*t3 + 2.0*t4) + 0.001729949218750000095815716472103*sin(2.0*t2 + 2.0*t3 + 2.0*t4) + 0.00054988671875000002826211487061414*sin(4.0*t2 + 2.0*t3 + 2.0*t4) - 0.00036659114583333335217474324707609*sin(4.0*t2 - 1.0*t1 + 2.0*t3 + 2.0*t4) - 0.00028832486979166668263595274535049*sin(2.0*t2 - 2.0*t1 + 2.0*t3 + 2.0*t4) - 0.00028832486979166668263595274535049*sin(2.0*t1 + 2.0*t2 + 2.0*t3 + 2.0*t4) + 0.00036659114583333335217474324707609*sin(2.0*t2 - 2.0*t1 + 4.0*t3 + 2.0*t4) + 0.000091647786458333338043685811769024*sin(4.0*t2 - 2.0*t1 + 2.0*t3 + 2.0*t4) + 0.000091647786458333338043685811769024*sin(2.0*t1 + 4.0*t2 + 2.0*t3 + 2.0*t4) + 0.00036659114583333335217474324707609*sin(t1 + 2.0*t3 + 2.0*t4) - 0.00036659114583333335217474324707609*sin(t1 + 4.0*t2 + 2.0*t3 + 2.0*t4) + 0.00054988671875000002826211487061414*sin(2.0*t3 + 2.0*t4) - 51.25*L3*m5*sin(t5) + 0.5*L3*L4*m5*sin(t5)) + 1.0*td6*(0.00063017578125000003929148673087468*cos(2.0*t2)*cos(2.0*t3)*sin(2.0*t4)*cos(t5) + 0.00063017578125000003929148673087468*cos(2.0*t2)*cos(2.0*t4)*sin(2.0*t3)*cos(t5) + 0.00063017578125000003929148673087468*cos(2.0*t3)*cos(2.0*t4)*sin(2.0*t2)*cos(t5) - 0.00063017578125000003929148673087468*sin(2.0*t2)*sin(2.0*t3)*sin(2.0*t4)*cos(t5) - 0.00021005859375000001309716224362489*cos(2.0*t1)*cos(2.0*t2)*cos(2.0*t3)*sin(2.0*t4)*cos(t5) - 0.00021005859375000001309716224362489*cos(2.0*t1)*cos(2.0*t2)*cos(2.0*t4)*sin(2.0*t3)*cos(t5) - 0.00021005859375000001309716224362489*cos(2.0*t1)*cos(2.0*t3)*cos(2.0*t4)*sin(2.0*t2)*cos(t5) + 0.00021005859375000001309716224362489*cos(2.0*t1)*sin(2.0*t2)*sin(2.0*t3)*sin(2.0*t4)*cos(t5) + 0.00042011718750000002619432448724979*sin(2.0*t1)*cos(t2)*cos(t3)*sin(t4)*sin(t5) + 0.00042011718750000002619432448724979*sin(2.0*t1)*cos(t2)*cos(t4)*sin(t3)*sin(t5) + 0.00042011718750000002619432448724979*sin(2.0*t1)*cos(t3)*cos(t4)*sin(t2)*sin(t5) - 0.00042011718750000002619432448724979*sin(2.0*t1)*sin(t2)*sin(t3)*sin(t4)*sin(t5)) - 1.0*td1*(0.00018329557291666667608737162353805*sin(2.0*t3 - 1.0*t1 + 2.0*t4) - 0.00036659114583333335217474324707609*sin(2.0*t1 + 2.0*t2 + 2.0*t4) + 0.000091647786458333338043685811769024*sin(2.0*t3 - 2.0*t1 + 2.0*t4) - 0.000091647786458333338043685811769024*sin(2.0*t1 + 2.0*t3 + 2.0*t4) - 0.00018329557291666667608737162353805*sin(4.0*t2 - 1.0*t1 + 2.0*t3 + 2.0*t4) - 0.00028832486979166668263595274535049*sin(2.0*t2 - 2.0*t1 + 2.0*t3 + 2.0*t4) + 0.00028832486979166668263595274535049*sin(2.0*t1 + 2.0*t2 + 2.0*t3 + 2.0*t4) + 0.00036659114583333335217474324707609*sin(2.0*t2 - 2.0*t1 + 4.0*t3 + 2.0*t4) + 0.000091647786458333338043685811769024*sin(4.0*t2 - 2.0*t1 + 2.0*t3 + 2.0*t4) - 0.000091647786458333338043685811769024*sin(2.0*t1 + 4.0*t2 + 2.0*t3 + 2.0*t4) - 0.00018329557291666667608737162353805*sin(t1 + 2.0*t3 + 2.0*t4) + 0.00018329557291666667608737162353805*sin(t1 + 4.0*t2 + 2.0*t3 + 2.0*t4) - 0.00057664973958333336527190549070099*sin(2.0*t1) + 0.00018329557291666667608737162353805*sin(2.0*t1 - 2.0*t2) + 0.00018329557291666667608737162353805*sin(2.0*t1 + 2.0*t2) + 0.00073318229166666670434948649415219*sin(2.0*t1 - 2.0*t3) - 94.0*L3*m5*sin(t2 + t3 + t5) + 9.5*L3*m5*sin(t2 + t3 + t4 - 1.0*t5) - 102.0*L3*m5*sin(t2 - 1.0*t5) - 60.75*L3*m5*sin(t2 + t3 + t4 + t5) - 102.0*L3*m5*sin(t2 + t5) - 94.0*L3*m5*sin(t2 + t3 - 1.0*t5) + 0.25*L3*L4*m5*sin(t2 + t3 + t4 + t5) + 0.25*L3*L4*m5*sin(t2 + t3 + t4 - 1.0*t5)) + 1.0*td2*(0.00036659114583333335217474324707609*sin(2.0*t1 + 2.0*t2 + 2.0*t4) + 0.001729949218750000095815716472103*sin(2.0*t2 + 2.0*t3 + 2.0*t4) + 0.0010997734375000000565242297412283*sin(4.0*t2 + 2.0*t3 + 2.0*t4) - 0.00073318229166666670434948649415219*sin(4.0*t2 - 1.0*t1 + 2.0*t3 + 2.0*t4) - 0.00028832486979166668263595274535049*sin(2.0*t2 - 2.0*t1 + 2.0*t3 + 2.0*t4) - 0.00028832486979166668263595274535049*sin(2.0*t1 + 2.0*t2 + 2.0*t3 + 2.0*t4) + 0.00036659114583333335217474324707609*sin(2.0*t2 - 2.0*t1 + 4.0*t3 + 2.0*t4) + 0.00018329557291666667608737162353805*sin(4.0*t2 - 2.0*t1 + 2.0*t3 + 2.0*t4) + 0.00018329557291666667608737162353805*sin(2.0*t1 + 4.0*t2 + 2.0*t3 + 2.0*t4) - 0.00073318229166666670434948649415219*sin(t1 + 4.0*t2 + 2.0*t3 + 2.0*t4) + 0.00036659114583333335217474324707609*sin(2.0*t2) + 0.00018329557291666667608737162353805*sin(2.0*t1 - 2.0*t2) - 0.00018329557291666667608737162353805*sin(2.0*t1 + 2.0*t2) - 102.0*L3*m5*sin(t3 + t4 + t5) + 94.0*L3*m5*sin(t4 - 1.0*t5) - 94.0*L3*m5*sin(t4 + t5) + 102.0*L3*m5*sin(t3 + t4 - 1.0*t5) - 51.25*L3*m5*sin(t5) + 0.5*L3*L4*m5*sin(t5)) + 1.0*td3*(0.00036659114583333335217474324707609*sin(2.0*t3 - 1.0*t1 + 2.0*t4) + 0.000091647786458333338043685811769024*sin(2.0*t3 - 2.0*t1 + 2.0*t4) + 0.000091647786458333338043685811769024*sin(2.0*t1 + 2.0*t3 + 2.0*t4) + 0.001729949218750000095815716472103*sin(2.0*t2 + 2.0*t3 + 2.0*t4) + 0.00054988671875000002826211487061414*sin(4.0*t2 + 2.0*t3 + 2.0*t4) - 0.00036659114583333335217474324707609*sin(4.0*t2 - 1.0*t1 + 2.0*t3 + 2.0*t4) - 0.00028832486979166668263595274535049*sin(2.0*t2 - 2.0*t1 + 2.0*t3 + 2.0*t4) - 0.00028832486979166668263595274535049*sin(2.0*t1 + 2.0*t2 + 2.0*t3 + 2.0*t4) + 0.00073318229166666670434948649415219*sin(2.0*t2 - 2.0*t1 + 4.0*t3 + 2.0*t4) + 0.000091647786458333338043685811769024*sin(4.0*t2 - 2.0*t1 + 2.0*t3 + 2.0*t4) + 0.000091647786458333338043685811769024*sin(2.0*t1 + 4.0*t2 + 2.0*t3 + 2.0*t4) + 0.00036659114583333335217474324707609*sin(t1 + 2.0*t3 + 2.0*t4) - 0.00036659114583333335217474324707609*sin(t1 + 4.0*t2 + 2.0*t3 + 2.0*t4) + 0.00073318229166666670434948649415219*sin(2.0*t1 - 2.0*t3) + 0.00054988671875000002826211487061414*sin(2.0*t3 + 2.0*t4) + 94.0*L3*m5*sin(t4 - 1.0*t5) - 94.0*L3*m5*sin(t4 + t5) - 51.25*L3*m5*sin(t5) + 0.5*L3*L4*m5*sin(t5))) + td3*(td5*(0.00036659114583333335217474324707609*sin(2.0*t3 - 1.0*t1 + 2.0*t4) + 0.000091647786458333338043685811769024*sin(2.0*t3 - 2.0*t1 + 2.0*t4) + 0.000091647786458333338043685811769024*sin(2.0*t1 + 2.0*t3 + 2.0*t4) + 0.001729949218750000095815716472103*sin(2.0*t2 + 2.0*t3 + 2.0*t4) + 0.00054988671875000002826211487061414*sin(4.0*t2 + 2.0*t3 + 2.0*t4) - 0.00036659114583333335217474324707609*sin(4.0*t2 - 1.0*t1 + 2.0*t3 + 2.0*t4) - 0.00028832486979166668263595274535049*sin(2.0*t2 - 2.0*t1 + 2.0*t3 + 2.0*t4) - 0.00028832486979166668263595274535049*sin(2.0*t1 + 2.0*t2 + 2.0*t3 + 2.0*t4) + 0.00073318229166666670434948649415219*sin(2.0*t2 - 2.0*t1 + 4.0*t3 + 2.0*t4) + 0.000091647786458333338043685811769024*sin(4.0*t2 - 2.0*t1 + 2.0*t3 + 2.0*t4) + 0.000091647786458333338043685811769024*sin(2.0*t1 + 4.0*t2 + 2.0*t3 + 2.0*t4) + 0.00036659114583333335217474324707609*sin(t1 + 2.0*t3 + 2.0*t4) - 0.00036659114583333335217474324707609*sin(t1 + 4.0*t2 + 2.0*t3 + 2.0*t4) + 0.00073318229166666670434948649415219*sin(2.0*t1 - 2.0*t3) + 0.00054988671875000002826211487061414*sin(2.0*t3 + 2.0*t4)) - 1.0*td1*(0.00036659114583333335217474324707609*sin(3.0*t2 - 1.0*t1 + t3 + t4) - 0.00073318229166666670434948649415219*sin(t2 - 2.0*t1 + 3.0*t3 + t4) - 0.00018329557291666667608737162353805*sin(3.0*t2 - 2.0*t1 + t3 + t4) - 0.00018329557291666667608737162353805*sin(2.0*t1 + 3.0*t2 + t3 + t4) + 0.00073318229166666670434948649415219*sin(t2 + t3 + t4) - 0.00036659114583333335217474324707609*sin(t1 - 1.0*t2 + t3 + t4) + 0.00057664973958333336527190549070099*sin(t2 - 2.0*t1 + t3 + t4) + 0.00057664973958333336527190549070099*sin(2.0*t1 + t2 + t3 + t4) + 0.00036659114583333335217474324707609*sin(t1 + 3.0*t2 + t3 + t4) + 0.00018329557291666667608737162353805*sin(2.0*t1 + t2 - 1.0*t3 - 1.0*t4) - 0.00036659114583333335217474324707609*sin(t3 - 1.0*t2 + t4) + 0.00036659114583333335217474324707609*sin(t1 + t2 - 1.0*t3 - 1.0*t4) - 0.00073318229166666670434948649415219*sin(2.0*t1 + t2 - 1.0*t3 + t4) - 0.00018329557291666667608737162353805*sin(2.0*t1 - 1.0*t2 + t3 + t4) - 0.00036659114583333335217474324707609*sin(3.0*t2 + t3 + t4) + 35.125*L3*m5*sin(t2 + t3 + t4 - 1.0*t5) + 0.125*L3^2*m5*sin(t2 + t3 + t4) + 0.0625*L3^2*m5*sin(t2 + t3 + t4 - 2.0*t5) + 0.0625*L3^2*m5*sin(t2 + t3 + t4 + 2.0*t5) + 35.125*L3*m5*sin(t2 + t3 + t4 + t5)) + td4*(0.00073318229166666670434948649415219*sin(t2 - 2.0*t1 + 3.0*t3 + t4) + 0.00073318229166666670434948649415219*sin(2.0*t1 + t2 - 1.0*t3 + t4) - 47.0*L3*m5*sin(t4 - 1.0*t5) - 47.0*L3*m5*sin(t4 + t5) + 0.25*L3^2*m5*cos(t5)*sin(t5) + 94.0*L3*m5*cos(t5)*sin(t4)) + td2*(0.00036659114583333335217474324707609*sin(3.0*t2 - 1.0*t1 + t3 + t4) + 0.00073318229166666670434948649415219*sin(t2 - 2.0*t1 + 3.0*t3 + t4) - 0.00018329557291666667608737162353805*sin(3.0*t2 - 2.0*t1 + t3 + t4) + 0.00018329557291666667608737162353805*sin(2.0*t1 + 3.0*t2 + t3 + t4) - 0.00036659114583333335217474324707609*sin(t1 - 1.0*t2 + t3 + t4) - 0.00036659114583333335217474324707609*sin(t1 + 3.0*t2 + t3 + t4) - 0.00018329557291666667608737162353805*sin(2.0*t1 + t2 - 1.0*t3 - 1.0*t4) - 0.00036659114583333335217474324707609*sin(t1 + t2 - 1.0*t3 - 1.0*t4) + 0.00073318229166666670434948649415219*sin(2.0*t1 + t2 - 1.0*t3 + t4) - 0.00018329557291666667608737162353805*sin(2.0*t1 - 1.0*t2 + t3 + t4) + 102.0*L3*m5*sin(t3 + t4 + t5) + 94.0*L3*m5*sin(t4 - 1.0*t5) + 94.0*L3*m5*sin(t4 + t5) + 102.0*L3*m5*sin(t3 + t4 - 1.0*t5) + 0.125*L3^2*m5*sin(2.0*t5)) + td3*(0.25*m5*cos(t5)*sin(t5)*L3^2 + 188.0*m5*cos(t5)*sin(t4)*L3) - 1.0*td6*(0.00042011718750000002619432448724979*sin(t5) + 0.00042011718750000002619432448724979*cos(t1)^2*sin(t5) + 0.00063017578125000003929148673087468*cos(2.0*t2)*cos(2.0*t3)*cos(2.0*t4)*sin(t5) - 0.00063017578125000003929148673087468*cos(2.0*t2)*sin(2.0*t3)*sin(2.0*t4)*sin(t5) - 0.00063017578125000003929148673087468*cos(2.0*t3)*sin(2.0*t2)*sin(2.0*t4)*sin(t5) - 0.00063017578125000003929148673087468*cos(2.0*t4)*sin(2.0*t2)*sin(2.0*t3)*sin(t5) - 0.00021005859375000001309716224362489*cos(2.0*t1)*cos(2.0*t2)*cos(2.0*t3)*cos(2.0*t4)*sin(t5) + 0.00021005859375000001309716224362489*cos(2.0*t1)*cos(2.0*t2)*sin(2.0*t3)*sin(2.0*t4)*sin(t5) + 0.00021005859375000001309716224362489*cos(2.0*t1)*cos(2.0*t3)*sin(2.0*t2)*sin(2.0*t4)*sin(t5) + 0.00021005859375000001309716224362489*cos(2.0*t1)*cos(2.0*t4)*sin(2.0*t2)*sin(2.0*t3)*sin(t5) - 0.00021005859375000001309716224362489*sin(2.0*t1)*cos(t2)*cos(t3)*cos(t4)*cos(t5) + 0.00021005859375000001309716224362489*sin(2.0*t1)*cos(t2)*cos(t5)*sin(t3)*sin(t4) + 0.00021005859375000001309716224362489*sin(2.0*t1)*cos(t3)*cos(t5)*sin(t2)*sin(t4) + 0.00021005859375000001309716224362489*sin(2.0*t1)*cos(t4)*cos(t5)*sin(t2)*sin(t3) + 0.00042011718750000002619432448724979*cos(t1)*cos(t2)*cos(t3)*cos(t4)*cos(t5)*sin(t1) - 0.00042011718750000002619432448724979*cos(t1)*cos(t2)*cos(t5)*sin(t1)*sin(t3)*sin(t4) - 0.00042011718750000002619432448724979*cos(t1)*cos(t3)*cos(t5)*sin(t1)*sin(t2)*sin(t4) - 0.00042011718750000002619432448724979*cos(t1)*cos(t4)*cos(t5)*sin(t1)*sin(t2)*sin(t3))) + td6*(td6*(0.5*(0.0016804687500000001047772979489991*cos(t1)*cos(t5) - 0.0016804687500000001047772979489991*cos(t2)*cos(t3)*cos(t4)*sin(t1)*sin(t5) + 0.0016804687500000001047772979489991*cos(t2)*sin(t1)*sin(t3)*sin(t4)*sin(t5) + 0.0016804687500000001047772979489991*cos(t3)*sin(t1)*sin(t2)*sin(t4)*sin(t5) + 0.0016804687500000001047772979489991*cos(t4)*sin(t1)*sin(t2)*sin(t3)*sin(t5))*(cos(t2)*cos(t5)*sin(t1)*sin(t3)*sin(t4) - 1.0*cos(t2)*cos(t3)*cos(t4)*cos(t5)*sin(t1) - 1.0*cos(t1)*sin(t5) + cos(t3)*cos(t5)*sin(t1)*sin(t2)*sin(t4) + cos(t4)*cos(t5)*sin(t1)*sin(t2)*sin(t3)) + 0.5*(sin(t1)*sin(t5) - 1.0*cos(t1)*cos(t2)*cos(t3)*cos(t4)*cos(t5) + cos(t1)*cos(t2)*cos(t5)*sin(t3)*sin(t4) + cos(t1)*cos(t3)*cos(t5)*sin(t2)*sin(t4) + cos(t1)*cos(t4)*cos(t5)*sin(t2)*sin(t3))*(0.00084023437500000005238864897449957*cos(t1)*cos(t2)*sin(t3)*sin(t4)*sin(t5) - 0.00084023437500000005238864897449957*cos(t1)*cos(t2)*cos(t3)*cos(t4)*sin(t5) - 0.00084023437500000005238864897449957*cos(t5)*sin(t1) + 0.00084023437500000005238864897449957*cos(t1)*cos(t3)*sin(t2)*sin(t4)*sin(t5) + 0.00084023437500000005238864897449957*cos(t1)*cos(t4)*sin(t2)*sin(t3)*sin(t5)) + 0.5*(0.00084023437500000005238864897449957*sin(t1)*sin(t5) - 0.00084023437500000005238864897449957*cos(t1)*cos(t2)*cos(t3)*cos(t4)*cos(t5) + 0.00084023437500000005238864897449957*cos(t1)*cos(t2)*cos(t5)*sin(t3)*sin(t4) + 0.00084023437500000005238864897449957*cos(t1)*cos(t3)*cos(t5)*sin(t2)*sin(t4) + 0.00084023437500000005238864897449957*cos(t1)*cos(t4)*cos(t5)*sin(t2)*sin(t3))*(cos(t1)*cos(t2)*sin(t3)*sin(t4)*sin(t5) - 1.0*cos(t1)*cos(t2)*cos(t3)*cos(t4)*sin(t5) - 1.0*cos(t5)*sin(t1) + cos(t1)*cos(t3)*sin(t2)*sin(t4)*sin(t5) + cos(t1)*cos(t4)*sin(t2)*sin(t3)*sin(t5)) + 0.5*(0.0016804687500000001047772979489991*cos(t2)*cos(t5)*sin(t1)*sin(t3)*sin(t4) - 0.0016804687500000001047772979489991*cos(t2)*cos(t3)*cos(t4)*cos(t5)*sin(t1) - 0.0016804687500000001047772979489991*cos(t1)*sin(t5) + 0.0016804687500000001047772979489991*cos(t3)*cos(t5)*sin(t1)*sin(t2)*sin(t4) + 0.0016804687500000001047772979489991*cos(t4)*cos(t5)*sin(t1)*sin(t2)*sin(t3))*(cos(t1)*cos(t5) - 1.0*cos(t2)*cos(t3)*cos(t4)*sin(t1)*sin(t5) + cos(t2)*sin(t1)*sin(t3)*sin(t4)*sin(t5) + cos(t3)*sin(t1)*sin(t2)*sin(t4)*sin(t5) + cos(t4)*sin(t1)*sin(t2)*sin(t3)*sin(t5))) + 1.0*td1*(0.00021005859375000001309716224362489*cos(2.0*t2)*cos(2.0*t3)*sin(2.0*t1)*sin(2.0*t4)*sin(t5) + 0.00021005859375000001309716224362489*cos(2.0*t2)*cos(2.0*t4)*sin(2.0*t1)*sin(2.0*t3)*sin(t5) + 0.00021005859375000001309716224362489*cos(2.0*t3)*cos(2.0*t4)*sin(2.0*t1)*sin(2.0*t2)*sin(t5) - 0.00042011718750000002619432448724979*cos(2.0*t1)*cos(t2)*cos(t3)*cos(t5)*sin(t4) - 0.00042011718750000002619432448724979*cos(2.0*t1)*cos(t2)*cos(t4)*cos(t5)*sin(t3) - 0.00042011718750000002619432448724979*cos(2.0*t1)*cos(t3)*cos(t4)*cos(t5)*sin(t2) - 0.00021005859375000001309716224362489*sin(2.0*t1)*sin(2.0*t2)*sin(2.0*t3)*sin(2.0*t4)*sin(t5) + 0.00042011718750000002619432448724979*cos(2.0*t1)*cos(t5)*sin(t2)*sin(t3)*sin(t4)) + td2*(0.00063017578125000003929148673087468*cos(2.0*t2)*cos(2.0*t3)*cos(2.0*t4)*sin(t5) - 0.00042011718750000002619432448724979*cos(t1)^2*sin(t5) - 0.00042011718750000002619432448724979*sin(t5) - 0.00063017578125000003929148673087468*cos(2.0*t2)*sin(2.0*t3)*sin(2.0*t4)*sin(t5) - 0.00063017578125000003929148673087468*cos(2.0*t3)*sin(2.0*t2)*sin(2.0*t4)*sin(t5) - 0.00063017578125000003929148673087468*cos(2.0*t4)*sin(2.0*t2)*sin(2.0*t3)*sin(t5) - 0.00021005859375000001309716224362489*cos(2.0*t1)*cos(2.0*t2)*cos(2.0*t3)*cos(2.0*t4)*sin(t5) + 0.00021005859375000001309716224362489*cos(2.0*t1)*cos(2.0*t2)*sin(2.0*t3)*sin(2.0*t4)*sin(t5) + 0.00021005859375000001309716224362489*cos(2.0*t1)*cos(2.0*t3)*sin(2.0*t2)*sin(2.0*t4)*sin(t5) + 0.00021005859375000001309716224362489*cos(2.0*t1)*cos(2.0*t4)*sin(2.0*t2)*sin(2.0*t3)*sin(t5) - 0.00021005859375000001309716224362489*sin(2.0*t1)*cos(t2)*cos(t3)*cos(t4)*cos(t5) + 0.00021005859375000001309716224362489*sin(2.0*t1)*cos(t2)*cos(t5)*sin(t3)*sin(t4) + 0.00021005859375000001309716224362489*sin(2.0*t1)*cos(t3)*cos(t5)*sin(t2)*sin(t4) + 0.00021005859375000001309716224362489*sin(2.0*t1)*cos(t4)*cos(t5)*sin(t2)*sin(t3) - 0.00042011718750000002619432448724979*cos(t1)*cos(t2)*cos(t3)*cos(t4)*cos(t5)*sin(t1) + 0.00042011718750000002619432448724979*cos(t1)*cos(t2)*cos(t5)*sin(t1)*sin(t3)*sin(t4) + 0.00042011718750000002619432448724979*cos(t1)*cos(t3)*cos(t5)*sin(t1)*sin(t2)*sin(t4) + 0.00042011718750000002619432448724979*cos(t1)*cos(t4)*cos(t5)*sin(t1)*sin(t2)*sin(t3)) + td3*(0.00063017578125000003929148673087468*cos(2.0*t2)*cos(2.0*t3)*cos(2.0*t4)*sin(t5) - 0.00042011718750000002619432448724979*cos(t1)^2*sin(t5) - 0.00042011718750000002619432448724979*sin(t5) - 0.00063017578125000003929148673087468*cos(2.0*t2)*sin(2.0*t3)*sin(2.0*t4)*sin(t5) - 0.00063017578125000003929148673087468*cos(2.0*t3)*sin(2.0*t2)*sin(2.0*t4)*sin(t5) - 0.00063017578125000003929148673087468*cos(2.0*t4)*sin(2.0*t2)*sin(2.0*t3)*sin(t5) - 0.00021005859375000001309716224362489*cos(2.0*t1)*cos(2.0*t2)*cos(2.0*t3)*cos(2.0*t4)*sin(t5) + 0.00021005859375000001309716224362489*cos(2.0*t1)*cos(2.0*t2)*sin(2.0*t3)*sin(2.0*t4)*sin(t5) + 0.00021005859375000001309716224362489*cos(2.0*t1)*cos(2.0*t3)*sin(2.0*t2)*sin(2.0*t4)*sin(t5) + 0.00021005859375000001309716224362489*cos(2.0*t1)*cos(2.0*t4)*sin(2.0*t2)*sin(2.0*t3)*sin(t5) - 0.00021005859375000001309716224362489*sin(2.0*t1)*cos(t2)*cos(t3)*cos(t4)*cos(t5) + 0.00021005859375000001309716224362489*sin(2.0*t1)*cos(t2)*cos(t5)*sin(t3)*sin(t4) + 0.00021005859375000001309716224362489*sin(2.0*t1)*cos(t3)*cos(t5)*sin(t2)*sin(t4) + 0.00021005859375000001309716224362489*sin(2.0*t1)*cos(t4)*cos(t5)*sin(t2)*sin(t3) - 0.00042011718750000002619432448724979*cos(t1)*cos(t2)*cos(t3)*cos(t4)*cos(t5)*sin(t1) + 0.00042011718750000002619432448724979*cos(t1)*cos(t2)*cos(t5)*sin(t1)*sin(t3)*sin(t4) + 0.00042011718750000002619432448724979*cos(t1)*cos(t3)*cos(t5)*sin(t1)*sin(t2)*sin(t4) + 0.00042011718750000002619432448724979*cos(t1)*cos(t4)*cos(t5)*sin(t1)*sin(t2)*sin(t3)) + td4*(0.00063017578125000003929148673087468*cos(2.0*t2)*cos(2.0*t3)*cos(2.0*t4)*sin(t5) - 0.00042011718750000002619432448724979*cos(t1)^2*sin(t5) - 0.00042011718750000002619432448724979*sin(t5) - 0.00063017578125000003929148673087468*cos(2.0*t2)*sin(2.0*t3)*sin(2.0*t4)*sin(t5) - 0.00063017578125000003929148673087468*cos(2.0*t3)*sin(2.0*t2)*sin(2.0*t4)*sin(t5) - 0.00063017578125000003929148673087468*cos(2.0*t4)*sin(2.0*t2)*sin(2.0*t3)*sin(t5) - 0.00021005859375000001309716224362489*cos(2.0*t1)*cos(2.0*t2)*cos(2.0*t3)*cos(2.0*t4)*sin(t5) + 0.00021005859375000001309716224362489*cos(2.0*t1)*cos(2.0*t2)*sin(2.0*t3)*sin(2.0*t4)*sin(t5) + 0.00021005859375000001309716224362489*cos(2.0*t1)*cos(2.0*t3)*sin(2.0*t2)*sin(2.0*t4)*sin(t5) + 0.00021005859375000001309716224362489*cos(2.0*t1)*cos(2.0*t4)*sin(2.0*t2)*sin(2.0*t3)*sin(t5) - 0.00021005859375000001309716224362489*sin(2.0*t1)*cos(t2)*cos(t3)*cos(t4)*cos(t5) + 0.00021005859375000001309716224362489*sin(2.0*t1)*cos(t2)*cos(t5)*sin(t3)*sin(t4) + 0.00021005859375000001309716224362489*sin(2.0*t1)*cos(t3)*cos(t5)*sin(t2)*sin(t4) + 0.00021005859375000001309716224362489*sin(2.0*t1)*cos(t4)*cos(t5)*sin(t2)*sin(t3) - 0.00042011718750000002619432448724979*cos(t1)*cos(t2)*cos(t3)*cos(t4)*cos(t5)*sin(t1) + 0.00042011718750000002619432448724979*cos(t1)*cos(t2)*cos(t5)*sin(t1)*sin(t3)*sin(t4) + 0.00042011718750000002619432448724979*cos(t1)*cos(t3)*cos(t5)*sin(t1)*sin(t2)*sin(t4) + 0.00042011718750000002619432448724979*cos(t1)*cos(t4)*cos(t5)*sin(t1)*sin(t2)*sin(t3))) + td2*(td2*(0.25*L3^2*m5*cos(t5)*sin(t5) + 188.0*L3*m5*cos(t5)*sin(t4) + 204.0*L3*m5*cos(t3)*cos(t5)*sin(t4) + 204.0*L3*m5*cos(t4)*cos(t5)*sin(t3)) - 1.0*td1*(0.00073318229166666670434948649415219*sin(3.0*t2 - 1.0*t1 + t3 + t4) - 0.00073318229166666670434948649415219*sin(t2 - 2.0*t1 + 3.0*t3 + t4) - 0.00018329557291666667608737162353805*sin(3.0*t2 - 2.0*t1 + t3 + t4) - 0.00018329557291666667608737162353805*sin(2.0*t1 + 3.0*t2 + t3 + t4) + 0.00073318229166666670434948649415219*sin(t2 + t3 + t4) + 0.00057664973958333336527190549070099*sin(t2 - 2.0*t1 + t3 + t4) + 0.00057664973958333336527190549070099*sin(2.0*t1 + t2 + t3 + t4) + 0.00073318229166666670434948649415219*sin(t1 + 3.0*t2 + t3 + t4) + 0.00018329557291666667608737162353805*sin(2.0*t1 + t2 - 1.0*t3 - 1.0*t4) + 0.00036659114583333335217474324707609*sin(t3 - 1.0*t2 + t4) - 0.00073318229166666670434948649415219*sin(2.0*t1 + t2 - 1.0*t3 + t4) - 0.00018329557291666667608737162353805*sin(2.0*t1 - 1.0*t2 + t3 + t4) - 0.0010997734375000000565242297412283*sin(3.0*t2 + t3 + t4) + 35.125*L3*m5*sin(t2 + t3 + t4 - 1.0*t5) + 0.125*L3^2*m5*sin(t2 + t3 + t4) + 0.0625*L3^2*m5*sin(t2 + t3 + t4 - 2.0*t5) + 0.0625*L3^2*m5*sin(t2 + t3 + t4 + 2.0*t5) + 35.125*L3*m5*sin(t2 + t3 + t4 + t5)) + td4*(0.125*m5*sin(2.0*t5)*L3^2 - 0.00036659114583333335217474324707609*sin(3.0*t2 - 1.0*t1 + t3 + t4) + 0.00018329557291666667608737162353805*sin(3.0*t2 - 2.0*t1 + t3 + t4) - 0.00018329557291666667608737162353805*sin(2.0*t1 + 3.0*t2 + t3 + t4) + 0.00036659114583333335217474324707609*sin(t1 - 1.0*t2 + t3 + t4) + 0.00036659114583333335217474324707609*sin(t1 + 3.0*t2 + t3 + t4) + 0.00018329557291666667608737162353805*sin(2.0*t1 + t2 - 1.0*t3 - 1.0*t4) + 0.00036659114583333335217474324707609*sin(t1 + t2 - 1.0*t3 - 1.0*t4) + 0.00018329557291666667608737162353805*sin(2.0*t1 - 1.0*t2 + t3 + t4)) + td5*(0.00036659114583333335217474324707609*sin(2.0*t1 + 2.0*t2 + 2.0*t4) + 0.001729949218750000095815716472103*sin(2.0*t2 + 2.0*t3 + 2.0*t4) + 0.0010997734375000000565242297412283*sin(4.0*t2 + 2.0*t3 + 2.0*t4) - 0.00073318229166666670434948649415219*sin(4.0*t2 - 1.0*t1 + 2.0*t3 + 2.0*t4) - 0.00028832486979166668263595274535049*sin(2.0*t2 - 2.0*t1 + 2.0*t3 + 2.0*t4) - 0.00028832486979166668263595274535049*sin(2.0*t1 + 2.0*t2 + 2.0*t3 + 2.0*t4) + 0.00036659114583333335217474324707609*sin(2.0*t2 - 2.0*t1 + 4.0*t3 + 2.0*t4) + 0.00018329557291666667608737162353805*sin(4.0*t2 - 2.0*t1 + 2.0*t3 + 2.0*t4) + 0.00018329557291666667608737162353805*sin(2.0*t1 + 4.0*t2 + 2.0*t3 + 2.0*t4) - 0.00073318229166666670434948649415219*sin(t1 + 4.0*t2 + 2.0*t3 + 2.0*t4) + 0.00036659114583333335217474324707609*sin(2.0*t2) + 0.00018329557291666667608737162353805*sin(2.0*t1 - 2.0*t2) - 0.00018329557291666667608737162353805*sin(2.0*t1 + 2.0*t2)) + td3*(0.00018329557291666667608737162353805*sin(3.0*t2 - 2.0*t1 + t3 + t4) - 0.00073318229166666670434948649415219*sin(t2 - 2.0*t1 + 3.0*t3 + t4) - 0.00036659114583333335217474324707609*sin(3.0*t2 - 1.0*t1 + t3 + t4) - 0.00018329557291666667608737162353805*sin(2.0*t1 + 3.0*t2 + t3 + t4) + 0.00036659114583333335217474324707609*sin(t1 - 1.0*t2 + t3 + t4) + 0.00036659114583333335217474324707609*sin(t1 + 3.0*t2 + t3 + t4) + 0.00018329557291666667608737162353805*sin(2.0*t1 + t2 - 1.0*t3 - 1.0*t4) + 0.00036659114583333335217474324707609*sin(t1 + t2 - 1.0*t3 - 1.0*t4) - 0.00073318229166666670434948649415219*sin(2.0*t1 + t2 - 1.0*t3 + t4) + 0.00018329557291666667608737162353805*sin(2.0*t1 - 1.0*t2 + t3 + t4) + 94.0*L3*m5*sin(t4 - 1.0*t5) + 94.0*L3*m5*sin(t4 + t5) + 0.125*L3^2*m5*sin(2.0*t5)) - 1.0*td6*(0.00042011718750000002619432448724979*sin(t5) + 0.00042011718750000002619432448724979*cos(t1)^2*sin(t5) + 0.00063017578125000003929148673087468*cos(2.0*t2)*cos(2.0*t3)*cos(2.0*t4)*sin(t5) - 0.00063017578125000003929148673087468*cos(2.0*t2)*sin(2.0*t3)*sin(2.0*t4)*sin(t5) - 0.00063017578125000003929148673087468*cos(2.0*t3)*sin(2.0*t2)*sin(2.0*t4)*sin(t5) - 0.00063017578125000003929148673087468*cos(2.0*t4)*sin(2.0*t2)*sin(2.0*t3)*sin(t5) - 0.00021005859375000001309716224362489*cos(2.0*t1)*cos(2.0*t2)*cos(2.0*t3)*cos(2.0*t4)*sin(t5) + 0.00021005859375000001309716224362489*cos(2.0*t1)*cos(2.0*t2)*sin(2.0*t3)*sin(2.0*t4)*sin(t5) + 0.00021005859375000001309716224362489*cos(2.0*t1)*cos(2.0*t3)*sin(2.0*t2)*sin(2.0*t4)*sin(t5) + 0.00021005859375000001309716224362489*cos(2.0*t1)*cos(2.0*t4)*sin(2.0*t2)*sin(2.0*t3)*sin(t5) - 0.00021005859375000001309716224362489*sin(2.0*t1)*cos(t2)*cos(t3)*cos(t4)*cos(t5) + 0.00021005859375000001309716224362489*sin(2.0*t1)*cos(t2)*cos(t5)*sin(t3)*sin(t4) + 0.00021005859375000001309716224362489*sin(2.0*t1)*cos(t3)*cos(t5)*sin(t2)*sin(t4) + 0.00021005859375000001309716224362489*sin(2.0*t1)*cos(t4)*cos(t5)*sin(t2)*sin(t3) + 0.00042011718750000002619432448724979*cos(t1)*cos(t2)*cos(t3)*cos(t4)*cos(t5)*sin(t1) - 0.00042011718750000002619432448724979*cos(t1)*cos(t2)*cos(t5)*sin(t1)*sin(t3)*sin(t4) - 0.00042011718750000002619432448724979*cos(t1)*cos(t3)*cos(t5)*sin(t1)*sin(t2)*sin(t4) - 0.00042011718750000002619432448724979*cos(t1)*cos(t4)*cos(t5)*sin(t1)*sin(t2)*sin(t3)))
